simulink library "Centralized_I_Lib_Controller"  (R2024b)
(part 3 of 7)

[dq1,dq2,dq3,dq4,dq5,dq6,t10,t100,t1001,t1002,t1003,t1004,t1005,t1006,t1007,t1009,t101,t1010,t1011,t1013,t1016,t1018,t1019,t102,t1022,t1023,t1025,t1027,t1029,t1030,t1033,t1034,t1035,t1037,t1039,t104,t1041,t1042,t1043,t1047,t1048,t105,t1050,t1051,t1053,t1055,t1056,t1058,t1059,t106,t1060,t1061,t1062,t1063,t1065,t1067,t1068,t107,t1072,t1073,t1074,t1076,t1077,t1078,t108,t1080,t1081,t1082,t1083,t1084,t1085,t1086,t1087,t1088,t1089,t109,t1090,t1091,t1092,t1095,t1096,t1098,t1099,t11,t110,t1100,t1101,t1102,t1103,t1104,t1105,t1106,t1107,t1108,t111,t1110,t1111,t1112,t1113,t1114,t1116,t1117,t1119,t112,t1120,t1122,t1123,t1124,t1127,t113,t1131,t1132,t1133,t1134,t1135,t114,t1141,t1144,t1145,t1147,t1148,t1149,t1151,t1158,t1159,t116,t1160,t1161,t1162,t1163,t1164,t1165,t1166,t1167,t1169,t1170,t1171,t1172,t1173,t1176,t1177,t1178,t118,t1180,t1182,t1183,t1186,t1188,t1189,t119,t1190,t1191,t1192,t1193,t1194,t1195,t1196,t1198,t1199,t12,t120,t1201,t1202,t1203,t1204,t1205,t1207,t1208,t1210,t1211,t1212,t1214,t1215,t1216,t1217,t1218,t1219,t1220,t1221,t1222,t1224,t1227,t1228,t1229,t123,t1230,t1231,t1233,t1234,t1235,t1239,t124,t1240,t1241,t1242,t1243,t1244,t1245,t1246,t1247,t125,t1254,t1255,t1256,t126,t1263,t1266,t127,t128,t1283,t1286,t1287,t1288,t1289,t129,t1291,t1293,t1295,t1296,t1297,t1298,t1299,t13,t130,t131,t1316,t1317,t1319,t132,t1320,t1323,t1324,t1325,t1326,t1327,t1328,t1329,t133,t1331,t1332,t1333,t1334,t1335,t1345,t1346,t1347,t1349,t135,t1352,t1353,t1355,t1356,t1357,t1358,t1359,t1361,t1362,t1363,t1366,t1369,t137,t1370,t1371,t1372,t1373,t1375,t1376,t1377,t1379,t138,t1380,t1383,t1385,t1386,t1387,t1388,t139,t1390,t1391,t1392,t1393,t1395,t1397,t1398,t1399,t140,t1400,t1401,t1402,t1403,t1404,t1406,t1407,t1408,t1409,t141,t1410,t1413,t1416,t1417,t1419,t142,t1423,t1424,t1426,t1427,t1429,t143,t1432,t1433,t1434,t1435,t1438,t1441,t1442,t1443,t1445,t1447,t1450,t1452,t1453,t1456,t1457,t1458,t1462,t1463,t1464,t1465,t1466,t1467,t1468,t1469,t1470,t1473,t1475,t1476,t1477,t1479,t1480,t1481,t1482,t1483,t1484,t1487,t1488,t1489,t1490,t1491,t1493,t1494,t1495,t1496,t1497,t1498,t1499,t1500,t1502,t1503,t1504,t1505,t1511,t1513,t1523,t1524,t1525,t1526,t1528,t1530,t1531,t1532,t1533,t1534,t1536,t1537,t1538,t1539,t1540,t1541,t1544,t1545,t1546,t1554,t1555,t1556,t1557,t1558,t1562,t1563,t1564,t1566,t1567,t1568,t1571,t1575,t1576,t158,t1581,t1582,t1584,t1585,t1586,t1587,t1589,t159,t1590,t1591,t1592,t1593,t1595,t1597,t1598,t1599,t160,t1600,t1601,t1602,t1603,t1604,t1605,t1606,t1607,t1608,t1609,t161,t1610,t1611,t1612,t1613,t1614,t1618,t1619,t162,t1620,t1621,t1623,t1624,t1626,t1627,t1628,t1629,t163,t1630,t1631,t1632,t1633,t1634,t1635,t1637,t164,t1643,t165,t1654,t1655,t1656,t1657,t166,t1660,t1661,t1662,t1663,t1664,t1665,t1666,t1668,t1669,t167,t1670,t1671,t1673,t1675,t1676,t1677,t168,t1681,t1682,t1684,t1685,t1686,t1688,t1689,t1690,t1691,t1692,t1695,t1696,t1697,t1698,t170,t1700,t1701,t1702,t1703,t1704,t1705,t1706,t1709,t171,t1711,t1713,t1714,t1715,t1716,t1717,t1718,t1719,t1720,t1721,t1722,t1723,t1724,t1726,t1727,t1728,t173,t1730,t1732,t1734,t1736,t1739,t1741,t1742,t1747,t1748,t1749,t1750,t1752,t1753,t1754,t1755,t1756,t1758,t1759,t1760,t1761,t1763,t1764,t1765,t1766,t1767,t1768,t177,t1772,t1773,t1776,t1778,t1779,t178,t1780,t1781,t1782,t1785,t1786,t1787,t179,t1794,t1796,t18,t180,t1800,t1801,t1802,t1803,t1804,t1805,t1806,t1808,t181,t1815,t1816,t1817,t1818,t1819,t182,t1820,t1821,t1822,t1823,t1827,t1828,t1829,t183,t1830,t1831,t1832,t1833,t1837,t1838,t1839,t184,t1840,t1844,t1845,t1847,t1849,t185,t1850,t1851,t1852,t1853,t1854,t1857,t1858,t1859,t186,t1860,t1861,t1862,t1866,t1867,t1868,t1869,t187,t1870,t1871,t1872,t1873,t1874,t1875,t1876,t1877,t1878,t1879,t188,t1881,t1882,t1883,t1884,t1885,t1888,t1889,t189,t1890,t1893,t1895,t1896,t1897,t1898,t1899,t19,t1900,t1901,t1902,t1904,t1906,t1907,t191,t1911,t1913,t1917,t1919,t192,t1921,t1922,t1923,t1925,t1926,t1927,t193,t1931,t1936,t1937,t194,t1943,t1944,t1947,t1949,t195,t1950,t1952,t1953,t1954,t1955,t1956,t1957,t1958,t1959,t1962,t1964,t1965,t1966,t1967,t1970,t1971,t1973,t1974,t1975,t1976,t1977,t1978,t1980,t1981,t1982,t1983,t1984,t1985,t1986,t1987,t1988,t1990,t1991,t1992,t1993,t1994,t1997,t2,t20,t200,t2001,t2002,t2003,t2004,t2005,t2007,t2009,t201,t2010,t2014,t2015,t2017,t2018,t202,t2021,t2023,t2024,t2025,t2029,t203,t2030,t2031,t2034,t2035,t2036,t2037,t2038,t2039,t204,t2040,t2041,t2043,t2046,t2047,t2048,t2050,t2052,t2053,t2054,t2055,t2056,t2057,t2058,t2059,t206,t2061,t2063,t2064,t2065,t2066,t2067,t2068,t2069,t2070,t2071,t2072,t2073,t2075,t2077,t2078,t208,t2080,t2081,t2083,t2084,t2085,t2086,t2087,t2089,t209,t2090,t2091,t2092,t2093,t2094,t2096,t2097,t2098,t2099,t21,t210,t2106,t211,t2111,t2112,t2115,t2118,t212,t2121,t2124,t2125,t2126,t2128,t213,t2132,t2134,t2135,t2136,t2137,t2138,t2139,t214,t2140,t2141,t2144,t2145,t2148,t215,t2152,t2154,t2156,t2157,t2158,t2159,t216,t2160,t2161,t2162,t2163,t2165,t2167,t2169,t217,t2171,t2172,t2175,t2176,t2177,t2178,t2179,t218,t2180,t2181,t2182,t2183,t2184,t2185,t2186,t2187,t2188,t2189,t219,t2190,t2191,t2193,t2196,t2197,t2198,t2199,t22,t220,t2201,t2203,t2204,t2205,t2206,t2208,t221,t2212,t2213,t2214,t2215,t2216,t2217,t2219,t222,t2221,t2222,t2223,t2224,t2225,t2226,t2227,t2229,t223,t2231,t2232,t2233,t2235,t2236,t2237,t2238,t2239,t224,t2240,t2242,t2243,t2245,t2246,t2247,t2248,t2249,t225,t2250,t2251,t2252,t2253,t2254,t2256,t2258,t2259,t226,t2263,t2264,t2265,t2266,t2267,t2268,t2269,t227,t2277,t2278,t228,t2281,t2282,t2283,t2284,t2285,t2287,t2289,t229,t2290,t2292,t2293,t2296,t2297,t2299,t230,t2300,t2301,t231,t2310,t2312,t2313,t2314,t2319,t2322,t2323,t2324,t2326,t2327,t2329,t2330,t2331,t2332,t2333,t2334,t2338,t2339,t234,t2342,t2343,t2344,t235,t2356,t2357,t2358,t236,t2362,t2363,t2364,t2365,t2368,t2369,t237,t2370,t2371,t2372,t2374,t2376,t2378,t2379,t238,t2381,t2382,t2383,t2386,t2387,t239,t2390,t2391,t2392,t2394,t2395,t2396,t2397,t2398,t240,t2400,t2401,t2402,t2403,t2405,t2408,t2409,t241,t2410,t2412,t2413,t2414,t2416,t2417,t2418,t2419,t242,t2421,t2422,t2423,t2424,t2425,t2426,t2427,t2428,t2429,t243,t2430,t2431,t2432,t2433,t2436,t2437,t2438,t2439,t244,t2440,t2449,t245,t2450,t2451,t2452,t2453,t2454,t2455,t2456,t2457,t2459,t246,t2464,t2465,t2466,t2467,t2468,t2469,t247,t2470,t2471,t2472,t2473,t2474,t2475,t2476,t2477,t2478,t2479,t248,t2481,t2482,t2483,t2484,t2485,t2486,t2487,t2488,t249,t2491,t2492,t2494,t2495,t2496,t2498,t25,t250,t2504,t2508,t251,t2511,t2512,t2513,t2514,t2515,t2516,t2517,t2518,t252,t2520,t2523,t2524,t2525,t2527,t2529,t253,t2531,t2534,t2536,t2537,t2538,t2541,t2542,t2546,t2547,t2548,t255,t2550,t2552,t2553,t2554,t2555,t2556,t2557,t2559,t256,t2560,t2563,t2564,t2565,t2566,t2567,t2568,t2569,t2570,t2571,t2572,t2573,t2574,t2575,t2576,t2577,t2578,t2579,t2580,t2581,t2582,t2583,t2585,t2586,t2587,t2588,t259,t2591,t2593,t2594,t2595,t2596,t2597,t2598,t2599,t26,t260,t2600,t2601,t2602,t2603,t2604,t2605,t2607,t2608,t2609,t261,t2610,t2611,t2614,t2615,t2616,t2617,t262,t2622,t2623,t2625,t2628,t2629,t263,t2631,t2632,t2634,t2636,t2638,t2644,t2646,t2649,t265,t2650,t2652,t2659,t2660,t2661,t2665,t2666,t2667,t2668,t2669,t267,t2670,t2671,t2672,t2673,t2674,t2675,t2679,t2681,t2682,t2683,t2685,t2686,t2689,t269,t2692,t2694,t2696,t2697,t2698,t27,t270,t2700,t2701,t2702,t2703,t2705,t2706,t2707,t2711,t272,t2723,t2724,t2725,t2726,t2727,t2729,t273,t2730,t2731,t2732,t2733,t2734,t2735,t2736,t2738,t2739,t274,t2740,t2741,t2742,t2744,t2745,t2746,t2747,t2748,t2749,t275,t2751,t2752,t2753,t2754,t2755,t2756,t2757,t2758,t2759,t276,t2762,t2763,t2764,t2765,t2766,t2767,t2769,t277,t2770,t2771,t2776,t2778,t2779,t278,t2780,t2782,t2784,t2785,t2786,t2788,t279,t2792,t2793,t2795,t28,t280,t2800,t2802,t2803,t2804,t2806,t2807,t2809,t281,t2810,t2812,t2813,t2814,t2815,t2819,t2820,t2821,t2822,t2825,t2827,t2828,t2829,t283,t2830,t2832,t2833,t2834,t2836,t2839,t284,t2842,t2843,t2844,t285,t2850,t2854,t2858,t286,t2860,t2862,t2864,t2865,t2866,t2867,t2869,t287,t2870,t2871,t2872,t2873,t2877,t288,t2880,t2882,t2883,t2885,t2887,t2888,t289,t2890,t2891,t2892,t2899,t29,t290,t2900,t2901,t2902,t2903,t2904,t2905,t2906,t2911,t2912,t2913,t2916,t2919,t292,t2921,t2922,t2923,t2924,t2925,t2926,t2927,t2928,t2929,t293,t2930,t2931,t2932,t2933,t2934,t2935,t2937,t2938,t2939,t294,t2940,t2942,t2943,t2944,t2945,t2946,t2947,t2948,t2949,t295,t2950,t2951,t2952,t2953,t2954,t2956,t2957,t2959,t296,t2960,t2962,t2964,t2965,t2966,t2967,t2968,t297,t2970,t2973,t2974,t2975,t2977,t2978,t2979,t298,t2981,t2983,t2984,t2986,t2988,t299,t2991,t2995,t2997,t2998,t3,t300,t3002,t3003,t3004,t3006,t3007,t301,t3010,t3011,t3012,t3013,t3015,t3016,t3017,t302,t3020,t3021,t3023,t3025,t3028,t303,t3034,t3035,t3036,t3037,t304,t3040,t3042,t3046,t3047,t3049,t305,t3051,t3052,t3053,t3054,t3056,t3057,t3058,t3059,t306,t3060,t3061,t3062,t3064,t3065,t3066,t3067,t3068,t3069,t307,t3070,t3071,t3072,t3073,t3074,t3075,t3076,t3077,t3078,t3079,t308,t3080,t3081,t3082,t3083,t3085,t3087,t3088,t309,t3091,t3092,t3093,t3094,t3095,t3096,t3097,t3099,t3100,t3101,t3102,t3103,t3104,t3107,t3108,t3109,t311,t3110,t3111,t3112,t3118,t312,t3126,t3128,t313,t3131,t3132,t3133,t3134,t3135,t3138,t3139,t314,t3140,t3142,t3143,t3146,t3147,t3148,t315,t3156,t316,t3160,t3161,t3162,t3163,t3164,t3167,t3168,t317,t3170,t3175,t318,t3182,t3185,t3187,t3188,t3189,t319,t3190,t3192,t3193,t3196,t3197,t3198,t3199,t320,t3200,t3203,t3204,t3205,t3206,t3207,t3208,t3209,t321,t3210,t3211,t3212,t3213,t3214,t3215,t3216,t3217,t3218,t3219,t322,t3220,t3221,t3222,t3223,t3224,t3225,t3226,t3227,t3228,t323,t3230,t3231,t3232,t3234,t324,t3245,t3246,t325,t326,t3262,t327,t3272,t328,t329,t3298,t3299,t330,t331,t332,t3320,t3326,t333,t3330,t334,t336,t337,t338,t3388,t339,t3396,t341,t342,t343,t344,t345,t3453,t346,t347,t3470,t3471,t3473,t3479,t348,t3480,t3483,t3484,t3485,t3486,t349,t3490,t3491,t3497,t3498,t350,t3501,t3510,t3511,t352,t3521,t3526,t3527,t3528,t3529,t353,t354,t3546,t3547,t3549,t355,t3551,t3559,t356,t3560,t3562,t357,t358,t3589,t3590,t3592,t3593,t3594,t3595,t360,t3608,t3609,t3611,t3612,t3613,t3614,t3615,t3616,t3617,t3627,t3628,t3629,t3630,t3635,t3636,t3637,t364,t3648,t365,t3650,t3651,t367,t368,t3680,t3687,t3690,t3691,t3692,t3704,t3705,t371,t3722,t3723,t3724,t3725,t3726,t373,t375,t376,t377,t3779,t378,t379,t3796,t380,t381,t3811,t382,t3822,t3823,t3824,t3827,t3828,t383,t3839,t384,t385,t386,t3862,t3865,t3868,t387,t3871,t3872,t388,t3884,t389,t3909,t391,t3910,t392,t3932,t3935,t3941,t396,t3960,t3963,t397,t399,t4,t400,t401,t402,t4031,t404,t4042,t4043,t4046,t4047,t405,t4057,t406,t4060,t4061,t4067,t407,t4075,t408,t409,t410,t4103,t4109,t411,t412,t413,t414,t415,t416,t4168,t417,t4174,t418,t419,t420,t4204,t4208,t4209,t421,t4212,t422,t423,t424,t425,t426,t4260,t4261,t4262,t4263,t4265,t427,t4280,t429,t430,t431,t432,t433,t434,t4344,t4345,t4347,t435,t436,t437,t4372,t438,t439,t440,t441,t442,t443,t444,t4451,t4452,t4456,t4457,t4475,t4477,t4478,t450,t4508,t451,t453,t4539,t454,t4542,t4544,t4545,t4546,t4547,t456,t4565,t4566,t4568,t4579,t458,t4581,t4584,t459,t460,t461,t462,t463,t464,t465,t467,t468,t469,t470,t471,t472,t473,t474,t475,t476,t4763,t4765,t4766,t4768,t4769,t477,t4770,t4771,t4773,t478,t479,t48,t480,t4806,t4808,t481,t482,t483,t4830,t4831,t4833,t484,t486,t487,t488,t489,t4895,t4898,t49,t490,t4900,t491,t492,t494,t495,t496,t497,t498,t499,t5,t50,t500,t501,t502,t5041,t5054,t5055,t509,t51,t510,t5103,t511,t512,t513,t514,t515,t516,t517,t5175,t5176,t518,t519,t52,t520,t521,t522,t523,t524,t527,t528,t5280,t529,t53,t530,t531,t534,t5343,t5344,t535,t5354,t5356,t536,t5361,t539,t54,t540,t5411,t542,t543,t545,t546,t547,t548,t5491,t5492,t55,t550,t551,t552,t553,t5551,t5552,t556,t557,t558,t559,t56,t560,t561,t5613,t562,t563,t565,t566,t567,t569,t57,t574,t58,t582,t585,t589,t59,t590,t592,t594,t595,t597,t598,t599,t6,t60,t600,t601,t602,t6023,t604,t605,t606,t608,t609,t61,t610,t611,t613,t614,t616,t617,t62,t624,t63,t630,t632,t635,t636,t641,t643,t644,t645,t647,t6473,t648,t649,t650,t651,t652,t653,t654,t655,t656,t657,t658,t66,t660,t661,t663,t664,t666,t667,t669,t67,t670,t6734,t6735,t6736,t674,t6742,t6743,t6744,t6745,t675,t6754,t6755,t676,t677,t6772,t678,t679,t680,t681,t683,t684,t685,t686,t687,t688,t689,t690,t691,t692,t693,t696,t699,t7,t700,t702,t703,t704,t705,t706,t708,t711,t713,t715,t716,t717,t719,t720,t721,t722,t723,t725,t726,t729,t731,t732,t734,t737,t738,t742,t744,t748,t750,t751,t754,t756,t758,t759,t761,t763,t766,t767,t768,t769,t770,t773,t774,t775,t776,t781,t782,t784,t785,t788,t789,t790,t793,t795,t796,t798,t799,t8,t800,t803,t805,t807,t808,t809,t81,t814,t815,t816,t817,t819,t82,t820,t821,t822,t823,t824,t826,t828,t829,t83,t831,t832,t833,t834,t835,t837,t838,t839,t84,t842,t844,t847,t848,t849,t85,t850,t851,t852,t853,t854,t858,t859,t86,t861,t863,t864,t867,t868,t87,t871,t872,t875,t879,t88,t880,t883,t884,t885,t886,t888,t89,t890,t891,t894,t895,t896,t897,t898,t899,t9,t90,t900,t902,t905,t906,t907,t908,t909,t910,t911,t912,t913,t914,t915,t916,t918,t919,t92,t920,t921,t923,t926,t928,t929,t93,t930,t931,t933,t934,t935,t936,t937,t938,t944,t945,t946,t947,t948,t949,t95,t950,t951,t954,t955,t956,t957,t958,t959,t96,t960,t961,t962,t963,t964,t965,t966,t967,t968,t969,t97,t970,t972,t973,t974,t975,t976,t977,t978,t98,t981,t982,t984,t986,t987,t988,t99,t990,t991,t992,t993,t994,t996,t997,t999] = ct{:};
t3240 = t12.*t204.*2.98328125e-2;
t3241 = t58.*t127.*2.98328125e-2;
t3247 = t28.*t2223;
t3249 = t28.*t2225;
t3250 = t28.*t2226;
t3251 = t22.*t2232;
t3252 = t22.*t2233;
t3257 = t58.*t86.*2.98328125e-2;
t3258 = t7.*t13.*t20.*t97.*1.1015625e-2;
t3260 = t98.*t1867;
t3271 = t22.*t62.*t97.*1.1015625e-2;
t3273 = t7.*t13.*t19.*t111.*1.1015625e-2;
t3274 = t7.*t13.*t20.*t109.*1.1015625e-2;
t3275 = t7.*t13.*t20.*t110.*1.1015625e-2;
t3276 = t6.*t12.*t19.*t101.*1.865e-2;
t3277 = t6.*t12.*t19.*t102.*1.865e-2;
t3279 = t20.*t62.*t97.*1.865e-2;
t3283 = t12.*t194.*t1009;
t3284 = t58.*t111.*t1009;
t3286 = t58.*t113.*t1009;
t3301 = t6.*t12.*t19.*t118.*1.865e-2;
t3302 = t8.*t12.*t19.*t112.*1.865e-2;
t3303 = t54.*t126.*t1009;
t3304 = t12.*t204.*t1009;
t3305 = t58.*t127.*t1009;
t3307 = t125.*t1869;
t3308 = t126.*t1869;
t3313 = t6.*t12.*t19.*t83.*1.865e-2;
t3314 = t29.*t54.*t126.*5.5078125e-3;
t3315 = t58.*t86.*t1009;
t3322 = t56.*t63.*t107.*5.5078125e-3;
t3323 = t62.*t63.*t97.*5.5078125e-3;
t3324 = t4.*t7.*t63.*t123.*5.5078125e-3;
t3327 = t7.*t12.*t63.*t112.*5.5078125e-3;
t3328 = t7.*t12.*t63.*t114.*5.5078125e-3;
t3329 = t5.*t2825;
t3332 = t4.*t13.*t49.*t1747;
t3333 = t4.*t7.*t54.*t1747;
t3334 = t7.*t107.*t1747;
t3335 = t12.*t194.*t1323;
t3336 = t111.*t2064;
t3341 = t7.*t204.*t1323;
t3342 = t113.*t2064;
t3343 = t97.*t2078;
t3344 = t107.*t2071;
t3345 = t109.*t2070;
t3346 = t12.*t99.*t1748;
t3347 = t110.*t2070;
t3348 = t108.*t2071;
t3353 = t112.*t2071;
t3358 = t3.*t4.*t13.*t346.*(-9.0./1.6e+2);
t3359 = t7.*t57.*t346.*(-9.0./3.2e+2);
t3360 = t5.*t6.*t13.*t346.*(-9.0./3.2e+2);
t3361 = t5.*t7.*t12.*t346.*(-9.0./3.2e+2);
t3363 = t7.*t58.*t346.*(9.0./8.0e+2);
t3370 = t13.*t50.*t346.*5.625e-3;
t3373 = t13.*t51.*t346.*5.625e-3;
t3380 = t13.*t50.*t346.*1.6875e-2;
t3381 = t5.*t7.*t10.*t346.*1.6875e-2;
t3382 = t13.*t51.*t346.*1.6875e-2;
t3383 = t7.*t57.*t346.*1.6875e-2;
t3384 = t7.*t58.*t346.*1.6875e-2;
t3386 = t5.*t7.*t12.*t346.*1.6875e-2;
t3391 = t20.*t21.*t1747;
t3395 = t20.*t2478;
t3397 = t11.*t13.*t63.*t113.*5.5078125e-3;
t3399 = t13.*t109.*t1747;
t3401 = t12.*t204.*t1323;
t3402 = t127.*t2064;
t3405 = t13.*t204.*t1323;
t3412 = t61.*t2371;
t3416 = t126.*t2071;
t3419 = t127.*t2071;
t3421 = t129.*t2071;
t3422 = t13.*t62.*t2053;
t3425 = t3.*t9.*t13.*t346.*(-9.0./1.6e+2);
t3427 = t4.*t9.*t13.*t346.*(-9.0./3.2e+2);
t3429 = t5.*t12.*t13.*t346.*(-9.0./3.2e+2);
t3430 = t5.*t11.*t13.*t346.*(9.0./8.0e+2);
t3433 = t13.*t54.*t346.*5.625e-3;
t3434 = t13.*t55.*t346.*5.625e-3;
t3436 = t13.*t56.*t346.*5.625e-3;
t3441 = t13.*t57.*t346.*5.625e-3;
t3442 = t13.*t58.*t346.*5.625e-3;
t3448 = t13.*t56.*t346.*1.6875e-2;
t3450 = t7.*t61.*t346.*1.6875e-2;
t3451 = t13.*t57.*t346.*1.6875e-2;
t3452 = t7.*t62.*t346.*1.6875e-2;
t3454 = -t3056;
t3455 = t11.*t13.*t63.*t127.*5.5078125e-3;
t3456 = t86.*t2064;
t3458 = t13.*t211.*t1323;
t3459 = t86.*t2071;
t3462 = t13.*t60.*t346.*5.625e-3;
t3463 = t13.*t62.*t346.*5.625e-3;
t3465 = t13.*t61.*t346.*1.6875e-2;
t3466 = t13.*t62.*t346.*1.6875e-2;
t3472 = t9.*t2900;
t3475 = t13.*t215.*t1323;
t3478 = t7.*t13.*t60.*t195.*2.203125e-2;
t3481 = t111.*t2092;
t3487 = t19.*t22.*t111.*(-5.5078125e-3);
t3488 = t109.*t2094;
t3489 = t110.*t2094;
t3504 = t19.*t2343;
t3505 = t10.*t2935;
t3506 = t21.*t22.*t123.*(-2.75390625e-3);
t3507 = t21.*t22.*t124.*(-2.75390625e-3);
t3512 = t19.*t2357;
t3519 = t3.*t9.*t27.*t1720;
t3520 = t28.*t56.*t1720;
t3522 = t22.*t28.*t124.*(-2.75390625e-3);
t3523 = t210.*t1803;
t3525 = t3.*t2977;
t3531 = t6.*t7.*t12.*t2124;
t3533 = t107.*t2126;
t3535 = t3.*t4.*t2478;
t3536 = t21.*t50.*t1748;
t3538 = t20.*t2371;
t3541 = t5.*t11.*t22.*t1741;
t3544 = t18.*t2378;
t3545 = t18.*t2379;
t3548 = t18.*t2382;
t3554 = t7.*t18.*t346.*(-9.0./3.2e+2);
t3555 = t7.*t20.*t346.*(-9.0./3.2e+2);
t3557 = t62.*t194.*5.9665625e-2;
t3561 = t13.*t57.*t2124;
t3564 = t19.*t2391;
t3566 = t21.*t55.*t1748;
t3569 = t13.*t54.*t2125;
t3570 = t13.*t55.*t2125;
t3572 = t13.*t56.*t2125;
t3586 = t13.*t20.*t346.*(-9.0./1.6e+2);
t3587 = t13.*t20.*t346.*5.625e-3;
t3591 = -t3192;
t3596 = t18.*t2419;
t3598 = t12.*t13.*t20.*t1747;
t3605 = t13.*t27.*t346.*5.625e-3;
t3610 = t10.*t3011;
t3632 = t22.*t51.*t111.*(-5.5078125e-3);
t3634 = t21.*t49.*t104.*(-9.325e-3);
t3638 = t20.*t2430;
t3639 = t21.*t2431;
t3640 = t21.*t2432;
t3642 = -t3272;
t3643 = t22.*t56.*t107.*(-5.5078125e-3);
t3645 = t9.*t12.*t22.*t99.*(-5.5078125e-3);
t3646 = t11.*t12.*t22.*t99.*(-5.5078125e-3);
t3647 = t21.*t49.*t120.*(-9.325e-3);
t3652 = t21.*t2450;
t3653 = -t3299;
t3654 = t19.*t2454;
t3656 = t7.*t13.*t20.*t126.*(-5.5078125e-3);
t3657 = t7.*t13.*t18.*t129.*(-5.5078125e-3);
t3659 = t21.*t49.*t84.*(-9.325e-3);
t3660 = t7.*t12.*t63.*t97.*5.5078125e-3;
t3663 = t7.*t194.*t1323;
t3664 = t7.*t195.*t1323;
t3667 = t98.*t2071;
t3668 = t99.*t2071;
t3671 = t5.*t6.*t7.*t346.*(-9.0./3.2e+2);
t3678 = t7.*t50.*t346.*1.6875e-2;
t3679 = t7.*t51.*t346.*1.6875e-2;
t3681 = t19.*t2466;
t3682 = t3.*t19.*t2125;
t3686 = -t3320;
t3694 = t12.*t99.*t1925;
t3695 = t13.*t63.*t194.*(-2.75390625e-3);
t3696 = t13.*t63.*t195.*(-2.75390625e-3);
t3697 = t7.*t12.*t63.*t109.*(-2.75390625e-3);
t3698 = t12.*t99.*t1926;
t3699 = t109.*t2222;
t3700 = t110.*t2222;
t3701 = t111.*t2222;
t3702 = t113.*t2222;
t3703 = t114.*t2222;
t3708 = t12.*t25.*t99.*2.98328125e-2;
t3711 = t3.*t4.*t13.*t346.*(-5.625e-3);
t3712 = t7.*t54.*t346.*(-5.625e-3);
t3713 = t7.*t55.*t346.*(-5.625e-3);
t3714 = t7.*t56.*t346.*(-5.625e-3);
t3716 = t7.*t58.*t346.*(-5.625e-3);
t3717 = t5.*t6.*t13.*t346.*(-5.625e-3);
t3720 = -t3388;
t3721 = t26.*t2725;
t3727 = t26.*t2729;
t3728 = t27.*t2730;
t3729 = t27.*t2731;
t3730 = t28.*t2733;
t3731 = t13.*t86.*t346.*(9.0./3.2e+2);
t3732 = t13.*t87.*t346.*(9.0./3.2e+2);
t3736 = t13.*t108.*t1925;
t3737 = t7.*t125.*t1925;
t3738 = t13.*t63.*t202.*(-2.75390625e-3);
t3739 = t13.*t63.*t203.*(-2.75390625e-3);
t3740 = t13.*t63.*t204.*(-2.75390625e-3);
t3741 = t13.*t51.*t2231;
t3742 = t58.*t2597;
t3743 = t7.*t63.*t211.*(-2.75390625e-3);
t3744 = t13.*t111.*t1926;
t3745 = t13.*t112.*t1926;
t3747 = t125.*t2222;
t3748 = t58.*t2600;
t3749 = t54.*t2603;
t3750 = t128.*t2222;
t3751 = t130.*t2222;
t3758 = t3.*t10.*t13.*t346.*(-5.625e-3);
t3759 = t4.*t9.*t13.*t346.*(-5.625e-3);
t3763 = t6.*t9.*t13.*t346.*(-5.625e-3);
t3768 = t87.*t2222;
t3774 = t9.*t10.*t13.*t346.*(-5.625e-3);
t3776 = t11.*t12.*t13.*t346.*(-5.625e-3);
t3778 = t7.*t13.*t110.*t111.*1.1015625e-2;
t3780 = t13.*t63.*t215.*(-2.75390625e-3);
t3781 = t9.*t20.*t22.*t109.*1.1015625e-2;
t3782 = t54.*t2636;
t3793 = t7.*t13.*t107.*t126.*1.1015625e-2;
t3795 = t9.*t20.*t29.*t109.*1.1015625e-2;
t3806 = t3.*t13.*t20.*t346.*(9.0./3.2e+2);
t3810 = -t3510;
t3812 = t3.*t4.*t2727;
t3813 = t21.*t2557;
t3814 = t22.*t2557;
t3821 = t3.*t3204;
t3826 = t20.*t2569;
t3829 = t28.*t2557;
t3837 = -t3546;
t3838 = -t3547;
t3840 = -t3551;
t3841 = t19.*t54.*t1919;
t3856 = t7.*t21.*t346.*(-5.625e-3);
t3858 = t12.*t54.*t110.*2.98328125e-2;
t3860 = t111.*t130.*2.98328125e-2;
t3861 = t86.*t99.*2.98328125e-2;
t3863 = -t3560;
t3864 = -t3562;
t3869 = t10.*t3216;
t3885 = t27.*t2586;
t3908 = -t3594;
t3928 = t20.*t97.*t1620;
t3931 = t25.*t2614;
t3936 = t21.*t2632;
t3939 = t18.*t2636;
t3959 = t22.*t62.*t194.*1.1015625e-2;
t3962 = t12.*t20.*t58.*t100.*1.865e-2;
t3964 = t12.*t54.*t110.*t1009;
t3966 = t27.*t97.*t1620;
t3967 = t111.*t130.*t1009;
t3968 = t86.*t99.*t1009;
t3970 = t49.*t61.*t1870;
t3971 = t50.*t60.*t1870;
t3972 = t19.*t28.*t54.*t1009;
t3973 = t9.*t20.*t26.*t1476;
t3977 = t7.*t9.*t13.*t20.*t125.*1.1015625e-2;
t3979 = t12.*t20.*t51.*t82.*1.865e-2;
t3984 = t9.*t20.*t26.*t1487;
t3985 = t5.*t6.*t7.*t11.*t346.*(9.0./1.6e+2);
t3986 = t13.*t97.*t346.*(9.0./3.2e+2);
t3996 = t13.*t108.*t346.*(9.0./3.2e+2);
t3997 = t13.*t109.*t346.*(9.0./3.2e+2);
t3999 = t13.*t110.*t346.*(9.0./3.2e+2);
t4002 = t13.*t111.*t346.*(9.0./3.2e+2);
t4004 = t13.*t112.*t346.*(9.0./3.2e+2);
t4007 = t13.*t113.*t346.*(9.0./3.2e+2);
t4008 = t13.*t114.*t346.*(9.0./3.2e+2);
t4015 = t51.*t63.*t111.*(-2.75390625e-3);
t4016 = t49.*t2569;
t4018 = t97.*t2222;
t4019 = t98.*t2222;
t4023 = t12.*t18.*t99.*2.98328125e-2;
t4024 = t3.*t4.*t7.*t346.*(-5.625e-3);
t4026 = t7.*t50.*t346.*(-5.625e-3);
t4029 = t20.*t2727;
t4032 = t20.*t2729;
t4033 = t20.*t2730;
t4034 = t20.*t2731;
t4035 = t22.*t2730;
t4036 = t22.*t2732;
t4038 = t13.*t127.*t346.*(9.0./3.2e+2);
t4040 = t13.*t129.*t346.*(9.0./3.2e+2);
t4048 = t22.*t3016;
t4051 = t13.*t86.*t346.*5.625e-3;
t4052 = t13.*t87.*t346.*5.625e-3;
t4054 = t13.*t87.*t346.*1.6875e-2;
t4058 = t12.*t19.*t22.*t98.*(-5.5078125e-3);
t4059 = -t3779;
t4062 = t12.*t22.*t25.*t99.*(-5.5078125e-3);
t4063 = t7.*t13.*t56.*t203.*(-5.5078125e-3);
t4064 = t4.*t3510;
t4068 = t18.*t2786;
t4069 = t10.*t20.*t21.*t116.*(-9.325e-3);
t4072 = t7.*t21.*t63.*t107.*5.5078125e-3;
t4073 = t13.*t19.*t63.*t98.*5.5078125e-3;
t4074 = t9.*t3511;
t4077 = t51.*t63.*t1869;
t4078 = t4.*t21.*t49.*t1747;
t4079 = t49.*t56.*t2125;
t4081 = t49.*t56.*t2126;
t4084 = t4.*t13.*t49.*t2125;
t4085 = t12.*t97.*t2126;
t4087 = t12.*t98.*t2126;
t4090 = t12.*t99.*t2126;
t4096 = t5.*t7.*t21.*t346.*(9.0./8.0e+2);
t4104 = t54.*t2979;
t4105 = t13.*t108.*t2124;
t4106 = t7.*t21.*t63.*t123.*5.5078125e-3;
t4107 = t7.*t21.*t63.*t124.*5.5078125e-3;
t4113 = t49.*t61.*t2125;
t4115 = t21.*t60.*t2052;
t4116 = t49.*t61.*t2126;
t4152 = t4.*t13.*t20.*t346.*(-9.0./3.2e+2);
t4153 = t4.*t13.*t20.*t346.*(9.0./8.0e+2);
t4166 = t110.*t210.*5.9665625e-2;
t4167 = t86.*t195.*5.9665625e-2;
t4171 = t13.*t125.*t2124;
t4172 = t13.*t126.*t2124;
t4173 = t7.*t21.*t63.*t85.*5.5078125e-3;
t4175 = t29.*t109.*t1747;
t4176 = t55.*t61.*t2125;
t4178 = t55.*t61.*t2126;
t4183 = t29.*t112.*t1748;
t4188 = t12.*t130.*t2126;
t4198 = t4.*t13.*t27.*t346.*(-9.0./3.2e+2);
t4205 = t22.*t63.*t108.*(-1.376953125e-3);
t4206 = t22.*t63.*t109.*(-1.376953125e-3);
t4207 = t22.*t63.*t112.*(-1.376953125e-3);
t4210 = t19.*t2899;
t4211 = t19.*t2900;
t4213 = t20.*t2902;
t4219 = t62+t88+t114+t129;
t4221 = t9.*t58.*t111.*(-2.98328125e-2);
t4230 = t21.*t63.*t123.*(-1.376953125e-3);
t4231 = t21.*t63.*t124.*(-1.376953125e-3);
t4232 = t22.*t63.*t123.*(-1.376953125e-3);
t4233 = t29.*t63.*t109.*(-1.376953125e-3);
t4234 = t29.*t63.*t110.*(-1.376953125e-3);
t4235 = t29.*t63.*t111.*(-1.376953125e-3);
t4236 = t29.*t63.*t113.*(-1.376953125e-3);
t4237 = t29.*t63.*t114.*(-1.376953125e-3);
t4238 = -t3884;
t4240 = t27.*t2902;
t4252 = t28.*t63.*t124.*(-1.376953125e-3);
t4253 = t22.*t63.*t86.*(-1.376953125e-3);
t4257 = t20.*t97.*t1804;
t4258 = t18.*t50.*t2096;
t4259 = t29.*t63.*t87.*(-1.376953125e-3);
t4266 = t20.*t21.*t2035;
t4272 = t21.*t61.*t191.*(-1.865e-2);
t4274 = -t3963;
t4275 = t27.*t97.*t1804;
t4276 = t22.*t111.*t130.*(-5.5078125e-3);
t4277 = t22.*t86.*t99.*(-5.5078125e-3);
t4279 = t21.*t2942;
t4281 = t20.*t21.*t2046;
t4284 = t7.*t51.*t63.*t111.*5.5078125e-3;
t4285 = t21.*t50.*t214.*(-1.865e-2);
t4287 = t7.*t99.*t346.*(-9.0./3.2e+2);
t4288 = t7.*t97.*t346.*(9.0./8.0e+2);
t4293 = t4.*t7.*t49.*t346.*1.6875e-2;
t4294 = t7.*t97.*t346.*1.6875e-2;
t4295 = t7.*t99.*t346.*1.6875e-2;
t4298 = t7.*t62.*t63.*t97.*1.1015625e-2;
t4299 = t13.*t51.*t63.*t107.*5.5078125e-3;
t4300 = t7.*t11.*t12.*t63.*t99.*5.5078125e-3;
t4301 = t63.*t99.*t1621;
t4311 = t7.*t108.*t346.*(-9.0./3.2e+2);
t4312 = t7.*t11.*t50.*t346.*(-9.0./3.2e+2);
t4313 = t7.*t112.*t346.*(-9.0./3.2e+2);
t4315 = t7.*t10.*t51.*t346.*(9.0./8.0e+2);
t4322 = t13.*t97.*t346.*5.625e-3;
t4327 = t13.*t98.*t346.*5.625e-3;
t4331 = t13.*t99.*t346.*5.625e-3;
t4336 = t4.*t13.*t49.*t346.*1.6875e-2;
t4337 = t4.*t7.*t54.*t346.*1.6875e-2;
t4338 = t7.*t107.*t346.*1.6875e-2;
t4340 = t7.*t108.*t346.*1.6875e-2;
t4341 = t7.*t109.*t346.*1.6875e-2;
t4342 = t7.*t114.*t346.*1.6875e-2;
t4349 = t18.*t2978;
t4352 = t18.*t2979;
t4354 = t6.*t12.*t18.*t2124;
t4361 = t19.*t54.*t2125;
t4364 = t20.*t21.*t2063;
t4379 = t7.*t51.*t63.*t87.*1.1015625e-2;
t4381 = t62.*t63.*t194.*5.5078125e-3;
t4383 = t7.*t12.*t63.*t204.*5.5078125e-3;
t4384 = t7.*t58.*t63.*t127.*5.5078125e-3;
t4386 = t63.*t112.*t1621;
t4387 = t12.*t54.*t110.*t1323;
t4388 = t58.*t111.*t1747;
t4389 = t111.*t130.*t1323;
t4390 = t86.*t99.*t1323;
t4391 = t49.*t61.*t2071;
t4393 = t202.*t2071;
t4394 = t203.*t2071;
t4403 = t7.*t126.*t346.*(-9.0./3.2e+2);
t4405 = t7.*t127.*t346.*(-9.0./3.2e+2);
t4406 = t7.*t129.*t346.*(-9.0./3.2e+2);
t4407 = t5.*t7.*t62.*t346.*(-9.0./3.2e+2);
t4409 = t11.*t13.*t50.*t346.*(9.0./8.0e+2);
t4413 = t13.*t107.*t346.*5.625e-3;
t4416 = t13.*t108.*t346.*5.625e-3;
t4418 = t13.*t109.*t346.*5.625e-3;
t4420 = t13.*t110.*t346.*5.625e-3;
t4423 = t13.*t111.*t346.*5.625e-3;
t4426 = t13.*t112.*t346.*5.625e-3;
t4429 = t13.*t113.*t346.*5.625e-3;
t4430 = t13.*t114.*t346.*5.625e-3;
t4437 = t4.*t13.*t54.*t346.*1.6875e-2;
t4438 = t13.*t107.*t346.*1.6875e-2;
t4440 = t13.*t108.*t346.*1.6875e-2;
t4441 = t13.*t109.*t346.*1.6875e-2;
t4442 = t7.*t125.*t346.*1.6875e-2;
t4443 = t7.*t126.*t346.*1.6875e-2;
t4445 = t13.*t114.*t346.*1.6875e-2;
t4446 = t7.*t129.*t346.*1.6875e-2;
t4449 = t7.*t130.*t346.*1.6875e-2;
t4454 = t7.*t20.*t28.*t1747;
t4458 = t12.*t19.*t98.*(-2.98328125e-2);
t4461 = t13.*t49.*t63.*t86.*1.1015625e-2;
t4462 = t13.*t49.*t63.*t87.*5.5078125e-3;
t4463 = t13.*t50.*t63.*t86.*5.5078125e-3;
t4464 = t13.*t50.*t63.*t87.*5.5078125e-3;
t4466 = t13.*t204.*t1747;
t4471 = t211.*t2071;
t4474 = t22.*t3010;
t4476 = t20.*t3011;
t4479 = t22.*t3013;
t4482 = t7.*t86.*t346.*(-9.0./3.2e+2);
t4483 = t11.*t13.*t55.*t346.*(9.0./8.0e+2);
t4485 = t9.*t13.*t54.*t346.*(2.7e+1./8.0e+2);
t4486 = t13.*t123.*t346.*5.625e-3;
t4487 = t13.*t124.*t346.*5.625e-3;
t4489 = t13.*t125.*t346.*5.625e-3;
t4490 = t13.*t126.*t346.*5.625e-3;
t4493 = t13.*t127.*t346.*5.625e-3;
t4494 = t13.*t128.*t346.*5.625e-3;
t4496 = t13.*t129.*t346.*5.625e-3;
t4498 = t13.*t130.*t346.*5.625e-3;
t4501 = t13.*t123.*t346.*1.6875e-2;
t4503 = t13.*t124.*t346.*1.6875e-2;
t4504 = t13.*t125.*t346.*1.6875e-2;
t4506 = t13.*t130.*t346.*1.6875e-2;
t4507 = t7.*t87.*t346.*1.6875e-2;
t4511 = t215.*t2222;
t4517 = t9.*t13.*t62.*t346.*(-5.625e-3);
t4522 = t7.*t20.*t51.*t346.*(9.0./1.6e+2);
t4529 = t3.*t9.*t13.*t20.*t346.*(9.0./8.0e+1);
t4530 = t5.*t11.*t13.*t18.*t346.*(9.0./8.0e+1);
t4538 = t7.*t3822;
t4543 = t12.*t19.*t63.*t98.*(-2.75390625e-3);
t4557 = t6.*t7.*t20.*t346.*(-9.0./8.0e+2);
t4558 = t4.*t7.*t20.*t346.*(-5.625e-3);
t4562 = -t4103;
t4567 = t9.*t3824;
t4569 = t22.*t109.*t1925;
t4570 = t12.*t25.*t63.*t99.*(-2.75390625e-3);
t4572 = t6.*t19.*t2595;
t4573 = t13.*t20.*t63.*t109.*(-2.75390625e-3);
t4574 = t7.*t20.*t63.*t125.*(-2.75390625e-3);
t4576 = t7.*t20.*t63.*t126.*(-2.75390625e-3);
t4578 = t6.*t12.*t54.*t2324;
t4580 = t12.*t112.*t2324;
t4582 = t12.*t114.*t2324;
t4590 = t5.*t18.*t61.*t1919;
t4613 = t6.*t13.*t19.*t346.*(-5.625e-3);
t4616 = t5.*t13.*t21.*t346.*(-5.625e-3);
t4618 = t5.*t13.*t18.*t346.*(-1.6875e-2);
t4619 = t7.*t11.*t18.*t346.*(-1.6875e-2);
t4624 = t13.*t21.*t63.*t123.*(-2.75390625e-3);
t4626 = t13.*t21.*t63.*t124.*(-2.75390625e-3);
t4627 = t29.*t62.*t2212;
t4628 = t29.*t112.*t1926;
t4629 = t25.*t3078;
t4631 = t6.*t27.*t2600;
t4632 = t5.*t26.*t2603;
t4639 = t11.*t26.*t2583;
t4664 = t7.*t11.*t26.*t346.*(-5.625e-3);
t4673 = t10.*t13.*t25.*t346.*(-5.625e-3);
t4674 = t9.*t13.*t27.*t346.*(-5.625e-3);
t4675 = t12.*t13.*t27.*t346.*(-5.625e-3);
t4676 = t7.*t13.*t19.*t60.*t98.*1.1015625e-2;
t4685 = t22.*t110.*t210.*1.1015625e-2;
t4686 = t22.*t86.*t195.*1.1015625e-2;
t4694 = t7.*t11.*t99.*t346.*(9.0./1.6e+2);
t4702 = t7.*t18.*t20.*t346.*(9.0./1.6e+2);
t4705 = t7.*t11.*t112.*t346.*(9.0./1.6e+2);
t4711 = t7.*t51.*t62.*t346.*(9.0./4.0e+2);
t4713 = t4.*t7.*t49.*t346.*(-5.625e-3);
t4714 = t7.*t98.*t346.*(-5.625e-3);
t4715 = t7.*t99.*t346.*(-5.625e-3);
t4718 = t19.*t3192;
t4723 = t13.*t202.*t346.*(9.0./3.2e+2);
t4724 = t13.*t203.*t346.*(9.0./3.2e+2);
t4725 = t13.*t204.*t346.*(9.0./3.2e+2);
t4734 = t13.*t49.*t60.*t346.*(9.0./4.0e+2);
t4737 = t63.*t99.*t1805;
t4739 = t110.*t2566;
t4740 = t97.*t2600;
t4742 = t194.*t2222;
tau = ft_6({dq1,dq2,dq3,dq4,dq5,dq6,t10,t1001,t1002,t1003,t1004,t1005,t1006,t1007,t1009,t101,t1010,t1011,t1013,t1016,t1018,t1019,t102,t1022,t1023,t1025,t1027,t1029,t1030,t1033,t1034,t1035,t1037,t1039,t1041,t1042,t1043,t1047,t1048,t105,t1050,t1051,t1053,t1055,t1056,t1058,t1059,t106,t1060,t1061,t1062,t1063,t1065,t1067,t1068,t107,t1072,t1073,t1074,t1076,t1077,t1078,t108,t1080,t1081,t1082,t1083,t1084,t1085,t1086,t1087,t1088,t1089,t109,t1090,t1091,t1092,t1095,t1096,t1098,t1099,t11,t110,t1100,t1101,t1102,t1103,t1104,t1105,t1106,t1107,t1108,t111,t1110,t1111,t1112,t1113,t1114,t1116,t1117,t1119,t112,t1120,t1122,t1123,t1124,t1127,t113,t1131,t1132,t1133,t1134,t1135,t114,t1141,t1144,t1145,t1147,t1148,t1149,t1151,t1158,t1159,t1160,t1161,t1162,t1163,t1164,t1165,t1166,t1167,t1169,t1170,t1171,t1172,t1173,t1176,t1177,t1178,t1180,t1182,t1183,t1186,t1188,t1189,t119,t1190,t1191,t1192,t1193,t1194,t1195,t1196,t1198,t1199,t12,t120,t1201,t1202,t1203,t1204,t1205,t1207,t1208,t1210,t1211,t1212,t1214,t1215,t1216,t1217,t1218,t1219,t1220,t1221,t1222,t1224,t1227,t1228,t1229,t123,t1230,t1231,t1233,t1234,t1235,t1239,t124,t1240,t1241,t1242,t1243,t1244,t1245,t1246,t1247,t125,t1254,t1255,t1256,t126,t1263,t1266,t127,t128,t1283,t1286,t1287,t1288,t1289,t129,t1291,t1293,t1295,t1296,t1297,t1298,t1299,t13,t130,t131,t1316,t1317,t1319,t132,t1320,t1323,t1324,t1325,t1326,t1327,t1328,t1329,t133,t1331,t1332,t1333,t1334,t1335,t1345,t1346,t1347,t1349,t135,t1352,t1353,t1355,t1356,t1357,t1358,t1359,t1361,t1362,t1363,t1366,t1369,t137,t1370,t1371,t1372,t1373,t1375,t1376,t1377,t1379,t138,t1380,t1383,t1385,t1386,t1387,t1388,t139,t1390,t1391,t1392,t1393,t1395,t1397,t1398,t1399,t140,t1400,t1401,t1402,t1403,t1404,t1406,t1407,t1408,t1409,t141,t1410,t1413,t1416,t1417,t1419,t142,t1423,t1424,t1426,t1427,t1429,t143,t1432,t1433,t1434,t1435,t1438,t1441,t1442,t1443,t1445,t1447,t1450,t1452,t1453,t1456,t1457,t1458,t1462,t1463,t1464,t1465,t1466,t1467,t1468,t1469,t1470,t1473,t1475,t1477,t1479,t1480,t1481,t1482,t1483,t1484,t1488,t1489,t1490,t1491,t1493,t1494,t1495,t1496,t1497,t1498,t1499,t1500,t1502,t1503,t1504,t1505,t1511,t1513,t1523,t1524,t1525,t1526,t1528,t1530,t1531,t1532,t1533,t1534,t1536,t1537,t1538,t1539,t1540,t1541,t1544,t1545,t1546,t1554,t1555,t1556,t1557,t1558,t1562,t1563,t1564,t1566,t1567,t1568,t1571,t1575,t1576,t158,t1581,t1582,t1584,t1585,t1586,t1587,t1589,t159,t1590,t1591,t1592,t1593,t1595,t1597,t1598,t1599,t160,t1600,t1601,t1602,t1603,t1604,t1605,t1606,t1607,t1608,t1609,t161,t1610,t1611,t1612,t1613,t1614,t1618,t1619,t162,t1620,t1621,t1623,t1624,t1626,t1627,t1628,t1629,t163,t1630,t1631,t1632,t1633,t1634,t1635,t1637,t164,t1643,t165,t1654,t1655,t1656,t1657,t166,t1660,t1661,t1662,t1663,t1664,t1665,t1666,t1668,t1669,t167,t1670,t1671,t1673,t1675,t1676,t1677,t168,t1681,t1682,t1684,t1685,t1686,t1688,t1689,t1690,t1691,t1692,t1695,t1696,t1697,t1698,t170,t1700,t1701,t1702,t1703,t1704,t1705,t1706,t1709,t171,t1711,t1713,t1714,t1715,t1716,t1717,t1718,t1719,t1720,t1721,t1722,t1723,t1724,t1726,t1727,t1728,t173,t1730,t1732,t1734,t1736,t1739,t1741,t1742,t1747,t1749,t1750,t1752,t1753,t1754,t1755,t1756,t1758,t1759,t1760,t1761,t1763,t1764,t1765,t1766,t1767,t1768,t177,t1772,t1773,t1776,t1778,t1779,t178,t1780,t1781,t1782,t1785,t1786,t1787,t179,t1794,t1796,t18,t180,t1800,t1801,t1802,t1803,t1804,t1805,t1806,t1808,t181,t1815,t1816,t1817,t1818,t1819,t182,t1820,t1821,t1822,t1823,t1827,t1828,t1829,t183,t1830,t1831,t1832,t1833,t1837,t1838,t1839,t184,t1840,t1844,t1845,t1847,t1849,t185,t1850,t1851,t1852,t1853,t1854,t1857,t1858,t1859,t186,t1860,t1861,t1862,t1866,t1867,t1868,t1869,t187,t1870,t1871,t1872,t1873,t1874,t1875,t1876,t1877,t1878,t1879,t188,t1881,t1882,t1883,t1884,t1885,t1888,t1889,t189,t1890,t1893,t1895,t1896,t1897,t1898,t1899,t19,t1900,t1901,t1902,t1904,t1906,t1907,t191,t1911,t1913,t1917,t1919,t192,t1921,t1922,t1923,t1925,t1926,t1927,t193,t1931,t1936,t1937,t194,t1943,t1944,t1947,t1949,t195,t1950,t1952,t1953,t1954,t1955,t1956,t1957,t1958,t1959,t1962,t1964,t1965,t1966,t1967,t1970,t1971,t1973,t1974,t1975,t1976,t1977,t1978,t1980,t1981,t1982,t1983,t1984,t1985,t1986,t1987,t1988,t1990,t1991,t1992,t1993,t1994,t1997,t2,t20,t200,t2001,t2002,t2003,t2004,t2005,t2007,t2009,t201,t2010,t2014,t2015,t2017,t2018,t202,t2021,t2023,t2024,t2025,t2029,t203,t2030,t2031,t2034,t2035,t2036,t2037,t2038,t2039,t204,t2040,t2041,t2043,t2046,t2047,t2048,t2050,t2053,t2054,t2055,t2056,t2057,t2058,t2059,t206,t2061,t2063,t2064,t2065,t2066,t2067,t2068,t2069,t2070,t2071,t2072,t2073,t2075,t2077,t2078,t208,t2080,t2081,t2083,t2084,t2085,t2086,t2087,t2089,t209,t2090,t2091,t2092,t2093,t2094,t2096,t2097,t2098,t2099,t21,t210,t2106,t211,t2111,t2112,t2115,t2118,t212,t2121,t2124,t2125,t2126,t2128,t213,t2132,t2134,t2135,t2136,t2137,t2138,t2139,t214,t2140,t2141,t2144,t2145,t2148,t215,t2152,t2154,t2156,t2157,t2158,t2159,t216,t2160,t2161,t2162,t2163,t2165,t2167,t2169,t217,t2171,t2172,t2175,t2176,t2177,t2178,t2179,t218,t2180,t2181,t2182,t2183,t2184,t2185,t2186,t2187,t2188,t2189,t219,t2190,t2191,t2193,t2196,t2197,t2198,t2199,t22,t220,t2201,t2203,t2204,t2205,t2206,t2208,t221,t2212,t2213,t2214,t2215,t2216,t2217,t2219,t222,t2221,t2222,t2223,t2224,t2225,t2227,t2229,t223,t2231,t2232,t2233,t2235,t2236,t2237,t2238,t2239,t224,t2240,t2242,t2243,t2245,t2246,t2247,t2248,t2249,t225,t2250,t2251,t2252,t2253,t2254,t2256,t2258,t2259,t226,t2263,t2264,t2265,t2266,t2267,t2268,t2269,t227,t2277,t2278,t228,t2281,t2282,t2283,t2284,t2285,t2287,t2289,t229,t2290,t2292,t2293,t2296,t2297,t2299,t230,t2300,t2301,t231,t2310,t2312,t2313,t2314,t2319,t2322,t2323,t2324,t2326,t2327,t2329,t2330,t2331,t2332,t2333,t2334,t2338,t2339,t234,t2342,t2343,t2344,t235,t2356,t2357,t2358,t236,t2362,t2363,t2364,t2365,t2368,t2369,t237,t2370,t2372,t2374,t2376,t2378,t2379,t238,t2381,t2382,t2383,t2386,t2387,t239,t2390,t2392,t2394,t2395,t2396,t2397,t2398,t240,t2400,t2401,t2402,t2403,t2405,t2408,t2409,t241,t2410,t2412,t2413,t2414,t2416,t2417,t2418,t2419,t242,t2421,t2422,t2423,t2424,t2425,t2426,t2427,t2428,t2429,t243,t2430,t2431,t2432,t2433,t2436,t2437,t2438,t2439,t244,t2440,t2449,t245,t2450,t2451,t2452,t2453,t2454,t2455,t2456,t2457,t2459,t246,t2464,t2465,t2466,t2467,t2468,t2469,t247,t2470,t2471,t2472,t2473,t2474,t2475,t2476,t2477,t2478,t2479,t248,t2481,t2482,t2483,t2484,t2485,t2486,t2487,t2488,t249,t2491,t2492,t2494,t2495,t2496,t2498,t25,t250,t2504,t2508,t251,t2511,t2512,t2513,t2514,t2515,t2516,t2517,t2518,t252,t2520,t2523,t2524,t2525,t2527,t2529,t253,t2531,t2534,t2536,t2537,t2538,t2541,t2542,t2546,t2547,t2548,t255,t2550,t2552,t2553,t2554,t2555,t2556,t2559,t256,t2560,t2563,t2564,t2565,t2566,t2567,t2568,t2569,t2570,t2571,t2572,t2573,t2574,t2575,t2576,t2577,t2578,t2579,t2580,t2581,t2582,t2583,t2585,t2586,t2587,t2588,t259,t2591,t2593,t2594,t2595,t2596,t2597,t2598,t2599,t26,t260,t2600,t2601,t2602,t2603,t2604,t2605,t2607,t2608,t2609,t261,t2610,t2611,t2614,t2615,t2616,t2617,t262,t2622,t2623,t2625,t2628,t2629,t263,t2631,t2632,t2634,t2638,t2644,t2646,t2649,t265,t2650,t2652,t2659,t2660,t2661,t2665,t2666,t2667,t2668,t2669,t267,t2670,t2671,t2672,t2673,t2674,t2675,t2679,t2681,t2682,t2683,t2685,t2686,t2689,t269,t2692,t2694,t2696,t2697,t2698,t27,t270,t2700,t2701,t2702,t2703,t2705,t2706,t2707,t2711,t272,t2723,t2724,t2725,t2726,t2727,t2729,t273,t2730,t2732,t2733,t2734,t2735,t2736,t2738,t2739,t274,t2740,t2741,t2742,t2744,t2745,t2746,t2747,t2748,t2749,t275,t2751,t2752,t2753,t2754,t2755,t2756,t2757,t2758,t2759,t276,t2762,t2763,t2764,t2765,t2766,t2767,t2769,t277,t2770,t2771,t2776,t2778,t2779,t278,t2780,t2782,t2784,t2785,t2786,t2788,t279,t2792,t2793,t2795,t28,t280,t2800,t2802,t2803,t2804,t2806,t2807,t2809,t281,t2810,t2812,t2813,t2814,t2815,t2819,t2820,t2821,t2822,t2825,t2827,t2828,t2829,t283,t2830,t2832,t2833,t2834,t2836,t2839,t284,t2842,t2843,t2844,t285,t2850,t2854,t2858,t286,t2860,t2862,t2864,t2865,t2866,t2867,t2869,t287,t2870,t2871,t2872,t2873,t2877,t288,t2880,t2882,t2883,t2885,t2887,t2888,t289,t2890,t2891,t2892,t2899,t29,t290,t2900,t2901,t2902,t2903,t2904,t2905,t2906,t2911,t2912,t2913,t2916,t2919,t292,t2921,t2922,t2923,t2924,t2925,t2926,t2927,t2928,t2929,t293,t2930,t2931,t2932,t2933,t2934,t2935,t2937,t2938,t2939,t294,t2940,t2942,t2943,t2944,t2945,t2946,t2947,t2948,t2949,t295,t2950,t2951,t2952,t2953,t2954,t2956,t2957,t2959,t296,t2960,t2962,t2964,t2965,t2966,t2967,t2968,t297,t2970,t2973,t2974,t2975,t2977,t2978,t298,t2981,t2983,t2984,t2986,t2988,t299,t2991,t2995,t2997,t2998,t3,t300,t3002,t3003,t3004,t3006,t3007,t301,t3010,t3011,t3012,t3013,t3015,t3016,t3017,t302,t3020,t3021,t3023,t3025,t3028,t303,t3034,t3035,t3036,t3037,t304,t3040,t3042,t3046,t3047,t3049,t305,t3051,t3052,t3053,t3054,t3056,t3057,t3058,t3059,t306,t3060,t3061,t3062,t3064,t3065,t3066,t3067,t3068,t3069,t307,t3070,t3071,t3072,t3073,t3074,t3075,t3076,t3077,t3078,t3079,t308,t3080,t3081,t3082,t3083,t3085,t3087,t3088,t309,t3091,t3092,t3093,t3094,t3095,t3096,t3097,t3099,t3100,t3101,t3102,t3103,t3104,t3107,t3108,t3109,t311,t3110,t3111,t3112,t3118,t312,t3126,t3128,t313,t3131,t3132,t3133,t3134,t3135,t3138,t3139,t314,t3140,t3142,t3143,t3146,t3147,t3148,t315,t3156,t316,t3160,t3161,t3162,t3163,t3164,t3167,t3168,t317,t3170,t3175,t318,t3182,t3185,t3187,t3188,t3189,t319,t3190,t3192,t3193,t3196,t3197,t3198,t3199,t320,t3200,t3203,t3204,t3205,t3206,t3207,t3208,t3209,t321,t3210,t3211,t3212,t3213,t3214,t3215,t3216,t3217,t3218,t3219,t322,t3220,t3221,t3222,t3223,t3224,t3225,t3226,t3227,t3228,t323,t3230,t3231,t3232,t3234,t324,t3240,t3241,t3245,t3246,t3247,t3249,t325,t3250,t3251,t3252,t3257,t3258,t326,t3260,t3262,t327,t3271,t3273,t3274,t3275,t3276,t3277,t3279,t328,t3283,t3284,t3286,t329,t3298,t330,t3301,t3302,t3303,t3304,t3305,t3307,t3308,t331,t3313,t3314,t3315,t332,t3322,t3323,t3324,t3326,t3327,t3328,t3329,t333,t3330,t3332,t3333,t3334,t3335,t3336,t334,t3341,t3342,t3343,t3344,t3345,t3346,t3347,t3348,t3353,t3358,t3359,t336,t3360,t3361,t3363,t337,t3370,t3373,t338,t3380,t3381,t3382,t3383,t3384,t3386,t3388,t339,t3391,t3395,t3396,t3397,t3399,t3401,t3402,t3405,t341,t3412,t3416,t3419,t342,t3421,t3422,t3425,t3427,t3429,t343,t3430,t3433,t3434,t3436,t344,t3441,t3442,t3448,t345,t3450,t3451,t3452,t3453,t3454,t3455,t3456,t3458,t3459,t346,t3462,t3463,t3465,t3466,t347,t3470,t3471,t3472,t3473,t3475,t3478,t3479,t348,t3480,t3481,t3483,t3484,t3485,t3486,t3487,t3488,t3489,t349,t3490,t3491,t3497,t3498,t350,t3501,t3504,t3505,t3506,t3507,t3510,t3511,t3512,t3519,t352,t3520,t3521,t3522,t3523,t3525,t3526,t3527,t3528,t3529,t353,t3531,t3533,t3535,t3536,t3538,t354,t3541,t3544,t3545,t3548,t3549,t355,t3554,t3555,t3557,t3559,t356,t3561,t3564,t3566,t3569,t357,t3570,t3572,t358,t3586,t3587,t3589,t3590,t3591,t3592,t3593,t3595,t3596,t3598,t360,t3605,t3608,t3609,t3610,t3611,t3612,t3613,t3614,t3615,t3616,t3617,t3627,t3628,t3629,t3630,t3632,t3634,t3635,t3636,t3637,t3638,t3639,t364,t3640,t3642,t3643,t3645,t3646,t3647,t3648,t365,t3650,t3651,t3652,t3653,t3654,t3656,t3657,t3659,t3660,t3663,t3664,t3667,t3668,t367,t3671,t3678,t3679,t368,t3680,t3681,t3682,t3686,t3687,t3690,t3691,t3692,t3694,t3695,t3696,t3697,t3698,t3699,t3700,t3701,t3702,t3703,t3704,t3705,t3708,t371,t3711,t3712,t3713,t3714,t3716,t3717,t3720,t3721,t3722,t3723,t3724,t3725,t3726,t3727,t3728,t3729,t373,t3730,t3731,t3732,t3736,t3737,t3738,t3739,t3740,t3741,t3742,t3743,t3744,t3745,t3747,t3748,t3749,t375,t3750,t3751,t3758,t3759,t376,t3763,t3768,t377,t3774,t3776,t3778,t378,t3780,t3781,t3782,t379,t3793,t3795,t3796,t380,t3806,t381,t3810,t3811,t3812,t3813,t3814,t382,t3821,t3822,t3823,t3824,t3826,t3827,t3828,t3829,t383,t3837,t3838,t3839,t384,t3840,t3841,t385,t3856,t3858,t386,t3860,t3861,t3862,t3863,t3864,t3865,t3868,t3869,t387,t3871,t3872,t388,t3884,t3885,t389,t3908,t3909,t391,t3910,t392,t3928,t3931,t3932,t3935,t3936,t3939,t3941,t3959,t396,t3960,t3962,t3964,t3966,t3967,t3968,t397,t3970,t3971,t3972,t3973,t3977,t3979,t3984,t3985,t3986,t399,t3996,t3997,t3999,t4,t400,t4002,t4004,t4007,t4008,t401,t4015,t4016,t4018,t4019,t402,t4023,t4024,t4026,t4029,t4031,t4032,t4033,t4034,t4035,t4036,t4038,t404,t4040,t4042,t4043,t4046,t4047,t4048,t405,t4051,t4052,t4054,t4057,t4058,t4059,t406,t4060,t4061,t4062,t4063,t4064,t4067,t4068,t4069,t407,t4072,t4073,t4074,t4075,t4077,t4078,t4079,t408,t4081,t4084,t4085,t4087,t409,t4090,t4096,t410,t4103,t4104,t4105,t4106,t4107,t4109,t411,t4113,t4115,t4116,t412,t413,t414,t415,t4152,t4153,t416,t4166,t4167,t4168,t417,t4171,t4172,t4173,t4174,t4175,t4176,t4178,t418,t4183,t4188,t419,t4198,t420,t4204,t4205,t4206,t4207,t4208,t4209,t421,t4210,t4211,t4212,t4213,t4219,t422,t4221,t423,t4230,t4231,t4232,t4233,t4234,t4235,t4236,t4237,t4238,t424,t4240,t425,t4252,t4253,t4257,t4258,t4259,t426,t4260,t4261,t4262,t4263,t4265,t4266,t427,t4272,t4274,t4275,t4276,t4277,t4279,t4280,t4281,t4284,t4285,t4287,t4288,t429,t4293,t4294,t4295,t4298,t4299,t430,t4300,t4301,t431,t4311,t4312,t4313,t4315,t432,t4322,t4327,t433,t4331,t4336,t4337,t4338,t434,t4340,t4341,t4342,t4344,t4345,t4347,t4349,t435,t4352,t4354,t436,t4361,t4364,t437,t4372,t4379,t438,t4381,t4383,t4384,t4386,t4387,t4388,t4389,t439,t4390,t4391,t4393,t4394,t440,t4403,t4405,t4406,t4407,t4409,t441,t4413,t4416,t4418,t442,t4420,t4423,t4426,t4429,t443,t4430,t4437,t4438,t444,t4440,t4441,t4442,t4443,t4445,t4446,t4449,t4451,t4452,t4454,t4456,t4457,t4458,t4461,t4462,t4463,t4464,t4466,t4471,t4474,t4475,t4476,t4477,t4478,t4479,t4482,t4483,t4485,t4486,t4487,t4489,t4490,t4493,t4494,t4496,t4498,t450,t4501,t4503,t4504,t4506,t4507,t4508,t451,t4511,t4517,t4522,t4529,t453,t4530,t4538,t4539,t454,t4542,t4543,t4544,t4545,t4546,t4547,t4557,t4558,t456,t4562,t4565,t4566,t4567,t4568,t4569,t4570,t4572,t4573,t4574,t4576,t4578,t4579,t458,t4580,t4581,t4582,t4584,t459,t4590,t460,t461,t4613,t4616,t4618,t4619,t462,t4624,t4626,t4627,t4628,t4629,t463,t4631,t4632,t4639,t464,t465,t4664,t467,t4673,t4674,t4675,t4676,t468,t4685,t4686,t469,t4694,t470,t4702,t4705,t471,t4711,t4713,t4714,t4715,t4718,t472,t4723,t4724,t4725,t473,t4734,t4737,t4739,t474,t4740,t4742,t475,t476,t4763,t4765,t4766,t4768,t4769,t477,t4770,t4771,t4773,t478,t479,t48,t480,t4806,t4808,t481,t482,t483,t4830,t4831,t4833,t484,t486,t487,t488,t489,t4895,t4898,t49,t490,t4900,t491,t492,t494,t495,t496,t497,t498,t499,t5,t50,t500,t501,t502,t5041,t5054,t5055,t509,t51,t510,t5103,t511,t512,t513,t514,t515,t516,t517,t5175,t5176,t518,t519,t52,t520,t521,t522,t523,t524,t527,t528,t5280,t529,t53,t530,t531,t534,t5343,t5344,t535,t5354,t5356,t536,t5361,t539,t54,t540,t5411,t542,t543,t545,t546,t547,t548,t5491,t5492,t55,t550,t551,t552,t553,t5551,t5552,t556,t557,t558,t559,t56,t560,t561,t5613,t562,t563,t565,t566,t567,t569,t57,t574,t58,t582,t585,t589,t59,t590,t592,t594,t595,t597,t598,t599,t6,t60,t600,t601,t602,t6023,t604,t605,t606,t608,t609,t61,t610,t611,t613,t614,t616,t617,t62,t624,t63,t630,t632,t635,t636,t641,t643,t644,t645,t647,t6473,t648,t649,t650,t651,t652,t653,t654,t655,t656,t657,t658,t66,t660,t661,t663,t664,t666,t667,t669,t67,t670,t6734,t6735,t6736,t674,t6742,t6743,t6744,t6745,t675,t6754,t6755,t676,t677,t6772,t678,t679,t680,t681,t683,t684,t685,t686,t687,t688,t689,t690,t691,t692,t693,t696,t699,t7,t700,t702,t703,t704,t705,t706,t708,t711,t713,t715,t716,t717,t719,t720,t721,t722,t723,t725,t726,t729,t731,t732,t734,t737,t738,t742,t744,t748,t750,t751,t754,t756,t758,t759,t761,t763,t766,t767,t768,t769,t770,t773,t774,t775,t776,t781,t782,t784,t785,t788,t789,t790,t793,t795,t796,t798,t799,t8,t800,t803,t805,t807,t808,t809,t81,t814,t815,t816,t817,t819,t820,t821,t822,t823,t824,t826,t828,t829,t831,t832,t833,t834,t835,t837,t838,t839,t84,t842,t844,t847,t848,t849,t85,t850,t851,t852,t853,t854,t858,t859,t86,t861,t863,t864,t867,t868,t87,t871,t872,t875,t879,t880,t883,t884,t885,t886,t888,t89,t890,t891,t894,t895,t896,t897,t898,t899,t9,t90,t900,t902,t905,t906,t907,t908,t909,t910,t911,t912,t913,t914,t915,t916,t918,t919,t92,t920,t921,t923,t926,t928,t929,t93,t930,t931,t933,t934,t935,t936,t937,t938,t944,t945,t946,t947,t948,t949,t95,t950,t951,t954,t955,t956,t957,t958,t959,t96,t960,t961,t962,t963,t964,t965,t966,t967,t968,t969,t97,t970,t972,t973,t974,t975,t976,t977,t978,t98,t981,t982,t984,t986,t987,t988,t99,t990,t991,t992,t993,t994,t996,t997,t999});
end
function tau = ft_6(ct)
[dq1,dq2,dq3,dq4,dq5,dq6,t10,t1001,t1002,t1003,t1004,t1005,t1006,t1007,t1009,t101,t1010,t1011,t1013,t1016,t1018,t1019,t102,t1022,t1023,t1025,t1027,t1029,t1030,t1033,t1034,t1035,t1037,t1039,t1041,t1042,t1043,t1047,t1048,t105,t1050,t1051,t1053,t1055,t1056,t1058,t1059,t106,t1060,t1061,t1062,t1063,t1065,t1067,t1068,t107,t1072,t1073,t1074,t1076,t1077,t1078,t108,t1080,t1081,t1082,t1083,t1084,t1085,t1086,t1087,t1088,t1089,t109,t1090,t1091,t1092,t1095,t1096,t1098,t1099,t11,t110,t1100,t1101,t1102,t1103,t1104,t1105,t1106,t1107,t1108,t111,t1110,t1111,t1112,t1113,t1114,t1116,t1117,t1119,t112,t1120,t1122,t1123,t1124,t1127,t113,t1131,t1132,t1133,t1134,t1135,t114,t1141,t1144,t1145,t1147,t1148,t1149,t1151,t1158,t1159,t1160,t1161,t1162,t1163,t1164,t1165,t1166,t1167,t1169,t1170,t1171,t1172,t1173,t1176,t1177,t1178,t1180,t1182,t1183,t1186,t1188,t1189,t119,t1190,t1191,t1192,t1193,t1194,t1195,t1196,t1198,t1199,t12,t120,t1201,t1202,t1203,t1204,t1205,t1207,t1208,t1210,t1211,t1212,t1214,t1215,t1216,t1217,t1218,t1219,t1220,t1221,t1222,t1224,t1227,t1228,t1229,t123,t1230,t1231,t1233,t1234,t1235,t1239,t124,t1240,t1241,t1242,t1243,t1244,t1245,t1246,t1247,t125,t1254,t1255,t1256,t126,t1263,t1266,t127,t128,t1283,t1286,t1287,t1288,t1289,t129,t1291,t1293,t1295,t1296,t1297,t1298,t1299,t13,t130,t131,t1316,t1317,t1319,t132,t1320,t1323,t1324,t1325,t1326,t1327,t1328,t1329,t133,t1331,t1332,t1333,t1334,t1335,t1345,t1346,t1347,t1349,t135,t1352,t1353,t1355,t1356,t1357,t1358,t1359,t1361,t1362,t1363,t1366,t1369,t137,t1370,t1371,t1372,t1373,t1375,t1376,t1377,t1379,t138,t1380,t1383,t1385,t1386,t1387,t1388,t139,t1390,t1391,t1392,t1393,t1395,t1397,t1398,t1399,t140,t1400,t1401,t1402,t1403,t1404,t1406,t1407,t1408,t1409,t141,t1410,t1413,t1416,t1417,t1419,t142,t1423,t1424,t1426,t1427,t1429,t143,t1432,t1433,t1434,t1435,t1438,t1441,t1442,t1443,t1445,t1447,t1450,t1452,t1453,t1456,t1457,t1458,t1462,t1463,t1464,t1465,t1466,t1467,t1468,t1469,t1470,t1473,t1475,t1477,t1479,t1480,t1481,t1482,t1483,t1484,t1488,t1489,t1490,t1491,t1493,t1494,t1495,t1496,t1497,t1498,t1499,t1500,t1502,t1503,t1504,t1505,t1511,t1513,t1523,t1524,t1525,t1526,t1528,t1530,t1531,t1532,t1533,t1534,t1536,t1537,t1538,t1539,t1540,t1541,t1544,t1545,t1546,t1554,t1555,t1556,t1557,t1558,t1562,t1563,t1564,t1566,t1567,t1568,t1571,t1575,t1576,t158,t1581,t1582,t1584,t1585,t1586,t1587,t1589,t159,t1590,t1591,t1592,t1593,t1595,t1597,t1598,t1599,t160,t1600,t1601,t1602,t1603,t1604,t1605,t1606,t1607,t1608,t1609,t161,t1610,t1611,t1612,t1613,t1614,t1618,t1619,t162,t1620,t1621,t1623,t1624,t1626,t1627,t1628,t1629,t163,t1630,t1631,t1632,t1633,t1634,t1635,t1637,t164,t1643,t165,t1654,t1655,t1656,t1657,t166,t1660,t1661,t1662,t1663,t1664,t1665,t1666,t1668,t1669,t167,t1670,t1671,t1673,t1675,t1676,t1677,t168,t1681,t1682,t1684,t1685,t1686,t1688,t1689,t1690,t1691,t1692,t1695,t1696,t1697,t1698,t170,t1700,t1701,t1702,t1703,t1704,t1705,t1706,t1709,t171,t1711,t1713,t1714,t1715,t1716,t1717,t1718,t1719,t1720,t1721,t1722,t1723,t1724,t1726,t1727,t1728,t173,t1730,t1732,t1734,t1736,t1739,t1741,t1742,t1747,t1749,t1750,t1752,t1753,t1754,t1755,t1756,t1758,t1759,t1760,t1761,t1763,t1764,t1765,t1766,t1767,t1768,t177,t1772,t1773,t1776,t1778,t1779,t178,t1780,t1781,t1782,t1785,t1786,t1787,t179,t1794,t1796,t18,t180,t1800,t1801,t1802,t1803,t1804,t1805,t1806,t1808,t181,t1815,t1816,t1817,t1818,t1819,t182,t1820,t1821,t1822,t1823,t1827,t1828,t1829,t183,t1830,t1831,t1832,t1833,t1837,t1838,t1839,t184,t1840,t1844,t1845,t1847,t1849,t185,t1850,t1851,t1852,t1853,t1854,t1857,t1858,t1859,t186,t1860,t1861,t1862,t1866,t1867,t1868,t1869,t187,t1870,t1871,t1872,t1873,t1874,t1875,t1876,t1877,t1878,t1879,t188,t1881,t1882,t1883,t1884,t1885,t1888,t1889,t189,t1890,t1893,t1895,t1896,t1897,t1898,t1899,t19,t1900,t1901,t1902,t1904,t1906,t1907,t191,t1911,t1913,t1917,t1919,t192,t1921,t1922,t1923,t1925,t1926,t1927,t193,t1931,t1936,t1937,t194,t1943,t1944,t1947,t1949,t195,t1950,t1952,t1953,t1954,t1955,t1956,t1957,t1958,t1959,t1962,t1964,t1965,t1966,t1967,t1970,t1971,t1973,t1974,t1975,t1976,t1977,t1978,t1980,t1981,t1982,t1983,t1984,t1985,t1986,t1987,t1988,t1990,t1991,t1992,t1993,t1994,t1997,t2,t20,t200,t2001,t2002,t2003,t2004,t2005,t2007,t2009,t201,t2010,t2014,t2015,t2017,t2018,t202,t2021,t2023,t2024,t2025,t2029,t203,t2030,t2031,t2034,t2035,t2036,t2037,t2038,t2039,t204,t2040,t2041,t2043,t2046,t2047,t2048,t2050,t2053,t2054,t2055,t2056,t2057,t2058,t2059,t206,t2061,t2063,t2064,t2065,t2066,t2067,t2068,t2069,t2070,t2071,t2072,t2073,t2075,t2077,t2078,t208,t2080,t2081,t2083,t2084,t2085,t2086,t2087,t2089,t209,t2090,t2091,t2092,t2093,t2094,t2096,t2097,t2098,t2099,t21,t210,t2106,t211,t2111,t2112,t2115,t2118,t212,t2121,t2124,t2125,t2126,t2128,t213,t2132,t2134,t2135,t2136,t2137,t2138,t2139,t214,t2140,t2141,t2144,t2145,t2148,t215,t2152,t2154,t2156,t2157,t2158,t2159,t216,t2160,t2161,t2162,t2163,t2165,t2167,t2169,t217,t2171,t2172,t2175,t2176,t2177,t2178,t2179,t218,t2180,t2181,t2182,t2183,t2184,t2185,t2186,t2187,t2188,t2189,t219,t2190,t2191,t2193,t2196,t2197,t2198,t2199,t22,t220,t2201,t2203,t2204,t2205,t2206,t2208,t221,t2212,t2213,t2214,t2215,t2216,t2217,t2219,t222,t2221,t2222,t2223,t2224,t2225,t2227,t2229,t223,t2231,t2232,t2233,t2235,t2236,t2237,t2238,t2239,t224,t2240,t2242,t2243,t2245,t2246,t2247,t2248,t2249,t225,t2250,t2251,t2252,t2253,t2254,t2256,t2258,t2259,t226,t2263,t2264,t2265,t2266,t2267,t2268,t2269,t227,t2277,t2278,t228,t2281,t2282,t2283,t2284,t2285,t2287,t2289,t229,t2290,t2292,t2293,t2296,t2297,t2299,t230,t2300,t2301,t231,t2310,t2312,t2313,t2314,t2319,t2322,t2323,t2324,t2326,t2327,t2329,t2330,t2331,t2332,t2333,t2334,t2338,t2339,t234,t2342,t2343,t2344,t235,t2356,t2357,t2358,t236,t2362,t2363,t2364,t2365,t2368,t2369,t237,t2370,t2372,t2374,t2376,t2378,t2379,t238,t2381,t2382,t2383,t2386,t2387,t239,t2390,t2392,t2394,t2395,t2396,t2397,t2398,t240,t2400,t2401,t2402,t2403,t2405,t2408,t2409,t241,t2410,t2412,t2413,t2414,t2416,t2417,t2418,t2419,t242,t2421,t2422,t2423,t2424,t2425,t2426,t2427,t2428,t2429,t243,t2430,t2431,t2432,t2433,t2436,t2437,t2438,t2439,t244,t2440,t2449,t245,t2450,t2451,t2452,t2453,t2454,t2455,t2456,t2457,t2459,t246,t2464,t2465,t2466,t2467,t2468,t2469,t247,t2470,t2471,t2472,t2473,t2474,t2475,t2476,t2477,t2478,t2479,t248,t2481,t2482,t2483,t2484,t2485,t2486,t2487,t2488,t249,t2491,t2492,t2494,t2495,t2496,t2498,t25,t250,t2504,t2508,t251,t2511,t2512,t2513,t2514,t2515,t2516,t2517,t2518,t252,t2520,t2523,t2524,t2525,t2527,t2529,t253,t2531,t2534,t2536,t2537,t2538,t2541,t2542,t2546,t2547,t2548,t255,t2550,t2552,t2553,t2554,t2555,t2556,t2559,t256,t2560,t2563,t2564,t2565,t2566,t2567,t2568,t2569,t2570,t2571,t2572,t2573,t2574,t2575,t2576,t2577,t2578,t2579,t2580,t2581,t2582,t2583,t2585,t2586,t2587,t2588,t259,t2591,t2593,t2594,t2595,t2596,t2597,t2598,t2599,t26,t260,t2600,t2601,t2602,t2603,t2604,t2605,t2607,t2608,t2609,t261,t2610,t2611,t2614,t2615,t2616,t2617,t262,t2622,t2623,t2625,t2628,t2629,t263,t2631,t2632,t2634,t2638,t2644,t2646,t2649,t265,t2650,t2652,t2659,t2660,t2661,t2665,t2666,t2667,t2668,t2669,t267,t2670,t2671,t2672,t2673,t2674,t2675,t2679,t2681,t2682,t2683,t2685,t2686,t2689,t269,t2692,t2694,t2696,t2697,t2698,t27,t270,t2700,t2701,t2702,t2703,t2705,t2706,t2707,t2711,t272,t2723,t2724,t2725,t2726,t2727,t2729,t273,t2730,t2732,t2733,t2734,t2735,t2736,t2738,t2739,t274,t2740,t2741,t2742,t2744,t2745,t2746,t2747,t2748,t2749,t275,t2751,t2752,t2753,t2754,t2755,t2756,t2757,t2758,t2759,t276,t2762,t2763,t2764,t2765,t2766,t2767,t2769,t277,t2770,t2771,t2776,t2778,t2779,t278,t2780,t2782,t2784,t2785,t2786,t2788,t279,t2792,t2793,t2795,t28,t280,t2800,t2802,t2803,t2804,t2806,t2807,t2809,t281,t2810,t2812,t2813,t2814,t2815,t2819,t2820,t2821,t2822,t2825,t2827,t2828,t2829,t283,t2830,t2832,t2833,t2834,t2836,t2839,t284,t2842,t2843,t2844,t285,t2850,t2854,t2858,t286,t2860,t2862,t2864,t2865,t2866,t2867,t2869,t287,t2870,t2871,t2872,t2873,t2877,t288,t2880,t2882,t2883,t2885,t2887,t2888,t289,t2890,t2891,t2892,t2899,t29,t290,t2900,t2901,t2902,t2903,t2904,t2905,t2906,t2911,t2912,t2913,t2916,t2919,t292,t2921,t2922,t2923,t2924,t2925,t2926,t2927,t2928,t2929,t293,t2930,t2931,t2932,t2933,t2934,t2935,t2937,t2938,t2939,t294,t2940,t2942,t2943,t2944,t2945,t2946,t2947,t2948,t2949,t295,t2950,t2951,t2952,t2953,t2954,t2956,t2957,t2959,t296,t2960,t2962,t2964,t2965,t2966,t2967,t2968,t297,t2970,t2973,t2974,t2975,t2977,t2978,t298,t2981,t2983,t2984,t2986,t2988,t299,t2991,t2995,t2997,t2998,t3,t300,t3002,t3003,t3004,t3006,t3007,t301,t3010,t3011,t3012,t3013,t3015,t3016,t3017,t302,t3020,t3021,t3023,t3025,t3028,t303,t3034,t3035,t3036,t3037,t304,t3040,t3042,t3046,t3047,t3049,t305,t3051,t3052,t3053,t3054,t3056,t3057,t3058,t3059,t306,t3060,t3061,t3062,t3064,t3065,t3066,t3067,t3068,t3069,t307,t3070,t3071,t3072,t3073,t3074,t3075,t3076,t3077,t3078,t3079,t308,t3080,t3081,t3082,t3083,t3085,t3087,t3088,t309,t3091,t3092,t3093,t3094,t3095,t3096,t3097,t3099,t3100,t3101,t3102,t3103,t3104,t3107,t3108,t3109,t311,t3110,t3111,t3112,t3118,t312,t3126,t3128,t313,t3131,t3132,t3133,t3134,t3135,t3138,t3139,t314,t3140,t3142,t3143,t3146,t3147,t3148,t315,t3156,t316,t3160,t3161,t3162,t3163,t3164,t3167,t3168,t317,t3170,t3175,t318,t3182,t3185,t3187,t3188,t3189,t319,t3190,t3192,t3193,t3196,t3197,t3198,t3199,t320,t3200,t3203,t3204,t3205,t3206,t3207,t3208,t3209,t321,t3210,t3211,t3212,t3213,t3214,t3215,t3216,t3217,t3218,t3219,t322,t3220,t3221,t3222,t3223,t3224,t3225,t3226,t3227,t3228,t323,t3230,t3231,t3232,t3234,t324,t3240,t3241,t3245,t3246,t3247,t3249,t325,t3250,t3251,t3252,t3257,t3258,t326,t3260,t3262,t327,t3271,t3273,t3274,t3275,t3276,t3277,t3279,t328,t3283,t3284,t3286,t329,t3298,t330,t3301,t3302,t3303,t3304,t3305,t3307,t3308,t331,t3313,t3314,t3315,t332,t3322,t3323,t3324,t3326,t3327,t3328,t3329,t333,t3330,t3332,t3333,t3334,t3335,t3336,t334,t3341,t3342,t3343,t3344,t3345,t3346,t3347,t3348,t3353,t3358,t3359,t336,t3360,t3361,t3363,t337,t3370,t3373,t338,t3380,t3381,t3382,t3383,t3384,t3386,t3388,t339,t3391,t3395,t3396,t3397,t3399,t3401,t3402,t3405,t341,t3412,t3416,t3419,t342,t3421,t3422,t3425,t3427,t3429,t343,t3430,t3433,t3434,t3436,t344,t3441,t3442,t3448,t345,t3450,t3451,t3452,t3453,t3454,t3455,t3456,t3458,t3459,t346,t3462,t3463,t3465,t3466,t347,t3470,t3471,t3472,t3473,t3475,t3478,t3479,t348,t3480,t3481,t3483,t3484,t3485,t3486,t3487,t3488,t3489,t349,t3490,t3491,t3497,t3498,t350,t3501,t3504,t3505,t3506,t3507,t3510,t3511,t3512,t3519,t352,t3520,t3521,t3522,t3523,t3525,t3526,t3527,t3528,t3529,t353,t3531,t3533,t3535,t3536,t3538,t354,t3541,t3544,t3545,t3548,t3549,t355,t3554,t3555,t3557,t3559,t356,t3561,t3564,t3566,t3569,t357,t3570,t3572,t358,t3586,t3587,t3589,t3590,t3591,t3592,t3593,t3595,t3596,t3598,t360,t3605,t3608,t3609,t3610,t3611,t3612,t3613,t3614,t3615,t3616,t3617,t3627,t3628,t3629,t3630,t3632,t3634,t3635,t3636,t3637,t3638,t3639,t364,t3640,t3642,t3643,t3645,t3646,t3647,t3648,t365,t3650,t3651,t3652,t3653,t3654,t3656,t3657,t3659,t3660,t3663,t3664,t3667,t3668,t367,t3671,t3678,t3679,t368,t3680,t3681,t3682,t3686,t3687,t3690,t3691,t3692,t3694,t3695,t3696,t3697,t3698,t3699,t3700,t3701,t3702,t3703,t3704,t3705,t3708,t371,t3711,t3712,t3713,t3714,t3716,t3717,t3720,t3721,t3722,t3723,t3724,t3725,t3726,t3727,t3728,t3729,t373,t3730,t3731,t3732,t3736,t3737,t3738,t3739,t3740,t3741,t3742,t3743,t3744,t3745,t3747,t3748,t3749,t375,t3750,t3751,t3758,t3759,t376,t3763,t3768,t377,t3774,t3776,t3778,t378,t3780,t3781,t3782,t379,t3793,t3795,t3796,t380,t3806,t381,t3810,t3811,t3812,t3813,t3814,t382,t3821,t3822,t3823,t3824,t3826,t3827,t3828,t3829,t383,t3837,t3838,t3839,t384,t3840,t3841,t385,t3856,t3858,t386,t3860,t3861,t3862,t3863,t3864,t3865,t3868,t3869,t387,t3871,t3872,t388,t3884,t3885,t389,t3908,t3909,t391,t3910,t392,t3928,t3931,t3932,t3935,t3936,t3939,t3941,t3959,t396,t3960,t3962,t3964,t3966,t3967,t3968,t397,t3970,t3971,t3972,t3973,t3977,t3979,t3984,t3985,t3986,t399,t3996,t3997,t3999,t4,t400,t4002,t4004,t4007,t4008,t401,t4015,t4016,t4018,t4019,t402,t4023,t4024,t4026,t4029,t4031,t4032,t4033,t4034,t4035,t4036,t4038,t404,t4040,t4042,t4043,t4046,t4047,t4048,t405,t4051,t4052,t4054,t4057,t4058,t4059,t406,t4060,t4061,t4062,t4063,t4064,t4067,t4068,t4069,t407,t4072,t4073,t4074,t4075,t4077,t4078,t4079,t408,t4081,t4084,t4085,t4087,t409,t4090,t4096,t410,t4103,t4104,t4105,t4106,t4107,t4109,t411,t4113,t4115,t4116,t412,t413,t414,t415,t4152,t4153,t416,t4166,t4167,t4168,t417,t4171,t4172,t4173,t4174,t4175,t4176,t4178,t418,t4183,t4188,t419,t4198,t420,t4204,t4205,t4206,t4207,t4208,t4209,t421,t4210,t4211,t4212,t4213,t4219,t422,t4221,t423,t4230,t4231,t4232,t4233,t4234,t4235,t4236,t4237,t4238,t424,t4240,t425,t4252,t4253,t4257,t4258,t4259,t426,t4260,t4261,t4262,t4263,t4265,t4266,t427,t4272,t4274,t4275,t4276,t4277,t4279,t4280,t4281,t4284,t4285,t4287,t4288,t429,t4293,t4294,t4295,t4298,t4299,t430,t4300,t4301,t431,t4311,t4312,t4313,t4315,t432,t4322,t4327,t433,t4331,t4336,t4337,t4338,t434,t4340,t4341,t4342,t4344,t4345,t4347,t4349,t435,t4352,t4354,t436,t4361,t4364,t437,t4372,t4379,t438,t4381,t4383,t4384,t4386,t4387,t4388,t4389,t439,t4390,t4391,t4393,t4394,t440,t4403,t4405,t4406,t4407,t4409,t441,t4413,t4416,t4418,t442,t4420,t4423,t4426,t4429,t443,t4430,t4437,t4438,t444,t4440,t4441,t4442,t4443,t4445,t4446,t4449,t4451,t4452,t4454,t4456,t4457,t4458,t4461,t4462,t4463,t4464,t4466,t4471,t4474,t4475,t4476,t4477,t4478,t4479,t4482,t4483,t4485,t4486,t4487,t4489,t4490,t4493,t4494,t4496,t4498,t450,t4501,t4503,t4504,t4506,t4507,t4508,t451,t4511,t4517,t4522,t4529,t453,t4530,t4538,t4539,t454,t4542,t4543,t4544,t4545,t4546,t4547,t4557,t4558,t456,t4562,t4565,t4566,t4567,t4568,t4569,t4570,t4572,t4573,t4574,t4576,t4578,t4579,t458,t4580,t4581,t4582,t4584,t459,t4590,t460,t461,t4613,t4616,t4618,t4619,t462,t4624,t4626,t4627,t4628,t4629,t463,t4631,t4632,t4639,t464,t465,t4664,t467,t4673,t4674,t4675,t4676,t468,t4685,t4686,t469,t4694,t470,t4702,t4705,t471,t4711,t4713,t4714,t4715,t4718,t472,t4723,t4724,t4725,t473,t4734,t4737,t4739,t474,t4740,t4742,t475,t476,t4763,t4765,t4766,t4768,t4769,t477,t4770,t4771,t4773,t478,t479,t48,t480,t4806,t4808,t481,t482,t483,t4830,t4831,t4833,t484,t486,t487,t488,t489,t4895,t4898,t49,t490,t4900,t491,t492,t494,t495,t496,t497,t498,t499,t5,t50,t500,t501,t502,t5041,t5054,t5055,t509,t51,t510,t5103,t511,t512,t513,t514,t515,t516,t517,t5175,t5176,t518,t519,t52,t520,t521,t522,t523,t524,t527,t528,t5280,t529,t53,t530,t531,t534,t5343,t5344,t535,t5354,t5356,t536,t5361,t539,t54,t540,t5411,t542,t543,t545,t546,t547,t548,t5491,t5492,t55,t550,t551,t552,t553,t5551,t5552,t556,t557,t558,t559,t56,t560,t561,t5613,t562,t563,t565,t566,t567,t569,t57,t574,t58,t582,t585,t589,t59,t590,t592,t594,t595,t597,t598,t599,t6,t60,t600,t601,t602,t6023,t604,t605,t606,t608,t609,t61,t610,t611,t613,t614,t616,t617,t62,t624,t63,t630,t632,t635,t636,t641,t643,t644,t645,t647,t6473,t648,t649,t650,t651,t652,t653,t654,t655,t656,t657,t658,t66,t660,t661,t663,t664,t666,t667,t669,t67,t670,t6734,t6735,t6736,t674,t6742,t6743,t6744,t6745,t675,t6754,t6755,t676,t677,t6772,t678,t679,t680,t681,t683,t684,t685,t686,t687,t688,t689,t690,t691,t692,t693,t696,t699,t7,t700,t702,t703,t704,t705,t706,t708,t711,t713,t715,t716,t717,t719,t720,t721,t722,t723,t725,t726,t729,t731,t732,t734,t737,t738,t742,t744,t748,t750,t751,t754,t756,t758,t759,t761,t763,t766,t767,t768,t769,t770,t773,t774,t775,t776,t781,t782,t784,t785,t788,t789,t790,t793,t795,t796,t798,t799,t8,t800,t803,t805,t807,t808,t809,t81,t814,t815,t816,t817,t819,t820,t821,t822,t823,t824,t826,t828,t829,t831,t832,t833,t834,t835,t837,t838,t839,t84,t842,t844,t847,t848,t849,t85,t850,t851,t852,t853,t854,t858,t859,t86,t861,t863,t864,t867,t868,t87,t871,t872,t875,t879,t880,t883,t884,t885,t886,t888,t89,t890,t891,t894,t895,t896,t897,t898,t899,t9,t90,t900,t902,t905,t906,t907,t908,t909,t910,t911,t912,t913,t914,t915,t916,t918,t919,t92,t920,t921,t923,t926,t928,t929,t93,t930,t931,t933,t934,t935,t936,t937,t938,t944,t945,t946,t947,t948,t949,t95,t950,t951,t954,t955,t956,t957,t958,t959,t96,t960,t961,t962,t963,t964,t965,t966,t967,t968,t969,t97,t970,t972,t973,t974,t975,t976,t977,t978,t98,t981,t982,t984,t986,t987,t988,t99,t990,t991,t992,t993,t994,t996,t997,t999] = ct{:};
t4743 = t195.*t2222;
t4744 = t98.*t2602;
t4746 = t56.*t107.*t1919;
t4747 = t20.*t62.*t97.*2.98328125e-2;
t4749 = t3.*t6.*t7.*t9.*t346.*(-9.0./8.0e+2);
t4751 = t5.*t6.*t7.*t12.*t346.*(-9.0./8.0e+2);
t4755 = t7.*t108.*t346.*(-5.625e-3);
t4756 = t7.*t109.*t346.*(-5.625e-3);
t4758 = t7.*t112.*t346.*(-5.625e-3);
t4759 = t7.*t113.*t346.*(-5.625e-3);
t4760 = t7.*t9.*t50.*t346.*(-1.6875e-2);
t4762 = t18.*t3204;
t4764 = t18.*t3206;
t4767 = t4.*t21.*t63.*t1720;
t4772 = t22.*t3208;
t4774 = t22.*t3210;
t4775 = t7.*t3723;
t4776 = t6.*t12.*t18.*t2324;
t4778 = t20.*t3217;
t4790 = t13.*t210.*t346.*(9.0./3.2e+2);
t4800 = t13.*t62.*t63.*t97.*(-5.5078125e-3);
t4804 = t63.*t111.*t130.*(-2.75390625e-3);
t4805 = t63.*t86.*t99.*(-2.75390625e-3);
t4807 = t204.*t2222;
t4809 = t112.*t2603;
t4810 = t114.*t2603;
t4813 = t3.*t7.*t9.*t10.*t346.*(-5.625e-3);
t4815 = t11.*t13.*t49.*t346.*(-5.625e-3);
t4821 = t7.*t127.*t346.*(-5.625e-3);
t4823 = t7.*t129.*t346.*(-5.625e-3);
t4824 = t5.*t13.*t58.*t346.*(-5.625e-3);
t4825 = t7.*t130.*t346.*(-5.625e-3);
t4832 = t18.*t3246;
t4842 = t13.*t215.*t346.*(9.0./3.2e+2);
t4855 = t126.*t2595;
t4856 = t125.*t2600;
t4857 = t210.*t2222;
t4858 = t211.*t2222;
t4859 = t56.*t3099;
t4860 = t127.*t2602;
t4864 = t10.*t13.*t56.*t346.*(-5.625e-3);
t4865 = t12.*t13.*t54.*t346.*(-5.625e-3);
t4870 = t9.*t13.*t56.*t346.*(-1.6875e-2);
t4872 = t19.*t3262;
t4875 = t62.*t97.*t2094;
t4876 = t63.*t97.*t1869;
t4882 = t7.*t21.*t49.*t346.*(9.0./8.0e+2);
t4883 = t7.*t21.*t50.*t346.*(9.0./8.0e+2);
t4894 = t4.*t7.*t21.*t63.*t123.*1.1015625e-2;
t4896 = t6.*t7.*t12.*t2974;
t4903 = t62.*t63.*t97.*t1009;
t4905 = t63.*t111.*t1867;
t4906 = t63.*t109.*t1869;
t4907 = t63.*t110.*t1869;
t4908 = t7.*t51.*t62.*t2124;
t4909 = t6.*t7.*t12.*t2978;
t4910 = t21.*t49.*t56.*t1747;
t4911 = t56.*t107.*t2125;
t4919 = t12.*t194.*t2126;
t4931 = t13.*t20.*t51.*t346.*(-9.0./3.2e+2);
t4935 = t7.*t19.*t54.*t346.*(9.0./8.0e+2);
t4936 = t5.*t7.*t11.*t18.*t346.*(9.0./8.0e+2);
t4937 = t7.*t21.*t54.*t346.*(9.0./8.0e+2);
t4938 = t7.*t21.*t55.*t346.*(9.0./8.0e+2);
t4940 = t7.*t21.*t56.*t346.*(9.0./8.0e+2);
t4957 = t18.*t3388;
t4958 = t7.*t18.*t28.*t2124;
t4967 = t54.*t126.*t2126;
t4971 = t28.*t61.*t2357;
t4975 = t12.*t204.*t2126;
t5000 = t3.*t10.*t13.*t20.*t346.*(9.0./8.0e+2);
t5002 = t7.*t21.*t60.*t346.*(9.0./8.0e+2);
t5003 = t13.*t20.*t57.*t346.*(9.0./8.0e+2);
t5004 = t7.*t21.*t61.*t346.*(9.0./8.0e+2);
t5005 = t6.*t12.*t13.*t19.*t346.*(9.0./8.0e+2);
t5020 = t10.*t20.*t2867;
t5032 = t3.*t10.*t13.*t27.*t346.*(-9.0./3.2e+2);
t5034 = t9.*t10.*t13.*t20.*t346.*(9.0./8.0e+2);
t5039 = t22.*t63.*t202.*(-1.376953125e-3);
t5040 = t22.*t63.*t203.*(-1.376953125e-3);
t5042 = t18.*t3473;
t5052 = t29.*t63.*t202.*(-1.376953125e-3);
t5053 = t29.*t63.*t204.*(-1.376953125e-3);
t5067 = t7.*t13.*t18.*t50.*t130.*(-1.1015625e-2);
t5068 = t29.*t63.*t215.*(-1.376953125e-3);
t5069 = t18.*t21.*t56.*t1720;
t5070 = t21.*t3498;
t5071 = t18.*t3501;
t5073 = t7.*t13.*t21.*t49.*t85.*(-1.1015625e-2);
t5074 = t7.*t13.*t18.*t51.*t87.*(-1.1015625e-2);
t5077 = t19.*t3510;
t5080 = t11.*t26.*t2933;
t5081 = t7.*t63.*t110.*t111.*1.1015625e-2;
t5082 = t7.*t63.*t111.*t114.*5.5078125e-3;
t5086 = t7.*t11.*t98.*t346.*(-9.0./3.2e+2);
t5087 = t7.*t50.*t58.*t346.*(-9.0./3.2e+2);
t5090 = t7.*t11.*t99.*t346.*(9.0./8.0e+2);
t5091 = t7.*t9.*t98.*t346.*(2.7e+1./8.0e+2);
t5100 = t7.*t194.*t346.*1.6875e-2;
t5101 = t7.*t195.*t346.*1.6875e-2;
t5105 = t25.*t3511;
t5120 = t7.*t19.*t21.*t346.*(9.0./8.0e+2);
t5123 = t7.*t13.*t60.*t63.*t98.*1.1015625e-2;
t5124 = t13.*t63.*t107.*t110.*5.5078125e-3;
t5125 = t63.*t107.*t1962;
t5126 = t7.*t63.*t111.*t130.*5.5078125e-3;
t5127 = t7.*t63.*t86.*t99.*5.5078125e-3;
t5129 = t63.*t99.*t1978;
t5132 = t203.*t2369;
t5136 = t7.*t49.*t61.*t346.*(-9.0./3.2e+2);
t5137 = t7.*t50.*t60.*t346.*(-9.0./3.2e+2);
t5138 = t7.*t202.*t346.*(-9.0./3.2e+2);
t5139 = t7.*t203.*t346.*(-9.0./3.2e+2);
t5141 = t4.*t7.*t123.*t346.*(9.0./8.0e+2);
t5143 = t7.*t11.*t112.*t346.*(9.0./8.0e+2);
t5145 = t7.*t12.*t112.*t346.*(9.0./8.0e+2);
t5146 = t7.*t12.*t114.*t346.*(9.0./8.0e+2);
t5155 = t13.*t194.*t346.*5.625e-3;
t5157 = t13.*t195.*t346.*5.625e-3;
t5171 = t13.*t194.*t346.*1.6875e-2;
t5172 = t7.*t202.*t346.*1.6875e-2;
t5173 = t7.*t204.*t346.*1.6875e-2;
t5179 = t6.*t27.*t63.*t1866;
t5186 = t19.*t29.*t111.*t1323;
t5187 = t20.*t29.*t109.*t1323;
t5188 = t20.*t29.*t110.*t1323;
t5204 = t13.*t18.*t20.*t346.*(9.0./8.0e+2);
t5205 = t7.*t19.*t28.*t346.*(9.0./8.0e+2);
t5209 = t63.*t110.*t210.*5.5078125e-3;
t5210 = t63.*t86.*t195.*5.5078125e-3;
t5211 = t13.*t56.*t63.*t203.*5.5078125e-3;
t5213 = t7.*t63.*t127.*t130.*5.5078125e-3;
t5219 = t9.*t13.*t109.*t346.*(-9.0./3.2e+2);
t5222 = t7.*t55.*t62.*t346.*(-9.0./3.2e+2);
t5223 = t11.*t13.*t112.*t346.*(-9.0./3.2e+2);
t5226 = t13.*t49.*t61.*t346.*(9.0./8.0e+2);
t5227 = t13.*t50.*t60.*t346.*(9.0./8.0e+2);
t5228 = t13.*t50.*t61.*t346.*(9.0./8.0e+2);
t5229 = t11.*t13.*t113.*t346.*(9.0./8.0e+2);
t5233 = t13.*t202.*t346.*5.625e-3;
t5234 = t13.*t203.*t346.*5.625e-3;
t5235 = t13.*t204.*t346.*5.625e-3;
t5248 = t13.*t202.*t346.*1.6875e-2;
t5249 = t13.*t204.*t346.*1.6875e-2;
t5250 = t7.*t210.*t346.*1.6875e-2;
t5253 = t7.*t211.*t346.*1.6875e-2;
t5257 = t18.*t3595;
t5258 = t5.*t25.*t61.*t2125;
t5259 = t5.*t25.*t61.*t2126;
t5263 = t9.*t4457;
t5264 = t21.*t56.*t107.*(-2.98328125e-2);
t5266 = t18.*t58.*t113.*(-2.98328125e-2);
t5269 = t13.*t18.*t27.*t346.*(9.0./8.0e+2);
t5271 = t13.*t60.*t63.*t203.*1.1015625e-2;
t5274 = t9.*t4477;
t5276 = t20.*t3611;
t5278 = t22.*t3609;
t5279 = t22.*t3613;
t5281 = t11.*t13.*t127.*t346.*(9.0./8.0e+2);
t5282 = t13.*t210.*t346.*5.625e-3;
t5284 = t13.*t211.*t346.*5.625e-3;
t5288 = t13.*t25.*t62.*t2124;
t5296 = t27.*t3608;
t5297 = t9.*t4046;
t5299 = t27.*t3611;
t5300 = t28.*t3612;
t5301 = t22.*t3628;
t5302 = t28.*t3614;
t5303 = t22.*t3630;
t5304 = t13.*t215.*t346.*5.625e-3;
t5311 = t7.*t20.*t97.*t346.*(9.0./1.6e+2);
t5313 = t7.*t19.*t111.*t346.*(9.0./1.6e+2);
t5314 = t7.*t20.*t109.*t346.*(9.0./1.6e+2);
t5315 = t7.*t20.*t110.*t346.*(9.0./1.6e+2);
t5317 = t3.*t6.*t7.*t9.*t20.*t346.*(9.0./4.0e+2);
t5320 = t7.*t9.*t20.*t58.*t346.*(9.0./1.6e+2);
t5322 = t5.*t7.*t11.*t12.*t18.*t346.*(9.0./1.6e+2);
t5333 = t51.*t111.*t2324;
t5339 = t7.*t19.*t49.*t346.*(-5.625e-3);
t5342 = t7.*t20.*t51.*t346.*(-5.625e-3);
t5355 = -t4898;
t5357 = -t4900;
t5358 = t9.*t4539;
t5359 = t7.*t9.*t21.*t63.*t107.*(-5.5078125e-3);
t5360 = t22.*t62.*t63.*t97.*(-5.5078125e-3);
t5363 = t56.*t107.*t2324;
t5365 = t49.*t61.*t2727;
t5370 = t7.*t12.*t20.*t63.*t110.*(-2.75390625e-3);
t5387 = t5.*t7.*t10.*t21.*t346.*(-9.0./8.0e+2);
t5389 = t3.*t7.*t10.*t20.*t346.*(-5.625e-3);
t5393 = t7.*t27.*t51.*t346.*(-5.625e-3);
t5394 = t13.*t20.*t51.*t346.*(-5.625e-3);
t5395 = t7.*t20.*t57.*t346.*(-5.625e-3);
t5399 = t3.*t21.*t26.*t2324;
t5400 = t22.*t3723;
t5401 = t20.*t21.*t2740;
t5407 = t9.*t13.*t20.*t63.*t109.*(-5.5078125e-3);
t5410 = t13.*t18.*t62.*t2212;
t5414 = t7.*t12.*t27.*t63.*t110.*(-2.75390625e-3);
t5417 = t20.*t126.*t2222;
t5418 = t18.*t129.*t2222;
t5453 = t7.*t25.*t57.*t346.*(-1.6875e-2);
t5455 = t29.*t54.*t63.*t126.*(-2.75390625e-3);
t5474 = t13.*t25.*t62.*t346.*(-5.625e-3);
t5480 = t7.*t60.*t98.*t346.*(9.0./8.0e+1);
t5481 = t7.*t57.*t107.*t346.*(9.0./1.6e+2);
t5482 = t7.*t49.*t130.*t346.*(9.0./1.6e+2);
t5483 = t7.*t60.*t99.*t346.*(9.0./1.6e+2);
t5484 = t7.*t50.*t130.*t346.*(9.0./1.6e+2);
t5487 = t7.*t62.*t97.*t346.*(9.0./4.0e+2);
t5488 = t6.*t7.*t18.*t27.*t346.*(9.0./1.6e+2);
t5495 = t7.*t49.*t85.*t346.*(9.0./1.6e+2);
t5497 = t7.*t51.*t87.*t346.*(9.0./4.0e+2);
t5498 = t111.*t3054;
t5500 = t7.*t10.*t97.*t346.*(-9.0./8.0e+2);
t5501 = t13.*t49.*t51.*t346.*(-5.625e-3);
t5502 = t7.*t49.*t57.*t346.*(-5.625e-3);
t5505 = -t5103;
t5507 = t6.*t4766;
t5508 = t6.*t4768;
t5509 = t19.*t111.*t2324;
t5512 = t18.*t3828;
t5517 = t19.*t20.*t2583;
t5518 = t13.*t54.*t126.*t346.*(9.0./3.2e+2);
t5520 = t13.*t49.*t85.*t346.*(9.0./4.0e+2);
t5521 = t13.*t49.*t86.*t346.*(9.0./4.0e+2);
t5530 = t7.*t13.*t60.*t63.*t99.*(-5.5078125e-3);
t5536 = t6.*t7.*t12.*t54.*t346.*(-9.0./8.0e+2);
t5537 = t5.*t7.*t12.*t58.*t346.*(-9.0./8.0e+2);
t5538 = t10.*t13.*t97.*t346.*(-5.625e-3);
t5543 = t7.*t204.*t346.*(-5.625e-3);
t5548 = -t5175;
t5549 = t18.*t3865;
t5550 = t6.*t4830;
t5553 = t5.*t18.*t61.*t2324;
t5554 = t20.*t29.*t63.*t109.*(-2.75390625e-3);
t5556 = t19.*t3871;
t5557 = t6.*t12.*t3724;
t5559 = t19.*t3872;
t5589 = t7.*t18.*t28.*t346.*(-5.625e-3);
t5590 = t7.*t20.*t28.*t346.*(-5.625e-3);
t5592 = t7.*t13.*t49.*t63.*t85.*(-5.5078125e-3);
t5593 = t63.*t87.*t2092;
t5599 = t9.*t13.*t108.*t346.*(-5.625e-3);
t5600 = t7.*t9.*t125.*t346.*(-5.625e-3);
t5604 = t13.*t51.*t60.*t346.*(-5.625e-3);
t5605 = t13.*t55.*t58.*t346.*(-5.625e-3);
t5606 = t7.*t211.*t346.*(-5.625e-3);
t5607 = t11.*t13.*t111.*t346.*(-5.625e-3);
t5608 = t11.*t13.*t112.*t346.*(-5.625e-3);
t5612 = t7.*t9.*t129.*t346.*(-1.6875e-2);
t5614 = t10.*t27.*t3210;
t5615 = t10.*t27.*t3212;
t5616 = t18.*t3910;
t5618 = t22.*t3910;
t5634 = t13.*t19.*t27.*t346.*(-5.625e-3);
t5636 = t210.*t2600;
t5638 = t13.*t56.*t62.*t346.*(-5.625e-3);
t5639 = t9.*t13.*t123.*t346.*(-1.6875e-2);
t5648 = t7.*t19.*t98.*t346.*(-9.0./3.2e+2);
t5652 = t7.*t62.*t97.*t2124;
t5663 = t5.*t6.*t7.*t11.*t18.*t346.*(-9.0./4.0e+2);
t5665 = t3.*t4.*t7.*t10.*t21.*t346.*(9.0./8.0e+2);
t5668 = t7.*t21.*t107.*t346.*(9.0./8.0e+2);
t5669 = t13.*t19.*t98.*t346.*(9.0./8.0e+2);
t5711 = t62.*t63.*t194.*t1009;
t5712 = t5.*t7.*t12.*t18.*t63.*t130.*5.5078125e-3;
t5715 = t12.*t54.*t110.*t2126;
t5719 = t111.*t130.*t2126;
t5720 = t86.*t99.*t2126;
t5726 = t5.*t6.*t11.*t13.*t18.*t346.*(-9.0./1.6e+2);
t5727 = t13.*t19.*t111.*t346.*(-9.0./3.2e+2);
t5728 = t7.*t12.*t19.*t54.*t346.*(-9.0./3.2e+2);
t5729 = t13.*t20.*t109.*t346.*(-9.0./3.2e+2);
t5731 = t13.*t20.*t110.*t346.*(-9.0./3.2e+2);
t5734 = t3.*t7.*t9.*t10.*t20.*t346.*(9.0./8.0e+2);
t5735 = t3.*t4.*t7.*t10.*t28.*t346.*(9.0./8.0e+2);
t5736 = t13.*t20.*t108.*t346.*(9.0./8.0e+2);
t5738 = t7.*t21.*t123.*t346.*(9.0./8.0e+2);
t5739 = t7.*t21.*t124.*t346.*(9.0./8.0e+2);
t5761 = t18.*t4451;
t5762 = t19.*t28.*t54.*t2126;
t5766 = t7.*t28.*t49.*t63.*t85.*5.5078125e-3;
t5767 = t13.*t19.*t49.*t63.*t86.*5.5078125e-3;
t5768 = t7.*t9.*t12.*t27.*t63.*t109.*5.5078125e-3;
t5771 = t5.*t7.*t12.*t25.*t63.*t130.*5.5078125e-3;
t5773 = t20.*t21.*t3010;
t5776 = t22.*t4477;
t5783 = t5.*t13.*t18.*t61.*t346.*(-9.0./1.6e+2);
t5785 = t13.*t20.*t125.*t346.*(9.0./8.0e+2);
t5786 = t13.*t20.*t126.*t346.*(9.0./8.0e+2);
t5787 = t7.*t21.*t85.*t346.*(9.0./8.0e+2);
t5788 = t10.*t13.*t21.*t56.*t346.*(9.0./8.0e+2);
t5808 = t22.*t4046;
t5810 = t9.*t13.*t20.*t62.*t346.*(9.0./8.0e+2);
t5831 = t7.*t49.*t114.*t346.*(9.0./8.0e+2);
t5832 = t7.*t51.*t111.*t346.*(9.0./8.0e+2);
t5843 = t7.*t49.*t51.*t63.*t86.*5.5078125e-3;
t5844 = t7.*t49.*t51.*t63.*t87.*5.5078125e-3;
t5852 = t13.*t51.*t107.*t346.*(9.0./8.0e+2);
t5853 = t7.*t49.*t130.*t346.*(9.0./8.0e+2);
t5854 = t7.*t60.*t99.*t346.*(9.0./8.0e+2);
t5859 = t7.*t54.*t110.*t346.*1.6875e-2;
t5884 = t3.*t13.*t19.*t20.*t346.*(-9.0./3.2e+2);
t5886 = t7.*t12.*t18.*t20.*t346.*(9.0./8.0e+2);
t5894 = t7.*t13.*t60.*t63.*t195.*1.1015625e-2;
t5897 = t22.*t4168;
t5898 = t13.*t56.*t107.*t346.*(-9.0./1.6e+2);
t5900 = t13.*t56.*t107.*t346.*(9.0./8.0e+2);
t5901 = t7.*t57.*t123.*t346.*(9.0./8.0e+2);
t5902 = t13.*t62.*t97.*t346.*(9.0./8.0e+2);
t5903 = t7.*t55.*t130.*t346.*(9.0./8.0e+2);
t5904 = t7.*t12.*t204.*t346.*(9.0./8.0e+2);
t5916 = t18.*t4174;
t5917 = t25.*t58.*t63.*t1869;
t5928 = t7.*t11.*t21.*t26.*t346.*(9.0./8.0e+2);
t5933 = t22.*t4204;
t5934 = t18.*t4209;
t5938 = t13.*t49.*t87.*t346.*(9.0./8.0e+2);
t5939 = t13.*t50.*t86.*t346.*(9.0./8.0e+2);
t5940 = t13.*t50.*t87.*t346.*(9.0./8.0e+2);
t5949 = t10.*t13.*t20.*t25.*t346.*(9.0./8.0e+2);
t5981 = t7.*t9.*t20.*t125.*t346.*(9.0./1.6e+2);
t5984 = t20.*t97.*t2601;
t5988 = t7.*t10.*t18.*t51.*t346.*(-9.0./8.0e+2);
t5989 = t4.*t7.*t21.*t54.*t346.*(-9.0./8.0e+2);
t5992 = t7.*t10.*t21.*t50.*t346.*(-9.0./8.0e+2);
t5993 = t4.*t13.*t21.*t49.*t346.*(-5.625e-3);
t5994 = t7.*t19.*t111.*t346.*(-5.625e-3);
t5997 = t7.*t20.*t110.*t346.*(-5.625e-3);
t6002 = t18.*t4769;
t6003 = t22.*t4765;
t6004 = t18.*t4771;
t6005 = t21.*t4768;
t6006 = t20.*t21.*t3208;
t6008 = t19.*t20.*t3213;
t6009 = t19.*t21.*t54.*t2324;
t6019 = t4.*t7.*t9.*t21.*t63.*t123.*(-1.1015625e-2);
t6020 = t7.*t18.*t51.*t63.*t87.*(-1.1015625e-2);
t6021 = t7.*t21.*t49.*t63.*t85.*(-5.5078125e-3);
t6024 = t27.*t97.*t2601;
t6025 = t111.*t130.*t2324;
t6026 = t86.*t99.*t2324;
t6028 = t21.*t4806;
t6047 = t3.*t6.*t7.*t12.*t26.*t346.*(-9.0./8.0e+2);
t6048 = t5.*t7.*t11.*t12.*t18.*t346.*(-9.0./8.0e+2);
t6052 = t13.*t19.*t111.*t346.*(-5.625e-3);
t6054 = t13.*t20.*t109.*t346.*(-5.625e-3);
t6055 = t7.*t20.*t125.*t346.*(-5.625e-3);
t6057 = t7.*t27.*t110.*t346.*(-5.625e-3);
t6058 = t13.*t20.*t110.*t346.*(-5.625e-3);
t6059 = t7.*t20.*t126.*t346.*(-5.625e-3);
t6062 = t7.*t18.*t130.*t346.*(-1.6875e-2);
t6063 = t19.*t28.*t54.*t2324;
t6072 = t13.*t18.*t50.*t63.*t87.*(-5.5078125e-3);
t6088 = t13.*t21.*t123.*t346.*(-5.625e-3);
t6089 = t13.*t25.*t114.*t346.*(-5.625e-3);
t6090 = t13.*t21.*t124.*t346.*(-5.625e-3);
t6096 = t7.*t49.*t51.*t61.*t346.*(9.0./1.6e+2);
t6097 = t7.*t110.*t111.*t346.*(9.0./4.0e+2);
t6103 = t7.*t19.*t21.*t54.*t346.*(9.0./4.0e+2);
t6106 = t7.*t60.*t195.*t346.*(9.0./8.0e+1);
t6107 = t7.*t107.*t126.*t346.*(9.0./1.6e+2);
t6113 = t7.*t20.*t25.*t58.*t346.*(9.0./1.6e+2);
t6116 = t18.*t4542;
t6118 = t12.*t19.*t98.*t2324;
t6119 = t19.*t4545;
t6124 = t49.*t61.*t63.*t2092;
t6126 = t13.*t49.*t110.*t346.*(-5.625e-3);
t6128 = t18.*t20.*t63.*t2096;
t6129 = t22.*t4568;
t6131 = t18.*t19.*t3077;
t6132 = t12.*t25.*t99.*t2324;
t6133 = t13.*t60.*t203.*t346.*(9.0./4.0e+2);
t6147 = t6.*t13.*t18.*t20.*t346.*(-9.0./8.0e+2);
t6148 = t7.*t11.*t19.*t21.*t346.*(-9.0./8.0e+2);
t6153 = t56.*t203.*t2222;
t6157 = t7.*t58.*t127.*t346.*(-9.0./8.0e+2);
t6159 = t13.*t49.*t130.*t346.*(-5.625e-3);
t6160 = t7.*t49.*t87.*t346.*(-5.625e-3);
t6162 = t9.*t20.*t29.*t63.*t109.*(-5.5078125e-3);
t6183 = t10.*t13.*t18.*t20.*t346.*(-9.0./8.0e+2);
t6184 = t12.*t13.*t18.*t20.*t346.*(-9.0./8.0e+2);
t6187 = t13.*t63.*t86.*t195.*(-5.5078125e-3);
t6191 = t13.*t54.*t126.*t346.*(-5.625e-3);
t6192 = t9.*t13.*t204.*t346.*(-1.6875e-2);
t6212 = t4.*t7.*t21.*t123.*t346.*(9.0./4.0e+2);
t6213 = t3.*t6.*t7.*t9.*t12.*t19.*t346.*(9.0./4.0e+2);
t6216 = t6.*t7.*t12.*t19.*t54.*t346.*(9.0./4.0e+2);
t6218 = t63.*t110.*t210.*t1009;
t6219 = t63.*t86.*t195.*t1009;
t6225 = t13.*t19.*t49.*t60.*t346.*(9.0./8.0e+2);
t6227 = t7.*t9.*t27.*t109.*t346.*(9.0./8.0e+2);
t6228 = t9.*t13.*t20.*t109.*t346.*(9.0./8.0e+2);
t6229 = t7.*t9.*t20.*t125.*t346.*(9.0./8.0e+2);
t6231 = t5.*t7.*t25.*t130.*t346.*(9.0./8.0e+2);
t6294 = t7.*t49.*t51.*t60.*t346.*(9.0./8.0e+2);
t6295 = t7.*t49.*t51.*t61.*t346.*(9.0./8.0e+2);
t6296 = t7.*t111.*t114.*t346.*(9.0./8.0e+2);
t6314 = t13.*t107.*t110.*t346.*(9.0./8.0e+2);
t6315 = t7.*t111.*t130.*t346.*(9.0./8.0e+2);
t6316 = t7.*t86.*t99.*t346.*(9.0./8.0e+2);
t6329 = t13.*t19.*t21.*t54.*t346.*(9.0./8.0e+2);
t6335 = t7.*t123.*t126.*t346.*(9.0./8.0e+2);
t6336 = t13.*t60.*t195.*t346.*(9.0./8.0e+2);
t6337 = t7.*t60.*t203.*t346.*(9.0./8.0e+2);
t6338 = t13.*t56.*t203.*t346.*(9.0./8.0e+2);
t6339 = t7.*t127.*t130.*t346.*(9.0./8.0e+2);
t6353 = t13.*t20.*t25.*t62.*t346.*(9.0./8.0e+2);
t6370 = t7.*t9.*t20.*t97.*t346.*(-9.0./1.6e+2);
t6381 = t7.*t18.*t20.*t21.*t346.*(9.0./8.0e+2);
t6387 = t7.*t10.*t27.*t97.*t346.*(-9.0./3.2e+2);
t6389 = t7.*t18.*t51.*t62.*t346.*(-9.0./4.0e+2);
t6392 = t4.*t9.*t13.*t21.*t49.*t346.*(9.0./8.0e+2);
t6395 = t7.*t9.*t20.*t109.*t346.*(9.0./8.0e+2);
t6396 = t5.*t7.*t18.*t130.*t346.*(9.0./8.0e+2);
t6397 = t7.*t20.*t51.*t62.*t346.*(9.0./8.0e+2);
t6422 = t7.*t18.*t20.*t28.*t346.*(9.0./8.0e+2);
t6438 = t13.*t18.*t50.*t61.*t346.*(-9.0./8.0e+2);
t6439 = t10.*t13.*t20.*t108.*t346.*(-5.625e-3);
t6440 = t13.*t18.*t50.*t62.*t346.*(-5.625e-3);
t6441 = t7.*t28.*t49.*t61.*t346.*(-5.625e-3);
t6453 = t10.*t13.*t27.*t108.*t346.*(-5.625e-3);
t6468 = t7.*t19.*t21.*t49.*t346.*(-9.0./8.0e+2);
t6469 = t7.*t18.*t21.*t50.*t346.*(-9.0./8.0e+2);
t6484 = t19.*t20.*t3725;
t6499 = t6.*t12.*t13.*t18.*t19.*t346.*(-9.0./8.0e+2);
t6503 = t13.*t111.*t130.*t346.*(-5.625e-3);
t6509 = t13.*t18.*t20.*t62.*t346.*(-9.0./8.0e+2);
t6515 = t7.*t19.*t60.*t98.*t346.*(9.0./1.6e+2);
t6521 = t7.*t18.*t19.*t21.*t346.*(-9.0./8.0e+2);
t6524 = t957+t2071;
t6529 = t7.*t9.*t21.*t107.*t346.*(-9.0./8.0e+2);
t6532 = t7.*t18.*t51.*t61.*t346.*(-5.625e-3);
t6583 = t7.*t49.*t51.*t86.*t346.*(9.0./8.0e+2);
t6584 = t7.*t49.*t51.*t87.*t346.*(9.0./8.0e+2);
t6598 = t13.*t86.*t195.*t346.*(9.0./8.0e+2);
t6618 = t4.*t7.*t9.*t21.*t123.*t346.*(-9.0./4.0e+2);
t6619 = t7.*t18.*t51.*t87.*t346.*(-9.0./4.0e+2);
t6628 = t7.*t28.*t49.*t85.*t346.*(9.0./8.0e+2);
t6629 = t13.*t19.*t49.*t86.*t346.*(9.0./8.0e+2);
t6669 = t7.*t21.*t49.*t85.*t346.*(-9.0./8.0e+2);
t6670 = t5.*t7.*t12.*t18.*t130.*t346.*(-9.0./8.0e+2);
t6680 = t7.*t9.*t12.*t27.*t109.*t346.*(-9.0./8.0e+2);
t6681 = t13.*t18.*t50.*t87.*t346.*(-9.0./8.0e+2);
t6750 = -t6745;
t366 = -t200;
t369 = -t269;
t370 = -t270;
t372 = -t272;
t374 = -t273;
t393 = -t274;
t394 = -t275;
t395 = -t279;
t398 = -t284;
t403 = -t288;
t445 = -t294;
t446 = -t296;
t449 = -t299;
t452 = -t302;
t466 = -t307;
t504 = -t316;
t505 = -t320;
t506 = -t324;
t507 = -t326;
t508 = -t327;
t549 = t200.*(2.0./5.0);
t554 = t200.*(6.0./5.0);
t555 = -t380;
t578 = -t416;
t579 = -t417;
t581 = -t419;
t584 = -t423;
t587 = -t426;
t591 = -t430;
t596 = -t439;
t618 = -t451;
t619 = -t454;
t620 = -t456;
t622 = -t461;
t623 = -t462;
t625 = -t469;
t626 = -t471;
t627 = -t472;
t629 = -t476;
t631 = -t481;
t633 = -t488;
t634 = -t492;
t637 = -t495;
t638 = -t497;
t639 = -t498;
t640 = -t501;
t659 = -t512;
t662 = -t513;
t707 = t6.*t373;
t709 = t6.*t375;
t710 = t6.*t376;
t712 = t6.*t379;
t724 = t193./1.0e+1;
t728 = t6.*t397;
tau = ft_7({dq1,dq2,dq3,dq4,dq5,dq6,t10,t1001,t1002,t1003,t1004,t1005,t1006,t1007,t1009,t101,t1010,t1011,t1013,t1016,t1018,t1019,t102,t1022,t1023,t1025,t1027,t1029,t1030,t1033,t1034,t1035,t1037,t1039,t1041,t1042,t1043,t1047,t1048,t105,t1050,t1051,t1053,t1055,t1056,t1058,t1059,t106,t1060,t1061,t1062,t1063,t1065,t1067,t1068,t107,t1072,t1073,t1074,t1076,t1077,t1078,t108,t1080,t1081,t1082,t1083,t1084,t1085,t1086,t1087,t1088,t1089,t109,t1090,t1091,t1092,t1095,t1096,t1098,t1099,t11,t110,t1100,t1101,t1102,t1103,t1104,t1105,t1106,t1107,t1108,t111,t1110,t1111,t1112,t1113,t1114,t1116,t1117,t1119,t112,t1120,t1122,t1123,t1124,t1127,t113,t1131,t1132,t1133,t1134,t1135,t114,t1141,t1144,t1145,t1147,t1148,t1149,t1151,t1158,t1159,t1160,t1161,t1162,t1163,t1164,t1165,t1166,t1167,t1169,t1170,t1171,t1172,t1173,t1176,t1177,t1178,t1180,t1182,t1183,t1186,t1188,t1189,t119,t1190,t1191,t1192,t1193,t1194,t1195,t1196,t1198,t1199,t12,t120,t1201,t1202,t1203,t1204,t1205,t1207,t1208,t1210,t1211,t1212,t1214,t1215,t1216,t1217,t1218,t1219,t1220,t1221,t1222,t1224,t1227,t1228,t1229,t123,t1230,t1231,t1233,t1234,t1235,t1239,t124,t1240,t1241,t1242,t1243,t1244,t1245,t1246,t1247,t125,t1254,t1255,t1256,t126,t1263,t1266,t127,t128,t1283,t1286,t1287,t1288,t1289,t129,t1291,t1293,t1295,t1296,t1297,t1298,t1299,t13,t130,t131,t1316,t1317,t1319,t132,t1320,t1323,t1324,t1325,t1326,t1327,t1328,t1329,t133,t1331,t1332,t1333,t1334,t1335,t1345,t1346,t1347,t1349,t135,t1352,t1353,t1355,t1356,t1357,t1358,t1359,t1361,t1362,t1363,t1366,t1369,t137,t1370,t1371,t1372,t1373,t1375,t1376,t1377,t1379,t138,t1380,t1383,t1385,t1386,t1387,t1388,t139,t1390,t1391,t1392,t1393,t1395,t1397,t1398,t1399,t140,t1400,t1401,t1402,t1403,t1404,t1406,t1407,t1408,t1409,t141,t1410,t1413,t1416,t1417,t1419,t142,t1423,t1424,t1426,t1427,t1429,t143,t1432,t1433,t1434,t1435,t1438,t1441,t1442,t1443,t1445,t1447,t1450,t1452,t1453,t1456,t1457,t1458,t1462,t1463,t1464,t1465,t1466,t1467,t1468,t1469,t1470,t1473,t1475,t1477,t1479,t1480,t1481,t1482,t1483,t1484,t1488,t1489,t1490,t1491,t1493,t1494,t1495,t1496,t1497,t1498,t1499,t1500,t1502,t1503,t1504,t1505,t1511,t1513,t1523,t1524,t1525,t1526,t1528,t1530,t1531,t1532,t1533,t1534,t1536,t1537,t1538,t1539,t1540,t1541,t1544,t1545,t1546,t1554,t1555,t1556,t1557,t1558,t1562,t1563,t1564,t1566,t1567,t1568,t1571,t1575,t1576,t158,t1581,t1582,t1584,t1585,t1586,t1587,t1589,t159,t1590,t1591,t1592,t1593,t1595,t1597,t1598,t1599,t160,t1600,t1601,t1602,t1603,t1604,t1605,t1606,t1607,t1608,t1609,t161,t1610,t1611,t1612,t1613,t1614,t1618,t1619,t162,t1620,t1621,t1623,t1624,t1626,t1627,t1628,t1629,t163,t1630,t1631,t1632,t1633,t1634,t1635,t1637,t164,t1643,t165,t1654,t1655,t1656,t1657,t166,t1660,t1661,t1662,t1663,t1664,t1665,t1666,t1668,t1669,t167,t1670,t1671,t1673,t1675,t1676,t1677,t168,t1681,t1682,t1684,t1685,t1686,t1688,t1689,t1690,t1691,t1692,t1695,t1696,t1697,t1698,t170,t1700,t1701,t1702,t1703,t1704,t1705,t1706,t1709,t171,t1711,t1713,t1714,t1715,t1716,t1717,t1718,t1719,t1720,t1721,t1722,t1723,t1724,t1726,t1727,t1728,t173,t1730,t1732,t1734,t1736,t1739,t1741,t1742,t1749,t1750,t1752,t1753,t1754,t1755,t1756,t1758,t1759,t1760,t1761,t1763,t1764,t1765,t1766,t1767,t1768,t177,t1772,t1773,t1776,t1778,t1779,t178,t1780,t1781,t1782,t1785,t1786,t1787,t179,t1794,t1796,t18,t180,t1800,t1801,t1802,t1803,t1804,t1805,t1806,t1808,t181,t1815,t1816,t1817,t1818,t1819,t182,t1820,t1821,t1822,t1823,t1827,t1828,t1829,t183,t1830,t1831,t1832,t1833,t1837,t1838,t1839,t184,t1840,t1844,t1845,t1847,t1849,t185,t1850,t1851,t1852,t1853,t1854,t1857,t1858,t1859,t186,t1860,t1861,t1862,t1866,t1867,t1868,t1869,t187,t1870,t1871,t1872,t1873,t1874,t1875,t1876,t1877,t1878,t1879,t188,t1881,t1882,t1883,t1884,t1885,t1888,t1889,t189,t1890,t1893,t1895,t1896,t1897,t1898,t1899,t19,t1900,t1901,t1902,t1904,t1906,t1907,t191,t1911,t1913,t1917,t1919,t192,t1921,t1922,t1923,t1925,t1926,t1927,t193,t1931,t1936,t1937,t194,t1943,t1944,t1947,t1949,t195,t1950,t1952,t1953,t1954,t1955,t1956,t1957,t1958,t1959,t1962,t1964,t1965,t1966,t1967,t1970,t1971,t1973,t1974,t1975,t1976,t1977,t1978,t1980,t1981,t1982,t1983,t1984,t1985,t1986,t1987,t1988,t1990,t1991,t1992,t1993,t1994,t1997,t2,t20,t200,t2001,t2002,t2003,t2004,t2005,t2007,t2009,t201,t2010,t2014,t2015,t2017,t2018,t202,t2021,t2023,t2024,t2025,t2029,t203,t2030,t2031,t2034,t2035,t2036,t2037,t2038,t2039,t204,t2040,t2041,t2043,t2046,t2047,t2048,t2050,t2053,t2054,t2055,t2056,t2057,t2058,t2059,t206,t2061,t2063,t2064,t2065,t2066,t2067,t2068,t2069,t2070,t2072,t2073,t2075,t2077,t2078,t208,t2080,t2081,t2083,t2084,t2085,t2086,t2087,t2089,t209,t2090,t2091,t2092,t2093,t2094,t2096,t2097,t2098,t2099,t21,t210,t2106,t211,t2111,t2112,t2115,t2118,t212,t2121,t2124,t2125,t2126,t2128,t213,t2132,t2134,t2135,t2136,t2137,t2138,t2139,t214,t2140,t2141,t2144,t2145,t2148,t215,t2152,t2154,t2156,t2157,t2158,t2159,t216,t2160,t2161,t2162,t2163,t2165,t2167,t2169,t217,t2171,t2172,t2175,t2176,t2177,t2178,t2179,t218,t2180,t2181,t2182,t2183,t2184,t2185,t2186,t2187,t2188,t2189,t219,t2190,t2191,t2193,t2196,t2197,t2198,t2199,t22,t220,t2201,t2203,t2204,t2205,t2206,t2208,t221,t2212,t2213,t2214,t2215,t2216,t2217,t2219,t222,t2221,t2222,t2223,t2224,t2225,t2227,t2229,t223,t2231,t2232,t2233,t2235,t2236,t2237,t2238,t2239,t224,t2240,t2242,t2243,t2245,t2246,t2247,t2248,t2249,t225,t2250,t2251,t2252,t2253,t2254,t2256,t2258,t2259,t226,t2263,t2264,t2265,t2266,t2267,t2268,t2269,t227,t2277,t2278,t228,t2281,t2282,t2283,t2284,t2285,t2287,t2289,t229,t2290,t2292,t2293,t2296,t2297,t2299,t230,t2300,t2301,t231,t2310,t2312,t2313,t2314,t2319,t2322,t2323,t2324,t2326,t2327,t2329,t2330,t2331,t2332,t2333,t2334,t2338,t2339,t234,t2342,t2343,t2344,t235,t2356,t2357,t2358,t236,t2362,t2363,t2364,t2365,t2368,t237,t2370,t2372,t2374,t2376,t2378,t2379,t238,t2381,t2382,t2383,t2386,t2387,t239,t2390,t2392,t2394,t2395,t2396,t2397,t2398,t240,t2400,t2401,t2402,t2403,t2405,t2408,t2409,t241,t2410,t2412,t2413,t2414,t2416,t2417,t2418,t2419,t242,t2421,t2422,t2423,t2424,t2425,t2426,t2427,t2428,t2429,t243,t2430,t2431,t2432,t2433,t2436,t2437,t2438,t2439,t244,t2440,t2449,t245,t2450,t2451,t2452,t2453,t2454,t2455,t2456,t2457,t2459,t246,t2464,t2465,t2466,t2467,t2468,t2469,t247,t2470,t2471,t2472,t2473,t2474,t2475,t2476,t2477,t2478,t2479,t248,t2481,t2482,t2483,t2484,t2485,t2486,t2487,t2488,t249,t2491,t2492,t2494,t2495,t2496,t2498,t25,t250,t2504,t2508,t251,t2511,t2512,t2513,t2514,t2515,t2516,t2517,t2518,t252,t2520,t2523,t2524,t2525,t2527,t2529,t253,t2531,t2534,t2536,t2537,t2538,t2541,t2542,t2546,t2547,t2548,t255,t2550,t2552,t2553,t2554,t2555,t2556,t2559,t256,t2560,t2563,t2564,t2565,t2566,t2567,t2568,t2569,t2570,t2571,t2572,t2573,t2574,t2575,t2576,t2577,t2578,t2579,t2580,t2581,t2582,t2583,t2585,t2586,t2587,t2588,t259,t2591,t2593,t2594,t2595,t2596,t2597,t2598,t2599,t26,t260,t2600,t2601,t2602,t2603,t2604,t2605,t2607,t2608,t2609,t261,t2610,t2611,t2614,t2615,t2616,t2617,t262,t2622,t2623,t2625,t2628,t2629,t263,t2631,t2632,t2634,t2638,t2644,t2646,t2649,t265,t2650,t2652,t2659,t2660,t2661,t2665,t2666,t2667,t2668,t2669,t267,t2670,t2671,t2672,t2673,t2674,t2675,t2679,t2681,t2682,t2683,t2685,t2686,t2689,t269,t2692,t2694,t2696,t2697,t2698,t27,t2700,t2701,t2702,t2703,t2705,t2706,t2707,t2711,t2723,t2724,t2725,t2726,t2727,t2729,t2730,t2732,t2733,t2734,t2735,t2736,t2738,t2739,t274,t2740,t2741,t2742,t2744,t2745,t2746,t2747,t2748,t2749,t2751,t2752,t2753,t2754,t2755,t2756,t2757,t2758,t2759,t276,t2762,t2763,t2764,t2765,t2766,t2767,t2769,t277,t2770,t2771,t2776,t2778,t2779,t278,t2780,t2782,t2784,t2785,t2786,t2788,t279,t2792,t2793,t2795,t28,t280,t2800,t2802,t2803,t2804,t2806,t2807,t2809,t281,t2810,t2812,t2813,t2814,t2815,t2819,t2820,t2821,t2822,t2825,t2827,t2828,t2829,t283,t2830,t2832,t2833,t2834,t2836,t2839,t2842,t2843,t2844,t285,t2850,t2854,t2858,t286,t2860,t2862,t2864,t2865,t2866,t2867,t2869,t287,t2870,t2871,t2872,t2873,t2877,t288,t2880,t2882,t2883,t2885,t2887,t2888,t289,t2890,t2891,t2892,t2899,t29,t290,t2900,t2901,t2902,t2903,t2904,t2905,t2906,t2911,t2912,t2913,t2916,t2919,t292,t2921,t2922,t2923,t2924,t2925,t2926,t2927,t2928,t2929,t293,t2930,t2931,t2932,t2933,t2934,t2935,t2937,t2938,t2939,t2940,t2942,t2943,t2944,t2945,t2946,t2947,t2948,t2949,t295,t2950,t2951,t2952,t2953,t2954,t2956,t2957,t2959,t296,t2960,t2962,t2964,t2965,t2966,t2967,t2968,t297,t2970,t2973,t2975,t2977,t298,t2981,t2983,t2984,t2986,t2988,t299,t2991,t2995,t2997,t2998,t3,t300,t3002,t3003,t3004,t3006,t3007,t301,t3010,t3011,t3012,t3013,t3015,t3016,t3017,t3020,t3021,t3023,t3025,t3028,t303,t3034,t3035,t3036,t3037,t304,t3040,t3042,t3046,t3047,t3049,t305,t3051,t3052,t3053,t3054,t3056,t3057,t3058,t3059,t306,t3060,t3061,t3062,t3064,t3065,t3066,t3067,t3068,t3069,t3070,t3071,t3072,t3073,t3074,t3075,t3076,t3077,t3078,t3079,t308,t3080,t3081,t3082,t3083,t3085,t3087,t3088,t309,t3091,t3092,t3093,t3094,t3095,t3096,t3097,t3099,t3100,t3101,t3102,t3103,t3104,t3107,t3108,t3109,t311,t3110,t3111,t3112,t3118,t312,t3126,t3128,t313,t3131,t3132,t3133,t3134,t3135,t3138,t3139,t314,t3140,t3142,t3143,t3146,t3147,t3148,t315,t3156,t316,t3160,t3161,t3162,t3163,t3164,t3167,t3168,t317,t3170,t3175,t318,t3182,t3185,t3187,t3188,t3189,t319,t3190,t3192,t3193,t3196,t3197,t3198,t3199,t320,t3200,t3203,t3204,t3205,t3206,t3207,t3208,t3209,t321,t3210,t3211,t3212,t3213,t3214,t3215,t3216,t3217,t3218,t3219,t322,t3220,t3221,t3222,t3223,t3224,t3225,t3226,t3227,t3228,t323,t3230,t3231,t3232,t3234,t324,t3240,t3241,t3245,t3246,t3247,t3249,t325,t3250,t3251,t3252,t3257,t3258,t326,t3260,t3262,t3271,t3273,t3274,t3275,t3276,t3277,t3279,t328,t3283,t3284,t3286,t329,t3298,t330,t3301,t3302,t3303,t3304,t3305,t3307,t3308,t331,t3313,t3314,t3315,t332,t3322,t3323,t3324,t3326,t3327,t3328,t3329,t333,t3330,t3332,t3333,t3334,t3335,t3336,t334,t3341,t3342,t3343,t3344,t3345,t3346,t3347,t3348,t3353,t3358,t3359,t336,t3360,t3361,t3363,t337,t3370,t3373,t338,t3380,t3381,t3382,t3383,t3384,t3386,t339,t3391,t3395,t3396,t3397,t3399,t3401,t3402,t3405,t341,t3412,t3416,t3419,t342,t3421,t3422,t3425,t3427,t3429,t343,t3430,t3433,t3434,t3436,t344,t3441,t3442,t3448,t345,t3450,t3451,t3452,t3453,t3454,t3455,t3456,t3458,t3459,t346,t3462,t3463,t3465,t3466,t347,t3470,t3471,t3472,t3473,t3475,t3478,t3479,t348,t3480,t3481,t3483,t3484,t3485,t3486,t3487,t3488,t3489,t349,t3490,t3491,t3497,t3498,t350,t3501,t3504,t3505,t3506,t3507,t3511,t3512,t3519,t352,t3520,t3521,t3522,t3523,t3525,t3526,t3527,t3528,t3529,t353,t3531,t3533,t3535,t3536,t3538,t354,t3541,t3544,t3545,t3548,t3549,t355,t3554,t3555,t3557,t3559,t356,t3561,t3564,t3566,t3569,t357,t3570,t3572,t358,t3586,t3587,t3589,t3590,t3591,t3592,t3593,t3596,t3598,t360,t3605,t3608,t3609,t3610,t3611,t3612,t3613,t3614,t3615,t3616,t3617,t3627,t3628,t3629,t3630,t3632,t3634,t3635,t3636,t3637,t3638,t3639,t364,t3640,t3642,t3643,t3645,t3646,t3647,t3648,t365,t3650,t3651,t3652,t3653,t3654,t3656,t3657,t3659,t366,t3660,t3663,t3664,t3667,t3668,t367,t3671,t3678,t3679,t368,t3680,t3681,t3682,t3686,t3687,t369,t3690,t3691,t3692,t3694,t3695,t3696,t3697,t3698,t3699,t370,t3700,t3701,t3702,t3703,t3704,t3705,t3708,t371,t3711,t3712,t3713,t3714,t3716,t3717,t372,t3720,t3721,t3722,t3723,t3724,t3725,t3726,t3727,t3728,t3729,t373,t3730,t3731,t3732,t3736,t3737,t3738,t3739,t374,t3740,t3741,t3742,t3743,t3744,t3745,t3747,t3748,t3749,t375,t3750,t3751,t3758,t3759,t376,t3763,t3768,t377,t3774,t3776,t3778,t378,t3780,t3781,t3782,t379,t3793,t3795,t3796,t380,t3806,t381,t3810,t3811,t3812,t3813,t3814,t382,t3821,t3822,t3823,t3824,t3826,t3827,t3828,t3829,t383,t3837,t3838,t3839,t384,t3840,t3841,t385,t3856,t3858,t386,t3860,t3861,t3862,t3863,t3864,t3865,t3868,t3869,t387,t3871,t3872,t388,t3884,t3885,t389,t3908,t3909,t391,t3910,t392,t3928,t393,t3931,t3932,t3935,t3936,t3939,t394,t3941,t395,t3959,t396,t3960,t3962,t3964,t3966,t3967,t3968,t397,t3970,t3971,t3972,t3973,t3977,t3979,t398,t3984,t3985,t3986,t399,t3996,t3997,t3999,t4,t400,t4002,t4004,t4007,t4008,t401,t4015,t4016,t4018,t4019,t402,t4023,t4024,t4026,t4029,t403,t4031,t4032,t4033,t4034,t4035,t4036,t4038,t404,t4040,t4042,t4043,t4046,t4047,t4048,t405,t4051,t4052,t4054,t4057,t4058,t4059,t406,t4060,t4061,t4062,t4063,t4064,t4067,t4068,t4069,t407,t4072,t4073,t4074,t4075,t4077,t4078,t4079,t408,t4081,t4084,t4085,t4087,t409,t4090,t4096,t410,t4103,t4104,t4105,t4106,t4107,t4109,t411,t4113,t4115,t4116,t412,t413,t414,t415,t4152,t4153,t416,t4166,t4167,t4168,t417,t4171,t4172,t4173,t4174,t4175,t4176,t4178,t418,t4183,t4188,t419,t4198,t420,t4204,t4205,t4206,t4207,t4208,t4209,t421,t4210,t4211,t4212,t4213,t4219,t422,t4221,t423,t4230,t4231,t4232,t4233,t4234,t4235,t4236,t4237,t4238,t424,t4240,t425,t4252,t4253,t4257,t4258,t4259,t426,t4260,t4261,t4262,t4263,t4265,t4266,t427,t4272,t4274,t4275,t4276,t4277,t4279,t4280,t4281,t4284,t4285,t4287,t4288,t429,t4293,t4294,t4295,t4298,t4299,t430,t4300,t4301,t431,t4311,t4312,t4313,t4315,t432,t4322,t4327,t433,t4331,t4336,t4337,t4338,t434,t4340,t4341,t4342,t4344,t4345,t4347,t4349,t435,t4352,t4354,t436,t4361,t4364,t437,t4372,t4379,t438,t4381,t4383,t4384,t4386,t4387,t4388,t4389,t439,t4390,t4391,t4393,t4394,t440,t4403,t4405,t4406,t4407,t4409,t441,t4413,t4416,t4418,t442,t4420,t4423,t4426,t4429,t443,t4430,t4437,t4438,t444,t4440,t4441,t4442,t4443,t4445,t4446,t4449,t445,t4451,t4452,t4454,t4456,t4457,t4458,t446,t4461,t4462,t4463,t4464,t4466,t4471,t4474,t4475,t4476,t4477,t4478,t4479,t4482,t4483,t4485,t4486,t4487,t4489,t449,t4490,t4493,t4494,t4496,t4498,t450,t4501,t4503,t4504,t4506,t4507,t4508,t451,t4511,t4517,t452,t4522,t4529,t453,t4530,t4538,t4539,t454,t4542,t4543,t4544,t4545,t4546,t4547,t4557,t4558,t456,t4562,t4565,t4566,t4567,t4568,t4569,t4570,t4572,t4573,t4574,t4576,t4578,t4579,t458,t4580,t4581,t4582,t4584,t459,t4590,t460,t461,t4613,t4616,t4618,t4619,t4624,t4626,t4627,t4628,t4629,t463,t4631,t4632,t4639,t464,t465,t466,t4664,t467,t4673,t4674,t4675,t4676,t468,t4685,t4686,t469,t4694,t470,t4702,t4705,t471,t4711,t4713,t4714,t4715,t4718,t472,t4723,t4724,t4725,t473,t4734,t4737,t4739,t474,t4740,t4742,t4743,t4744,t4746,t4747,t4749,t475,t4751,t4755,t4756,t4758,t4759,t4760,t4762,t4763,t4764,t4765,t4766,t4767,t4768,t4769,t477,t4770,t4771,t4772,t4773,t4774,t4775,t4776,t4778,t478,t479,t4790,t48,t480,t4800,t4804,t4805,t4806,t4807,t4808,t4809,t481,t4810,t4813,t4815,t482,t4821,t4823,t4824,t4825,t483,t4830,t4831,t4832,t4833,t484,t4842,t4855,t4856,t4857,t4858,t4859,t486,t4860,t4864,t4865,t487,t4870,t4872,t4875,t4876,t488,t4882,t4883,t489,t4894,t4895,t4896,t4898,t49,t490,t4903,t4905,t4906,t4907,t4908,t4909,t491,t4910,t4911,t4919,t492,t4931,t4935,t4936,t4937,t4938,t494,t4940,t4957,t4958,t496,t4967,t497,t4971,t4975,t498,t499,t5,t50,t500,t5000,t5002,t5003,t5004,t5005,t501,t502,t5020,t5032,t5034,t5039,t504,t5040,t5041,t5042,t505,t5052,t5053,t5054,t5055,t506,t5067,t5068,t5069,t507,t5070,t5071,t5073,t5074,t5077,t508,t5080,t5081,t5082,t5086,t5087,t509,t5090,t5091,t51,t510,t5100,t5101,t5105,t511,t512,t5120,t5123,t5124,t5125,t5126,t5127,t5129,t5132,t5136,t5137,t5138,t5139,t514,t5141,t5143,t5145,t5146,t515,t5155,t5157,t516,t517,t5171,t5172,t5173,t5176,t5179,t518,t5186,t5187,t5188,t519,t52,t520,t5204,t5205,t5209,t521,t5210,t5211,t5213,t5219,t522,t5222,t5223,t5226,t5227,t5228,t5229,t523,t5233,t5234,t5235,t524,t5248,t5249,t5250,t5253,t5257,t5258,t5259,t5263,t5264,t5266,t5269,t527,t5271,t5274,t5276,t5278,t5279,t528,t5280,t5281,t5282,t5284,t5288,t529,t5296,t5297,t5299,t53,t530,t5300,t5301,t5302,t5303,t5304,t531,t5311,t5313,t5314,t5315,t5317,t5320,t5322,t5333,t5339,t534,t5342,t5343,t5344,t535,t5354,t5355,t5356,t5357,t5358,t5359,t536,t5360,t5361,t5363,t5365,t5370,t5387,t5389,t539,t5393,t5394,t5395,t5399,t54,t540,t5400,t5401,t5407,t5410,t5411,t5414,t5417,t5418,t542,t543,t545,t5453,t5455,t546,t547,t5474,t548,t5480,t5481,t5482,t5483,t5484,t5487,t5488,t549,t5491,t5492,t5495,t5497,t5498,t55,t550,t5500,t5501,t5502,t5505,t5507,t5508,t5509,t551,t5512,t5517,t5518,t552,t5520,t5521,t553,t5530,t5536,t5537,t5538,t554,t5543,t5548,t5549,t555,t5550,t5551,t5552,t5553,t5554,t5556,t5557,t5559,t556,t557,t558,t5589,t559,t5590,t5592,t5593,t5599,t56,t560,t5600,t5604,t5605,t5606,t5607,t5608,t561,t5612,t5613,t5614,t5615,t5616,t5618,t562,t563,t5634,t5636,t5638,t5639,t5648,t565,t5652,t566,t5663,t5665,t5668,t5669,t567,t569,t57,t5711,t5712,t5715,t5719,t5720,t5726,t5727,t5728,t5729,t5731,t5734,t5735,t5736,t5738,t5739,t574,t5761,t5762,t5766,t5767,t5768,t5771,t5773,t5776,t578,t5783,t5785,t5786,t5787,t5788,t579,t58,t5808,t581,t5810,t582,t5831,t5832,t584,t5843,t5844,t585,t5852,t5853,t5854,t5859,t587,t5884,t5886,t589,t5894,t5897,t5898,t59,t590,t5900,t5901,t5902,t5903,t5904,t591,t5916,t5917,t592,t5928,t5933,t5934,t5938,t5939,t594,t5940,t5949,t595,t596,t597,t598,t5981,t5984,t5988,t5989,t599,t5992,t5993,t5994,t5997,t6,t60,t600,t6002,t6003,t6004,t6005,t6006,t6008,t6009,t601,t6019,t602,t6020,t6021,t6023,t6024,t6025,t6026,t6028,t604,t6047,t6048,t605,t6052,t6054,t6055,t6057,t6058,t6059,t606,t6062,t6063,t6072,t608,t6088,t6089,t609,t6090,t6096,t6097,t61,t610,t6103,t6106,t6107,t611,t6113,t6116,t6118,t6119,t6124,t6126,t6128,t6129,t613,t6131,t6132,t6133,t614,t6147,t6148,t6153,t6157,t6159,t616,t6160,t6162,t617,t618,t6183,t6184,t6187,t619,t6191,t6192,t62,t620,t6212,t6213,t6216,t6218,t6219,t622,t6225,t6227,t6228,t6229,t623,t6231,t624,t625,t626,t627,t629,t6294,t6295,t6296,t63,t630,t631,t6314,t6315,t6316,t632,t6329,t633,t6335,t6336,t6337,t6338,t6339,t634,t635,t6353,t636,t637,t6370,t638,t6381,t6387,t6389,t639,t6392,t6395,t6396,t6397,t640,t641,t6422,t643,t6438,t6439,t644,t6440,t6441,t645,t6453,t6468,t6469,t647,t6473,t648,t6484,t649,t6499,t650,t6503,t6509,t651,t6515,t652,t6521,t6524,t6529,t653,t6532,t654,t655,t656,t657,t658,t6583,t6584,t659,t6598,t66,t660,t661,t6618,t6619,t662,t6628,t6629,t663,t664,t666,t6669,t667,t6670,t6680,t6681,t669,t67,t670,t6734,t6735,t6736,t674,t6742,t6743,t6744,t675,t6750,t6754,t6755,t676,t677,t6772,t678,t679,t680,t681,t683,t684,t685,t686,t687,t688,t689,t690,t691,t692,t693,t696,t699,t7,t700,t702,t703,t704,t705,t706,t707,t708,t709,t710,t711,t712,t713,t715,t716,t717,t719,t720,t721,t722,t723,t724,t725,t726,t728,t729,t731,t732,t734,t737,t738,t742,t744,t748,t750,t751,t754,t756,t758,t759,t761,t763,t766,t767,t768,t769,t770,t773,t774,t775,t776,t781,t782,t784,t785,t788,t789,t790,t793,t795,t796,t798,t799,t8,t800,t803,t805,t807,t808,t809,t81,t814,t815,t816,t817,t819,t820,t821,t822,t823,t824,t826,t828,t829,t831,t832,t833,t834,t835,t837,t838,t839,t84,t842,t844,t847,t848,t849,t85,t850,t851,t852,t853,t854,t858,t859,t86,t861,t863,t864,t867,t868,t87,t871,t872,t875,t879,t880,t883,t884,t885,t886,t888,t89,t890,t891,t894,t895,t896,t897,t898,t899,t9,t90,t900,t902,t905,t906,t907,t908,t909,t910,t911,t912,t913,t914,t915,t916,t918,t919,t92,t920,t921,t923,t926,t928,t929,t93,t930,t931,t933,t934,t935,t936,t937,t938,t944,t945,t946,t947,t948,t949,t95,t950,t951,t954,t955,t956,t957,t958,t959,t96,t960,t961,t962,t963,t964,t965,t966,t967,t968,t969,t97,t970,t972,t973,t974,t975,t976,t977,t978,t98,t981,t982,t984,t986,t987,t988,t99,t990,t991,t992,t993,t994,t996,t997,t999});
end
function tau = ft_7(ct)
[dq1,dq2,dq3,dq4,dq5,dq6,t10,t1001,t1002,t1003,t1004,t1005,t1006,t1007,t1009,t101,t1010,t1011,t1013,t1016,t1018,t1019,t102,t1022,t1023,t1025,t1027,t1029,t1030,t1033,t1034,t1035,t1037,t1039,t1041,t1042,t1043,t1047,t1048,t105,t1050,t1051,t1053,t1055,t1056,t1058,t1059,t106,t1060,t1061,t1062,t1063,t1065,t1067,t1068,t107,t1072,t1073,t1074,t1076,t1077,t1078,t108,t1080,t1081,t1082,t1083,t1084,t1085,t1086,t1087,t1088,t1089,t109,t1090,t1091,t1092,t1095,t1096,t1098,t1099,t11,t110,t1100,t1101,t1102,t1103,t1104,t1105,t1106,t1107,t1108,t111,t1110,t1111,t1112,t1113,t1114,t1116,t1117,t1119,t112,t1120,t1122,t1123,t1124,t1127,t113,t1131,t1132,t1133,t1134,t1135,t114,t1141,t1144,t1145,t1147,t1148,t1149,t1151,t1158,t1159,t1160,t1161,t1162,t1163,t1164,t1165,t1166,t1167,t1169,t1170,t1171,t1172,t1173,t1176,t1177,t1178,t1180,t1182,t1183,t1186,t1188,t1189,t119,t1190,t1191,t1192,t1193,t1194,t1195,t1196,t1198,t1199,t12,t120,t1201,t1202,t1203,t1204,t1205,t1207,t1208,t1210,t1211,t1212,t1214,t1215,t1216,t1217,t1218,t1219,t1220,t1221,t1222,t1224,t1227,t1228,t1229,t123,t1230,t1231,t1233,t1234,t1235,t1239,t124,t1240,t1241,t1242,t1243,t1244,t1245,t1246,t1247,t125,t1254,t1255,t1256,t126,t1263,t1266,t127,t128,t1283,t1286,t1287,t1288,t1289,t129,t1291,t1293,t1295,t1296,t1297,t1298,t1299,t13,t130,t131,t1316,t1317,t1319,t132,t1320,t1323,t1324,t1325,t1326,t1327,t1328,t1329,t133,t1331,t1332,t1333,t1334,t1335,t1345,t1346,t1347,t1349,t135,t1352,t1353,t1355,t1356,t1357,t1358,t1359,t1361,t1362,t1363,t1366,t1369,t137,t1370,t1371,t1372,t1373,t1375,t1376,t1377,t1379,t138,t1380,t1383,t1385,t1386,t1387,t1388,t139,t1390,t1391,t1392,t1393,t1395,t1397,t1398,t1399,t140,t1400,t1401,t1402,t1403,t1404,t1406,t1407,t1408,t1409,t141,t1410,t1413,t1416,t1417,t1419,t142,t1423,t1424,t1426,t1427,t1429,t143,t1432,t1433,t1434,t1435,t1438,t1441,t1442,t1443,t1445,t1447,t1450,t1452,t1453,t1456,t1457,t1458,t1462,t1463,t1464,t1465,t1466,t1467,t1468,t1469,t1470,t1473,t1475,t1477,t1479,t1480,t1481,t1482,t1483,t1484,t1488,t1489,t1490,t1491,t1493,t1494,t1495,t1496,t1497,t1498,t1499,t1500,t1502,t1503,t1504,t1505,t1511,t1513,t1523,t1524,t1525,t1526,t1528,t1530,t1531,t1532,t1533,t1534,t1536,t1537,t1538,t1539,t1540,t1541,t1544,t1545,t1546,t1554,t1555,t1556,t1557,t1558,t1562,t1563,t1564,t1566,t1567,t1568,t1571,t1575,t1576,t158,t1581,t1582,t1584,t1585,t1586,t1587,t1589,t159,t1590,t1591,t1592,t1593,t1595,t1597,t1598,t1599,t160,t1600,t1601,t1602,t1603,t1604,t1605,t1606,t1607,t1608,t1609,t161,t1610,t1611,t1612,t1613,t1614,t1618,t1619,t162,t1620,t1621,t1623,t1624,t1626,t1627,t1628,t1629,t163,t1630,t1631,t1632,t1633,t1634,t1635,t1637,t164,t1643,t165,t1654,t1655,t1656,t1657,t166,t1660,t1661,t1662,t1663,t1664,t1665,t1666,t1668,t1669,t167,t1670,t1671,t1673,t1675,t1676,t1677,t168,t1681,t1682,t1684,t1685,t1686,t1688,t1689,t1690,t1691,t1692,t1695,t1696,t1697,t1698,t170,t1700,t1701,t1702,t1703,t1704,t1705,t1706,t1709,t171,t1711,t1713,t1714,t1715,t1716,t1717,t1718,t1719,t1720,t1721,t1722,t1723,t1724,t1726,t1727,t1728,t173,t1730,t1732,t1734,t1736,t1739,t1741,t1742,t1749,t1750,t1752,t1753,t1754,t1755,t1756,t1758,t1759,t1760,t1761,t1763,t1764,t1765,t1766,t1767,t1768,t177,t1772,t1773,t1776,t1778,t1779,t178,t1780,t1781,t1782,t1785,t1786,t1787,t179,t1794,t1796,t18,t180,t1800,t1801,t1802,t1803,t1804,t1805,t1806,t1808,t181,t1815,t1816,t1817,t1818,t1819,t182,t1820,t1821,t1822,t1823,t1827,t1828,t1829,t183,t1830,t1831,t1832,t1833,t1837,t1838,t1839,t184,t1840,t1844,t1845,t1847,t1849,t185,t1850,t1851,t1852,t1853,t1854,t1857,t1858,t1859,t186,t1860,t1861,t1862,t1866,t1867,t1868,t1869,t187,t1870,t1871,t1872,t1873,t1874,t1875,t1876,t1877,t1878,t1879,t188,t1881,t1882,t1883,t1884,t1885,t1888,t1889,t189,t1890,t1893,t1895,t1896,t1897,t1898,t1899,t19,t1900,t1901,t1902,t1904,t1906,t1907,t191,t1911,t1913,t1917,t1919,t192,t1921,t1922,t1923,t1925,t1926,t1927,t193,t1931,t1936,t1937,t194,t1943,t1944,t1947,t1949,t195,t1950,t1952,t1953,t1954,t1955,t1956,t1957,t1958,t1959,t1962,t1964,t1965,t1966,t1967,t1970,t1971,t1973,t1974,t1975,t1976,t1977,t1978,t1980,t1981,t1982,t1983,t1984,t1985,t1986,t1987,t1988,t1990,t1991,t1992,t1993,t1994,t1997,t2,t20,t200,t2001,t2002,t2003,t2004,t2005,t2007,t2009,t201,t2010,t2014,t2015,t2017,t2018,t202,t2021,t2023,t2024,t2025,t2029,t203,t2030,t2031,t2034,t2035,t2036,t2037,t2038,t2039,t204,t2040,t2041,t2043,t2046,t2047,t2048,t2050,t2053,t2054,t2055,t2056,t2057,t2058,t2059,t206,t2061,t2063,t2064,t2065,t2066,t2067,t2068,t2069,t2070,t2072,t2073,t2075,t2077,t2078,t208,t2080,t2081,t2083,t2084,t2085,t2086,t2087,t2089,t209,t2090,t2091,t2092,t2093,t2094,t2096,t2097,t2098,t2099,t21,t210,t2106,t211,t2111,t2112,t2115,t2118,t212,t2121,t2124,t2125,t2126,t2128,t213,t2132,t2134,t2135,t2136,t2137,t2138,t2139,t214,t2140,t2141,t2144,t2145,t2148,t215,t2152,t2154,t2156,t2157,t2158,t2159,t216,t2160,t2161,t2162,t2163,t2165,t2167,t2169,t217,t2171,t2172,t2175,t2176,t2177,t2178,t2179,t218,t2180,t2181,t2182,t2183,t2184,t2185,t2186,t2187,t2188,t2189,t219,t2190,t2191,t2193,t2196,t2197,t2198,t2199,t22,t220,t2201,t2203,t2204,t2205,t2206,t2208,t221,t2212,t2213,t2214,t2215,t2216,t2217,t2219,t222,t2221,t2222,t2223,t2224,t2225,t2227,t2229,t223,t2231,t2232,t2233,t2235,t2236,t2237,t2238,t2239,t224,t2240,t2242,t2243,t2245,t2246,t2247,t2248,t2249,t225,t2250,t2251,t2252,t2253,t2254,t2256,t2258,t2259,t226,t2263,t2264,t2265,t2266,t2267,t2268,t2269,t227,t2277,t2278,t228,t2281,t2282,t2283,t2284,t2285,t2287,t2289,t229,t2290,t2292,t2293,t2296,t2297,t2299,t230,t2300,t2301,t231,t2310,t2312,t2313,t2314,t2319,t2322,t2323,t2324,t2326,t2327,t2329,t2330,t2331,t2332,t2333,t2334,t2338,t2339,t234,t2342,t2343,t2344,t235,t2356,t2357,t2358,t236,t2362,t2363,t2364,t2365,t2368,t237,t2370,t2372,t2374,t2376,t2378,t2379,t238,t2381,t2382,t2383,t2386,t2387,t239,t2390,t2392,t2394,t2395,t2396,t2397,t2398,t240,t2400,t2401,t2402,t2403,t2405,t2408,t2409,t241,t2410,t2412,t2413,t2414,t2416,t2417,t2418,t2419,t242,t2421,t2422,t2423,t2424,t2425,t2426,t2427,t2428,t2429,t243,t2430,t2431,t2432,t2433,t2436,t2437,t2438,t2439,t244,t2440,t2449,t245,t2450,t2451,t2452,t2453,t2454,t2455,t2456,t2457,t2459,t246,t2464,t2465,t2466,t2467,t2468,t2469,t247,t2470,t2471,t2472,t2473,t2474,t2475,t2476,t2477,t2478,t2479,t248,t2481,t2482,t2483,t2484,t2485,t2486,t2487,t2488,t249,t2491,t2492,t2494,t2495,t2496,t2498,t25,t250,t2504,t2508,t251,t2511,t2512,t2513,t2514,t2515,t2516,t2517,t2518,t252,t2520,t2523,t2524,t2525,t2527,t2529,t253,t2531,t2534,t2536,t2537,t2538,t2541,t2542,t2546,t2547,t2548,t255,t2550,t2552,t2553,t2554,t2555,t2556,t2559,t256,t2560,t2563,t2564,t2565,t2566,t2567,t2568,t2569,t2570,t2571,t2572,t2573,t2574,t2575,t2576,t2577,t2578,t2579,t2580,t2581,t2582,t2583,t2585,t2586,t2587,t2588,t259,t2591,t2593,t2594,t2595,t2596,t2597,t2598,t2599,t26,t260,t2600,t2601,t2602,t2603,t2604,t2605,t2607,t2608,t2609,t261,t2610,t2611,t2614,t2615,t2616,t2617,t262,t2622,t2623,t2625,t2628,t2629,t263,t2631,t2632,t2634,t2638,t2644,t2646,t2649,t265,t2650,t2652,t2659,t2660,t2661,t2665,t2666,t2667,t2668,t2669,t267,t2670,t2671,t2672,t2673,t2674,t2675,t2679,t2681,t2682,t2683,t2685,t2686,t2689,t269,t2692,t2694,t2696,t2697,t2698,t27,t2700,t2701,t2702,t2703,t2705,t2706,t2707,t2711,t2723,t2724,t2725,t2726,t2727,t2729,t2730,t2732,t2733,t2734,t2735,t2736,t2738,t2739,t274,t2740,t2741,t2742,t2744,t2745,t2746,t2747,t2748,t2749,t2751,t2752,t2753,t2754,t2755,t2756,t2757,t2758,t2759,t276,t2762,t2763,t2764,t2765,t2766,t2767,t2769,t277,t2770,t2771,t2776,t2778,t2779,t278,t2780,t2782,t2784,t2785,t2786,t2788,t279,t2792,t2793,t2795,t28,t280,t2800,t2802,t2803,t2804,t2806,t2807,t2809,t281,t2810,t2812,t2813,t2814,t2815,t2819,t2820,t2821,t2822,t2825,t2827,t2828,t2829,t283,t2830,t2832,t2833,t2834,t2836,t2839,t2842,t2843,t2844,t285,t2850,t2854,t2858,t286,t2860,t2862,t2864,t2865,t2866,t2867,t2869,t287,t2870,t2871,t2872,t2873,t2877,t288,t2880,t2882,t2883,t2885,t2887,t2888,t289,t2890,t2891,t2892,t2899,t29,t290,t2900,t2901,t2902,t2903,t2904,t2905,t2906,t2911,t2912,t2913,t2916,t2919,t292,t2921,t2922,t2923,t2924,t2925,t2926,t2927,t2928,t2929,t293,t2930,t2931,t2932,t2933,t2934,t2935,t2937,t2938,t2939,t2940,t2942,t2943,t2944,t2945,t2946,t2947,t2948,t2949,t295,t2950,t2951,t2952,t2953,t2954,t2956,t2957,t2959,t296,t2960,t2962,t2964,t2965,t2966,t2967,t2968,t297,t2970,t2973,t2975,t2977,t298,t2981,t2983,t2984,t2986,t2988,t299,t2991,t2995,t2997,t2998,t3,t300,t3002,t3003,t3004,t3006,t3007,t301,t3010,t3011,t3012,t3013,t3015,t3016,t3017,t3020,t3021,t3023,t3025,t3028,t303,t3034,t3035,t3036,t3037,t304,t3040,t3042,t3046,t3047,t3049,t305,t3051,t3052,t3053,t3054,t3056,t3057,t3058,t3059,t306,t3060,t3061,t3062,t3064,t3065,t3066,t3067,t3068,t3069,t3070,t3071,t3072,t3073,t3074,t3075,t3076,t3077,t3078,t3079,t308,t3080,t3081,t3082,t3083,t3085,t3087,t3088,t309,t3091,t3092,t3093,t3094,t3095,t3096,t3097,t3099,t3100,t3101,t3102,t3103,t3104,t3107,t3108,t3109,t311,t3110,t3111,t3112,t3118,t312,t3126,t3128,t313,t3131,t3132,t3133,t3134,t3135,t3138,t3139,t314,t3140,t3142,t3143,t3146,t3147,t3148,t315,t3156,t316,t3160,t3161,t3162,t3163,t3164,t3167,t3168,t317,t3170,t3175,t318,t3182,t3185,t3187,t3188,t3189,t319,t3190,t3192,t3193,t3196,t3197,t3198,t3199,t320,t3200,t3203,t3204,t3205,t3206,t3207,t3208,t3209,t321,t3210,t3211,t3212,t3213,t3214,t3215,t3216,t3217,t3218,t3219,t322,t3220,t3221,t3222,t3223,t3224,t3225,t3226,t3227,t3228,t323,t3230,t3231,t3232,t3234,t324,t3240,t3241,t3245,t3246,t3247,t3249,t325,t3250,t3251,t3252,t3257,t3258,t326,t3260,t3262,t3271,t3273,t3274,t3275,t3276,t3277,t3279,t328,t3283,t3284,t3286,t329,t3298,t330,t3301,t3302,t3303,t3304,t3305,t3307,t3308,t331,t3313,t3314,t3315,t332,t3322,t3323,t3324,t3326,t3327,t3328,t3329,t333,t3330,t3332,t3333,t3334,t3335,t3336,t334,t3341,t3342,t3343,t3344,t3345,t3346,t3347,t3348,t3353,t3358,t3359,t336,t3360,t3361,t3363,t337,t3370,t3373,t338,t3380,t3381,t3382,t3383,t3384,t3386,t339,t3391,t3395,t3396,t3397,t3399,t3401,t3402,t3405,t341,t3412,t3416,t3419,t342,t3421,t3422,t3425,t3427,t3429,t343,t3430,t3433,t3434,t3436,t344,t3441,t3442,t3448,t345,t3450,t3451,t3452,t3453,t3454,t3455,t3456,t3458,t3459,t346,t3462,t3463,t3465,t3466,t347,t3470,t3471,t3472,t3473,t3475,t3478,t3479,t348,t3480,t3481,t3483,t3484,t3485,t3486,t3487,t3488,t3489,t349,t3490,t3491,t3497,t3498,t350,t3501,t3504,t3505,t3506,t3507,t3511,t3512,t3519,t352,t3520,t3521,t3522,t3523,t3525,t3526,t3527,t3528,t3529,t353,t3531,t3533,t3535,t3536,t3538,t354,t3541,t3544,t3545,t3548,t3549,t355,t3554,t3555,t3557,t3559,t356,t3561,t3564,t3566,t3569,t357,t3570,t3572,t358,t3586,t3587,t3589,t3590,t3591,t3592,t3593,t3596,t3598,t360,t3605,t3608,t3609,t3610,t3611,t3612,t3613,t3614,t3615,t3616,t3617,t3627,t3628,t3629,t3630,t3632,t3634,t3635,t3636,t3637,t3638,t3639,t364,t3640,t3642,t3643,t3645,t3646,t3647,t3648,t365,t3650,t3651,t3652,t3653,t3654,t3656,t3657,t3659,t366,t3660,t3663,t3664,t3667,t3668,t367,t3671,t3678,t3679,t368,t3680,t3681,t3682,t3686,t3687,t369,t3690,t3691,t3692,t3694,t3695,t3696,t3697,t3698,t3699,t370,t3700,t3701,t3702,t3703,t3704,t3705,t3708,t371,t3711,t3712,t3713,t3714,t3716,t3717,t372,t3720,t3721,t3722,t3723,t3724,t3725,t3726,t3727,t3728,t3729,t373,t3730,t3731,t3732,t3736,t3737,t3738,t3739,t374,t3740,t3741,t3742,t3743,t3744,t3745,t3747,t3748,t3749,t375,t3750,t3751,t3758,t3759,t376,t3763,t3768,t377,t3774,t3776,t3778,t378,t3780,t3781,t3782,t379,t3793,t3795,t3796,t380,t3806,t381,t3810,t3811,t3812,t3813,t3814,t382,t3821,t3822,t3823,t3824,t3826,t3827,t3828,t3829,t383,t3837,t3838,t3839,t384,t3840,t3841,t385,t3856,t3858,t386,t3860,t3861,t3862,t3863,t3864,t3865,t3868,t3869,t387,t3871,t3872,t388,t3884,t3885,t389,t3908,t3909,t391,t3910,t392,t3928,t393,t3931,t3932,t3935,t3936,t3939,t394,t3941,t395,t3959,t396,t3960,t3962,t3964,t3966,t3967,t3968,t397,t3970,t3971,t3972,t3973,t3977,t3979,t398,t3984,t3985,t3986,t399,t3996,t3997,t3999,t4,t400,t4002,t4004,t4007,t4008,t401,t4015,t4016,t4018,t4019,t402,t4023,t4024,t4026,t4029,t403,t4031,t4032,t4033,t4034,t4035,t4036,t4038,t404,t4040,t4042,t4043,t4046,t4047,t4048,t405,t4051,t4052,t4054,t4057,t4058,t4059,t406,t4060,t4061,t4062,t4063,t4064,t4067,t4068,t4069,t407,t4072,t4073,t4074,t4075,t4077,t4078,t4079,t408,t4081,t4084,t4085,t4087,t409,t4090,t4096,t410,t4103,t4104,t4105,t4106,t4107,t4109,t411,t4113,t4115,t4116,t412,t413,t414,t415,t4152,t4153,t416,t4166,t4167,t4168,t417,t4171,t4172,t4173,t4174,t4175,t4176,t4178,t418,t4183,t4188,t419,t4198,t420,t4204,t4205,t4206,t4207,t4208,t4209,t421,t4210,t4211,t4212,t4213,t4219,t422,t4221,t423,t4230,t4231,t4232,t4233,t4234,t4235,t4236,t4237,t4238,t424,t4240,t425,t4252,t4253,t4257,t4258,t4259,t426,t4260,t4261,t4262,t4263,t4265,t4266,t427,t4272,t4274,t4275,t4276,t4277,t4279,t4280,t4281,t4284,t4285,t4287,t4288,t429,t4293,t4294,t4295,t4298,t4299,t430,t4300,t4301,t431,t4311,t4312,t4313,t4315,t432,t4322,t4327,t433,t4331,t4336,t4337,t4338,t434,t4340,t4341,t4342,t4344,t4345,t4347,t4349,t435,t4352,t4354,t436,t4361,t4364,t437,t4372,t4379,t438,t4381,t4383,t4384,t4386,t4387,t4388,t4389,t439,t4390,t4391,t4393,t4394,t440,t4403,t4405,t4406,t4407,t4409,t441,t4413,t4416,t4418,t442,t4420,t4423,t4426,t4429,t443,t4430,t4437,t4438,t444,t4440,t4441,t4442,t4443,t4445,t4446,t4449,t445,t4451,t4452,t4454,t4456,t4457,t4458,t446,t4461,t4462,t4463,t4464,t4466,t4471,t4474,t4475,t4476,t4477,t4478,t4479,t4482,t4483,t4485,t4486,t4487,t4489,t449,t4490,t4493,t4494,t4496,t4498,t450,t4501,t4503,t4504,t4506,t4507,t4508,t451,t4511,t4517,t452,t4522,t4529,t453,t4530,t4538,t4539,t454,t4542,t4543,t4544,t4545,t4546,t4547,t4557,t4558,t456,t4562,t4565,t4566,t4567,t4568,t4569,t4570,t4572,t4573,t4574,t4576,t4578,t4579,t458,t4580,t4581,t4582,t4584,t459,t4590,t460,t461,t4613,t4616,t4618,t4619,t4624,t4626,t4627,t4628,t4629,t463,t4631,t4632,t4639,t464,t465,t466,t4664,t467,t4673,t4674,t4675,t4676,t468,t4685,t4686,t469,t4694,t470,t4702,t4705,t471,t4711,t4713,t4714,t4715,t4718,t472,t4723,t4724,t4725,t473,t4734,t4737,t4739,t474,t4740,t4742,t4743,t4744,t4746,t4747,t4749,t475,t4751,t4755,t4756,t4758,t4759,t4760,t4762,t4763,t4764,t4765,t4766,t4767,t4768,t4769,t477,t4770,t4771,t4772,t4773,t4774,t4775,t4776,t4778,t478,t479,t4790,t48,t480,t4800,t4804,t4805,t4806,t4807,t4808,t4809,t481,t4810,t4813,t4815,t482,t4821,t4823,t4824,t4825,t483,t4830,t4831,t4832,t4833,t484,t4842,t4855,t4856,t4857,t4858,t4859,t486,t4860,t4864,t4865,t487,t4870,t4872,t4875,t4876,t488,t4882,t4883,t489,t4894,t4895,t4896,t4898,t49,t490,t4903,t4905,t4906,t4907,t4908,t4909,t491,t4910,t4911,t4919,t492,t4931,t4935,t4936,t4937,t4938,t494,t4940,t4957,t4958,t496,t4967,t497,t4971,t4975,t498,t499,t5,t50,t500,t5000,t5002,t5003,t5004,t5005,t501,t502,t5020,t5032,t5034,t5039,t504,t5040,t5041,t5042,t505,t5052,t5053,t5054,t5055,t506,t5067,t5068,t5069,t507,t5070,t5071,t5073,t5074,t5077,t508,t5080,t5081,t5082,t5086,t5087,t509,t5090,t5091,t51,t510,t5100,t5101,t5105,t511,t512,t5120,t5123,t5124,t5125,t5126,t5127,t5129,t5132,t5136,t5137,t5138,t5139,t514,t5141,t5143,t5145,t5146,t515,t5155,t5157,t516,t517,t5171,t5172,t5173,t5176,t5179,t518,t5186,t5187,t5188,t519,t52,t520,t5204,t5205,t5209,t521,t5210,t5211,t5213,t5219,t522,t5222,t5223,t5226,t5227,t5228,t5229,t523,t5233,t5234,t5235,t524,t5248,t5249,t5250,t5253,t5257,t5258,t5259,t5263,t5264,t5266,t5269,t527,t5271,t5274,t5276,t5278,t5279,t528,t5280,t5281,t5282,t5284,t5288,t529,t5296,t5297,t5299,t53,t530,t5300,t5301,t5302,t5303,t5304,t531,t5311,t5313,t5314,t5315,t5317,t5320,t5322,t5333,t5339,t534,t5342,t5343,t5344,t535,t5354,t5355,t5356,t5357,t5358,t5359,t536,t5360,t5361,t5363,t5365,t5370,t5387,t5389,t539,t5393,t5394,t5395,t5399,t54,t540,t5400,t5401,t5407,t5410,t5411,t5414,t5417,t5418,t542,t543,t545,t5453,t5455,t546,t547,t5474,t548,t5480,t5481,t5482,t5483,t5484,t5487,t5488,t549,t5491,t5492,t5495,t5497,t5498,t55,t550,t5500,t5501,t5502,t5505,t5507,t5508,t5509,t551,t5512,t5517,t5518,t552,t5520,t5521,t553,t5530,t5536,t5537,t5538,t554,t5543,t5548,t5549,t555,t5550,t5551,t5552,t5553,t5554,t5556,t5557,t5559,t556,t557,t558,t5589,t559,t5590,t5592,t5593,t5599,t56,t560,t5600,t5604,t5605,t5606,t5607,t5608,t561,t5612,t5613,t5614,t5615,t5616,t5618,t562,t563,t5634,t5636,t5638,t5639,t5648,t565,t5652,t566,t5663,t5665,t5668,t5669,t567,t569,t57,t5711,t5712,t5715,t5719,t5720,t5726,t5727,t5728,t5729,t5731,t5734,t5735,t5736,t5738,t5739,t574,t5761,t5762,t5766,t5767,t5768,t5771,t5773,t5776,t578,t5783,t5785,t5786,t5787,t5788,t579,t58,t5808,t581,t5810,t582,t5831,t5832,t584,t5843,t5844,t585,t5852,t5853,t5854,t5859,t587,t5884,t5886,t589,t5894,t5897,t5898,t59,t590,t5900,t5901,t5902,t5903,t5904,t591,t5916,t5917,t592,t5928,t5933,t5934,t5938,t5939,t594,t5940,t5949,t595,t596,t597,t598,t5981,t5984,t5988,t5989,t599,t5992,t5993,t5994,t5997,t6,t60,t600,t6002,t6003,t6004,t6005,t6006,t6008,t6009,t601,t6019,t602,t6020,t6021,t6023,t6024,t6025,t6026,t6028,t604,t6047,t6048,t605,t6052,t6054,t6055,t6057,t6058,t6059,t606,t6062,t6063,t6072,t608,t6088,t6089,t609,t6090,t6096,t6097,t61,t610,t6103,t6106,t6107,t611,t6113,t6116,t6118,t6119,t6124,t6126,t6128,t6129,t613,t6131,t6132,t6133,t614,t6147,t6148,t6153,t6157,t6159,t616,t6160,t6162,t617,t618,t6183,t6184,t6187,t619,t6191,t6192,t62,t620,t6212,t6213,t6216,t6218,t6219,t622,t6225,t6227,t6228,t6229,t623,t6231,t624,t625,t626,t627,t629,t6294,t6295,t6296,t63,t630,t631,t6314,t6315,t6316,t632,t6329,t633,t6335,t6336,t6337,t6338,t6339,t634,t635,t6353,t636,t637,t6370,t638,t6381,t6387,t6389,t639,t6392,t6395,t6396,t6397,t640,t641,t6422,t643,t6438,t6439,t644,t6440,t6441,t645,t6453,t6468,t6469,t647,t6473,t648,t6484,t649,t6499,t650,t6503,t6509,t651,t6515,t652,t6521,t6524,t6529,t653,t6532,t654,t655,t656,t657,t658,t6583,t6584,t659,t6598,t66,t660,t661,t6618,t6619,t662,t6628,t6629,t663,t664,t666,t6669,t667,t6670,t6680,t6681,t669,t67,t670,t6734,t6735,t6736,t674,t6742,t6743,t6744,t675,t6750,t6754,t6755,t676,t677,t6772,t678,t679,t680,t681,t683,t684,t685,t686,t687,t688,t689,t690,t691,t692,t693,t696,t699,t7,t700,t702,t703,t704,t705,t706,t707,t708,t709,t710,t711,t712,t713,t715,t716,t717,t719,t720,t721,t722,t723,t724,t725,t726,t728,t729,t731,t732,t734,t737,t738,t742,t744,t748,t750,t751,t754,t756,t758,t759,t761,t763,t766,t767,t768,t769,t770,t773,t774,t775,t776,t781,t782,t784,t785,t788,t789,t790,t793,t795,t796,t798,t799,t8,t800,t803,t805,t807,t808,t809,t81,t814,t815,t816,t817,t819,t820,t821,t822,t823,t824,t826,t828,t829,t831,t832,t833,t834,t835,t837,t838,t839,t84,t842,t844,t847,t848,t849,t85,t850,t851,t852,t853,t854,t858,t859,t86,t861,t863,t864,t867,t868,t87,t871,t872,t875,t879,t880,t883,t884,t885,t886,t888,t89,t890,t891,t894,t895,t896,t897,t898,t899,t9,t90,t900,t902,t905,t906,t907,t908,t909,t910,t911,t912,t913,t914,t915,t916,t918,t919,t92,t920,t921,t923,t926,t928,t929,t93,t930,t931,t933,t934,t935,t936,t937,t938,t944,t945,t946,t947,t948,t949,t95,t950,t951,t954,t955,t956,t957,t958,t959,t96,t960,t961,t962,t963,t964,t965,t966,t967,t968,t969,t97,t970,t972,t973,t974,t975,t976,t977,t978,t98,t981,t982,t984,t986,t987,t988,t99,t990,t991,t992,t993,t994,t996,t997,t999] = ct{:};
t730 = t8.*t383;
t733 = t12.*t375;
t735 = t6.*t401;
t736 = t6.*t402;
t740 = t6.*t405;
t743 = t8.*t385;
t745 = t12.*t379;
t746 = t6.*t414;
t747 = t6.*t415;
t752 = t9.*t386;
t757 = t10.*t388;
t772 = t200./1.0e+1;
t777 = t8.*t417;
t780 = t12.*t397;
t783 = t6.*t450;
t794 = t6.*t454;
t797 = t12.*t404;
t801 = t12.*t405;
t802 = t6.*t459;
t812 = t6.*t469;
t813 = t12.*t418;
t827 = t12.*t438;
t836 = -t560;
t857 = t12.*t451;
t860 = t6.*t315;
t862 = t12.*t454;
t865 = t12.*t456;
t870 = t12.*t461;
t874 = t6.*t317;
t876 = t12.*t469;
t877 = t12.*t471;
t889 = t11.*t492;
t892 = -t599;
t893 = -t600;
t901 = -t604;
t903 = -t608;
t904 = -t609;
t917 = -t613;
t924 = t12.*t316;
t927 = t12.*t320;
t932 = -t644;
t940 = -t647;
t941 = -t648;
t943 = -t653;
t952 = -t654;
t953 = -t655;
t1024 = -t754;
t1026 = -t756;
t1032 = t10.*t558;
t1038 = t11.*t560;
t1046 = -t775;
t1057 = -t799;
t1066 = -t814;
t1069 = -t821;
t1070 = -t822;
t1071 = -t824;
t1075 = -t831;
t1079 = t10.*t599;
t1097 = -t837;
t1109 = -t872;
t1115 = -t886;
t1118 = -t891;
t1126 = -t895;
t1128 = -t906;
t1129 = -t908;
t1130 = -t910;
t1139 = -t920;
t1142 = -t923;
t1150 = -t935;
t1152 = -t945;
t1153 = -t946;
t1155 = -t948;
t1156 = -t949;
t1157 = -t951;
t1174 = t3.*t669;
t1179 = t19.*t438;
t1181 = t18.*t442;
t1187 = t20.*t442;
t1206 = t12.*t674;
t1250 = t52+t218;
t1251 = t53+t217;
t1252 = t54+t222;
t1253 = t55+t221;
t1257 = t48.*t424;
t1258 = t52.*t383;
t1259 = t48.*t426;
t1260 = t48.*t431;
t1261 = t52.*t385;
t1262 = t48.*t432;
t1270 = t48.*t483;
t1272 = t51.*t451;
t1273 = t58.*t400;
t1274 = t9.*t738;
t1278 = t48.*t489;
t1280 = t51.*t461;
t1281 = t58.*t410;
t1284 = t54.*t434;
t1285 = t62.*t386;
t1290 = t49.*t501;
t1300 = t48.*t324;
t1301 = t52.*t481;
t1302 = t52.*t483;
t1306 = t51.*t315;
t1307 = t58.*t453;
t1308 = t48.*t326;
t1309 = t52.*t488;
t1310 = t52.*t489;
t1313 = t12.*t788;
t1314 = t51.*t317;
t1315 = t58.*t465;
t1318 = t55.*t501;
t1336 = t52.*t324;
t1338 = t59.*t481;
t1339 = t58.*t315;
t1340 = t52.*t326;
t1342 = t59.*t488;
t1343 = t58.*t317;
t1344 = t9.*t885;
t1351 = -t1082;
t1354 = -t1087;
t1360 = t9.*t898;
t1364 = -t1088;
t1365 = -t1091;
t1368 = t9.*t907;
t1378 = t11.*t910;
t1389 = t9.*t934;
t1394 = t9.*t949;
t1396 = -t1135;
t1405 = -t1161;
t1411 = -t1166;
t1412 = -t1167;
t1414 = t19.*t559;
t1415 = t18.*t560;
t1420 = -t1176;
t1421 = -t1177;
t1422 = -t1178;
t1428 = t19.*t602;
t1430 = t20.*t600;
t1431 = t20.*t601;
t1439 = -t1193;
t1440 = -t1194;
t1444 = t19.*t641;
t1446 = t27.*t600;
t1448 = t27.*t601;
t1455 = t20.*t648;
t1459 = -t1216;
t1460 = t27.*t647;
t1461 = t27.*t648;
t1492 = t49.*t601;
t1507 = -t1283;
t1508 = -t1286;
t1510 = -t1288;
t1512 = t11.*t12.*t557;
t1516 = t54.*t605;
t1517 = t9.*t1035;
t1518 = t49.*t653;
t1519 = t60.*t560;
t1520 = t6.*t687;
t1521 = t6.*t688;
t1522 = t6.*t689;
t1542 = -t1320;
t1543 = t12.*t1072;
t1547 = t9.*t1081;
t1548 = t49.*t510;
t1549 = t50.*t509;
t1551 = t12.*t687;
t1552 = t12.*t688;
t1553 = t12.*t689;
t1559 = -t1334;
t1560 = -t1335;
t1572 = -t1355;
t1573 = -t1358;
t1577 = -t1369;
t1578 = -t1370;
t1579 = -t1371;
t1580 = -t1372;
t1583 = -t1375;
t1594 = -t1393;
t1596 = t9.*t1159;
t1615 = -t1404;
t1616 = -t1407;
t1636 = t10.*t27.*t386;
t1639 = t26.*t754;
t1641 = t18.*t823;
t1642 = t6.*t1192;
t1644 = t9.*t1182;
t1645 = t9.*t1183;
t1646 = t9.*t20.*t439;
t1647 = t5.*t18.*t501;
t1652 = -t1409;
t1653 = -t1410;
t1658 = t9.*t27.*t439;
t1659 = t5.*t25.*t501;
t1672 = t20.*t895;
t1678 = t20.*t907;
t1679 = t20.*t908;
t1680 = t18.*t911;
t1687 = -t1447;
t1693 = t20.*t934;
t1694 = t20.*t935;
t1707 = t20.*t657;
t1710 = t18.*t661;
t1735 = t56.*t822;
t1744 = t123.*t498;
t1745 = t60.*t826;
t1751 = t9.*t1327;
t1762 = -t1544;
t1771 = t9.*t1371;
t1777 = t193.*1.35e-3;
t1783 = -t1589;
t1788 = -t1608;
t1789 = -t1610;
t1790 = -t1611;
t1791 = -t1612;
t1793 = -t1614;
t1795 = t10.*t20.*t386;
t1807 = -t1624;
t1809 = -t1627;
t1810 = -t1628;
t1811 = -t1630;
t1812 = -t1631;
t1813 = -t1633;
t1814 = -t1634;
t1825 = t18.*t1084;
t1826 = t18.*t1086;
t1835 = -t1654;
t1836 = -t1657;
t1841 = t5.*t18.*t510;
t1842 = t27.*t1083;
t1843 = t27.*t1085;
t1848 = -t1676;
t1856 = -t1695;
t1863 = t3.*t1482;
t1864 = t4.*t1483;
t1865 = t5.*t1484;
t1903 = t18.*t987;
t1905 = -t1736;
t1908 = t86.*t557;
t1909 = t123.*t601;
t1912 = t56.*t1081;
t1914 = t11.*t1524;
t1920 = -t1742;
t1933 = -t1765;
t1934 = -t1766;
t1935 = -t1767;
t1960 = -t1780;
t1961 = -t1782;
t1972 = t200.*1.0675e-2;
t1996 = t18.*t1037;
t1998 = -t1815;
t2000 = t20.*t1349;
t2012 = t61.*t1210;
t2013 = t19.*t1375;
t2016 = -t1838;
t2020 = t27.*t1353;
t2026 = t102+t364;
t2028 = t109+t367;
t2032 = t119+t391;
t2033 = t120+t392;
t2045 = t18.*t1188;
t2074 = t61.*t1299;
t2079 = t9.*t1749;
t2088 = -t1923;
t2100 = -t1970;
t2102 = -t1974;
t2103 = -t1975;
t2104 = -t1976;
t2105 = -t1977;
t2107 = t18.*t1289;
t2109 = t18.*t1293;
t2110 = t18.*t1296;
t2113 = -t1981;
t2114 = -t1982;
t2116 = t9.*t1637;
t2117 = t18.*t1316;
t2123 = -t1991;
t2127 = t20.*t1329;
t2133 = -t2007;
t2149 = t50.*t1484;
t2151 = t5.*t1868;
t2168 = t55.*t1484;
t2200 = t3.*t19.*t978;
t2202 = t3.*t6.*t1526;
t2220 = t6.*t1704;
t2228 = -t2073;
t2230 = t12.*t1704;
t2234 = -t2081;
t2262 = t6.*t1964;
t2276 = (t6.*t690)./1.0e+1;
t2279 = t20.*t1482;
t2280 = t21.*t1483;
t2295 = t5.*t1980;
t2308 = (t12.*t690)./1.0e+1;
t2318 = -t2106;
t2320 = t20.*t1524;
t2325 = -t2128;
t2335 = -t2156;
t2336 = -t2157;
t2337 = -t2160;
t2345 = -t2175;
t2346 = -t2177;
t2347 = -t2178;
t2348 = -t2181;
t2349 = -t2182;
t2350 = -t2183;
t2351 = -t2185;
t2352 = -t2186;
t2359 = t5.*t2054;
t2360 = -t2190;
t2373 = t5.*t2067;
t2375 = t5.*t2069;
t2384 = -t2196;
t2385 = -t2198;
t2404 = t11.*t2069;
t2406 = t13.*t2067;
t2407 = t13.*t2068;
t2411 = -t2205;
t2415 = t26.*t1669;
t2420 = t12.*t2077;
t2434 = -t2249;
t2435 = -t2251;
t2441 = -t2264;
t2442 = -t2265;
t2443 = -t2266;
t2444 = -t2267;
t2458 = -t2297;
t2460 = -t2299;
t2461 = -t2300;
t2480 = t18.*t1759;
t2499 = t60.*t1860;
t2500 = t62.*t1860;
t2501 = t112.*t1484;
t2502 = t54.*t1868;
t2506 = t5.*t2171;
t2507 = t6.*t2169;
t2509 = t19.*t1964;
t2510 = t20.*t1966;
t2533 = t20.*t1982;
t2543 = t6.*t2199;
t2549 = t10.*t2199;
t2551 = t12.*t2199;
t2562 = t10.*t2205;
t2613 = t48.*t1952;
t2618 = t21.*t1859;
t2647 = t18.*t1868;
t2651 = t20.*t1868;
t2653 = t20.*t1871;
t2655 = t20.*t1874;
t2656 = t20.*t1875;
t2657 = t21.*t1874;
t2658 = t21.*t1875;
t2662 = t21.*t1879;
t2677 = t6.*t2289;
t2680 = t58.*t1964;
t2688 = t20.*t1885;
t2691 = t27.*t1875;
t2695 = t28.*t1879;
t2743 = t1006.*(9.0./8.0e+2);
t2760 = t21.*t1958;
t2761 = -t2492;
t2772 = -t2515;
t2773 = -t2516;
t2775 = t7.*t2356;
t2781 = -t2523;
t2783 = -t2527;
t2787 = -t2534;
t2789 = -t2536;
t2790 = -t2538;
t2794 = t12.*t2356;
t2796 = t7.*t2365;
t2798 = t13.*t2356;
t2801 = t10.*t2358;
t2808 = t13.*t2358;
t2816 = t4.*t2386;
t2817 = t5.*t2386;
t2818 = t6.*t2386;
t2826 = t13.*t2365;
t2837 = t54.*t2069;
t2840 = t5.*t2397;
t2845 = t7.*t2392;
t2849 = t5.*t12.*t2068;
t2851 = t13.*t2374;
t2852 = t13.*t2376;
t2855 = -t2547;
t2856 = -t2548;
t2857 = -t2550;
t2859 = t10.*t2386;
t2861 = t11.*t2386;
t2863 = t12.*t2386;
t2878 = t13.*t2390;
t2884 = t13.*t2397;
t2889 = -t2563;
t2893 = -t2573;
t2894 = -t2575;
t2895 = -t2576;
t2896 = -t2577;
t2898 = -t2579;
t2910 = -t2605;
t2914 = -t2616;
t2915 = -t2617;
t2917 = -t2622;
t2918 = -t2623;
t2941 = -t2666;
t2955 = -t2696;
t2969 = -t2711;
t2985 = t3.*t2475;
t2987 = t18.*t2067;
t2989 = t19.*t2068;
t2990 = t5.*t2477;
t2992 = t20.*t2067;
t2993 = t10.*t2468;
t2996 = t22.*t2067;
t3000 = t6.*t1006.*(9.0./3.2e+2);
t3008 = -t2723;
t3009 = -t2724;
t3018 = -t2744;
t3019 = -t2745;
t3022 = -t2751;
t3024 = -t2758;
t3029 = t57.*t2199;
t3030 = t58.*t2199;
t3031 = t5.*t2550;
t3039 = t5.*t11.*t2205;
t3041 = t9.*t2548;
t3043 = t62.*t2199;
t3050 = t13.*t2554;
t3063 = t11.*t2563;
t3089 = -t2858;
t3090 = -t2862;
t3098 = t13.*t2596;
t3106 = t21.*t2138;
t3116 = t21.*t2144;
t3121 = t109.*t1958;
t3125 = t6.*t2650;
t3129 = t28.*t2138;
t3130 = -t2913;
t3136 = t49.*t2287;
t3153 = t6.*t12.*t19.*t1484;
t3154 = t21.*t2169;
t3159 = t21.*t2179;
t3171 = t28.*t56.*t1483;
t3173 = t28.*t2178;
t3174 = t28.*t2179;
t3177 = t3.*t19.*t1895;
t3183 = t18.*t2199;
t3184 = t20.*t2199;
t3186 = t20.*t2205;
t3194 = t158+t1255;
t3195 = -t2970;
t3233 = t9.*t2734;
t3236 = t3.*t1006.*5.625e-3;
t3237 = t4.*t1006.*5.625e-3;
t3238 = t5.*t1006.*5.625e-3;
t3239 = t6.*t1006.*5.625e-3;
t3265 = t3.*t19.*t1959;
t3267 = t21.*t2243;
t3269 = t21.*t2245;
t3270 = t21.*t2246;
t3278 = t21.*t2251;
t3280 = t49.*t56.*t1482;
t3281 = t56.*t2148;
t3282 = t20.*t2252;
t3287 = t12.*t99.*t1484;
t3288 = t21.*t2258;
t3290 = t21.*t2264;
t3291 = t21.*t2265;
t3296 = t26.*t2245;
t3297 = t27.*t2247;
t3300 = t2.*t2523;
t3306 = t19.*t2289;
t3312 = t50.*t2188;
t3316 = t25.*t2292;
t3317 = t3.*t4.*t2199;
t3318 = t51.*t2199;
t3331 = t5.*t63.*t1965;
t3339 = t7.*t13.*t2364;
t3362 = t9.*t2815;
t3364 = t12.*t2815;
t3365 = t3.*t2858;
t3368 = t54.*t2386;
t3369 = t55.*t2386;
t3371 = t56.*t2386;
t3374 = t57.*t2386;
t3377 = t6.*t2860;
t3385 = t6.*t2864;
t3387 = t6.*t2865;
t3394 = t22.*t2474;
t3406 = t7.*t2870;
t3410 = t111.*t2077;
t3411 = t62.*t2368;
t3413 = t112.*t2077;
t3414 = t127.*t2068;
t3418 = t54.*t2408;
t3426 = -t3040;
t3428 = -t3042;
t3432 = t9.*t2858;
t3435 = t60.*t2386;
t3437 = t10.*t2860;
t3438 = t9.*t2862;
t3440 = t61.*t2386;
